simulink model "FeedBack_Linearization"  (R2021b)
settings: Solver=VariableStepAuto  StartTime=0.0  StopTime=10.0  RelTol=1e-3
undefined symbols (not defined in the file): Kd, Kp, q_dq_init
(part 4 of 9)

== matlab function FeedBack_Linearization/C ==
  data: q input; C output; dq input
function C = C_fun(q,dq)
%C_fun
%    C = C_fun(Q1,Q2,Q3,Q4,Q5,Q6,Q7,DQ1,DQ2,DQ3,DQ4,DQ5,DQ6,DQ7)

%    This function was generated by the Symbolic Math Toolbox version 9.0.
%    15-Apr-2022 03:00:29

q1 = q(1);
q2 = q(2);
q3 = q(3);
q4 = q(4);
q5 = q(5);
q6 = q(6);
q7 = q(7);

dq1 = dq(1);
dq2 = dq(2);
dq3 = dq(3);
dq4 = dq(4);
dq5 = dq(5);
dq6 = dq(6);
dq7 = dq(7);

t2 = cos(q1);
t3 = cos(q2);
t4 = cos(q3);
t5 = cos(q4);
t6 = cos(q5);
t7 = cos(q6);
t8 = cos(q7);
t9 = sin(q1);
t10 = sin(q2);
t11 = sin(q3);
t12 = sin(q4);
t13 = sin(q5);
t14 = sin(q6);
t15 = sin(q7);
t16 = dq1.^2;
t17 = dq2.^2;
t18 = dq3.^2;
t19 = dq4.^2;
t20 = dq5.^2;
t21 = dq6.^2;
t22 = dq7.^2;
t1002 = atan(4.601355810186573e-2);
t1005 = atan(4.558404558404559e-1);
t1006 = atan(2.19375);
t23 = t2.^2;
t24 = t3.^2;
t25 = t4.^2;
t26 = t9.^2;
t27 = t10.^2;
t28 = t11.^2;
t29 = t2.*t4;
t30 = t3.*t5;
t31 = t2.*t11;
t32 = t4.*t9;
t33 = t3.*t12;
t34 = t5.*t10;
t35 = t9.*t11;
t36 = t10.*t12;
t37 = dq1.*t2.*t3;
t39 = dq2.*t2.*t3;
t40 = dq2.*t3.*t4;
t43 = dq3.*t3.*t4;
t45 = dq1.*t2.*t10;
t46 = dq1.*t3.*t9;
t49 = dq2.*t2.*t10;
t50 = dq2.*t3.*t9;
t51 = dq2.*t3.*t11;
t52 = dq2.*t4.*t10;
t57 = dq3.*t3.*t11;
t58 = dq3.*t4.*t10;
t61 = dq1.*t9.*t10;
t63 = dq2.*t9.*t10;
t64 = dq2.*t10.*t11;
t67 = dq3.*t10.*t11;
t71 = t10.*t11.*t13;
t72 = dq2.*t3.*t10.*2.0;
t83 = t3.*t6.*t11;
t84 = t4.*t6.*t10;
t90 = t3.*t11.*t13;
t91 = t4.*t10.*t13;
t92 = t6.*t10.*t11;
t105 = t10.*(2.1e+1./5.0e+1);
t192 = t2.*t3.*t16;
t194 = t2.*t3.*t17;
t202 = t2.*t10.*t16;
t203 = t3.*t9.*t16;
t206 = t2.*t10.*t17;
t207 = t3.*t9.*t17;
t209 = t4.*t10.*t17;
t213 = t4.*t10.*t18;
t221 = t9.*t10.*t16;
t223 = t9.*t10.*t17;
t224 = t10.*t11.*t17;
t226 = t10.*t11.*t18;
t248 = t3.*t10.*t17.*2.0;
t267 = t2.*t3.*(2.1e+1./5.0e+1);
t272 = t3.*t9.*(2.1e+1./5.0e+1);
t358 = dq2.*t10.*(-2.1e+1./5.0e+1);
t496 = t3.*t17.*(2.1e+1./5.0e+1);
t1021 = q2+t1002;
t1026 = q1+t1006;
t1037 = -t1005;
t1107 = t2.*t16.*3.55e-3;
t1108 = t9.*t16.*3.55e-3;
t1403 = t3.*t17.*3.9348e-1;
t1717 = dq2.*t3.*t10.*2.32304589786736e-19;
t1723 = dq2.*t3.*t10.*1.781996172844913e-20;
t2010 = dq2.*t3.*t10.*8.400000000000278e-4;
t38 = dq1.*t29;
t41 = dq3.*t29;
t42 = dq2.*t30;
t44 = dq4.*t30;
t47 = dq1.*t31;
t48 = dq1.*t32;
t53 = dq3.*t31;
t54 = dq3.*t32;
t55 = dq2.*t33;
t56 = dq2.*t34;
t59 = dq4.*t33;
t60 = dq4.*t34;
t62 = dq1.*t35;
t65 = dq3.*t35;
t66 = dq2.*t36;
t68 = dq4.*t36;
t69 = dq2.*t24;
t70 = t9.*t36;
t73 = t3.*t29;
t74 = t2.*t30;
t75 = t4.*t30;
t76 = t3.*t31;
t77 = t3.*t32;
t78 = t2.*t33;
t79 = t2.*t34;
t80 = t9.*t30;
t81 = t4.*t33;
t82 = t4.*t34;
t85 = t3.*t35;
t86 = t2.*t36;
t87 = t9.*t33;
t88 = t9.*t34;
t89 = t4.*t36;
t93 = t33.*(2.0./5.0);
t94 = t34.*(2.0./5.0);
t102 = t6.*t40;
t103 = t6.*t43;
t113 = dq2.*t10.*t29;
t127 = t13.*t40;
t128 = t6.*t51;
t129 = dq3.*t11.*t30;
t131 = t13.*t43;
t132 = t6.*t58;
t135 = dq5.*t83;
t136 = dq5.*t84;
t143 = dq2.*t10.*t31;
t145 = dq2.*t10.*t32;
t157 = t13.*t51;
t158 = t6.*t64;
t159 = dq3.*t11.*t33;
t161 = dq3.*t11.*t34;
t162 = t13.*t58;
t163 = t6.*t67;
t166 = dq5.*t90;
t167 = dq5.*t91;
t168 = dq5.*t92;
t173 = dq2.*t10.*t35;
t177 = t13.*t64;
t178 = dq3.*t11.*t36;
t179 = t13.*t67;
t181 = dq5.*t71;
t182 = -t72;
t185 = -t61;
t186 = -t63;
t187 = -t64;
t189 = -t67;
t191 = dq1.*t3.*t23;
t193 = t16.*t29;
t195 = t18.*t29;
t196 = t17.*t30;
t197 = t19.*t30;
t198 = dq2.*t37.*2.0;
t200 = dq3.*t40.*2.0;
t201 = dq1.*t3.*t26;
t204 = t16.*t31;
t205 = t16.*t32;
t208 = dq2.*t4.*t27;
t210 = t18.*t31;
t211 = t18.*t32;
t212 = t17.*t33;
t214 = t19.*t33;
t215 = dq2.*t45.*2.0;
t216 = dq2.*t46.*2.0;
t219 = dq3.*t51.*2.0;
t222 = t16.*t35;
t225 = t18.*t35;
t227 = dq2.*t61.*2.0;
t231 = dq1.*dq2.*t10.*t23;
t232 = dq1.*dq2.*t10.*t26;
t233 = dq2.*dq3.*t11.*t27;
t234 = t10.*t40.*2.0;
t239 = dq2.*t105;
t240 = t29.*t34;
t241 = t29.*t36;
t242 = t32.*t34;
t243 = t6.*t10.*t31;
t244 = t6.*t11.*t34;
t250 = t32.*t36;
t251 = t10.*t13.*t31;
t252 = t6.*t10.*t35;
t253 = t11.*t13.*t34;
t254 = t7.*t11.*t36;
t258 = t10.*t13.*t35;
t259 = t11.*t14.*t36;
t265 = -t90;
t266 = -t92;
t269 = t11.*t36.*(2.0./5.0);
t271 = t2.*t105;
t281 = t9.*t105;
t395 = t17.*t92;
t397 = t18.*t92;
t399 = t20.*t92;
t418 = t17.*t71;
t419 = t18.*t71;
t420 = t20.*t71;
t459 = t37.*(2.1e+1./5.0e+1);
t460 = t39.*(2.1e+1./5.0e+1);
t464 = t45.*(2.1e+1./5.0e+1);
t465 = t46.*(2.1e+1./5.0e+1);
t466 = t49.*(2.1e+1./5.0e+1);
t467 = t50.*(2.1e+1./5.0e+1);
t468 = t61.*(2.1e+1./5.0e+1);
t469 = t63.*(2.1e+1./5.0e+1);
t475 = t3.*t209.*2.0;
t554 = dq2.*t37.*(2.1e+1./2.5e+1);
t557 = dq2.*t46.*(2.1e+1./2.5e+1);
t558 = -t496;
t567 = t45+t50;
t568 = t46+t49;
t569 = t51+t58;
t570 = t52+t57;
t1058 = q1+t1037;
t1171 = -t1108;
t1192 = dq2.*t37.*3.3338e-1;
t1196 = dq2.*t46.*3.3338e-1;
t1235 = dq3.*t51.*4.5e-3;
t1251 = t202.*1.6669e-1;
t1252 = t206.*1.6669e-1;
t1254 = t221.*1.6669e-1;
t1255 = t223.*1.6669e-1;
t1261 = dq3.*t40.*7.635999999999999e-2;
t1262 = dq3.*t40.*6.984e-2;
t1279 = t209.*2.25e-3;
t1281 = t213.*2.25e-3;
t1282 = dq2.*t45.*1.534e-2;
t1285 = dq2.*t61.*1.534e-2;
t1323 = t224.*3.492e-2;
t1324 = t226.*3.492e-2;
t1396 = t224.*3.818e-2;
t1397 = t226.*3.818e-2;
t1404 = t192.*7.669999999999999e-3;
t1405 = t194.*7.669999999999999e-3;
t1407 = t203.*7.669999999999999e-3;
t1408 = t207.*7.669999999999999e-3;
t1457 = dq2.*t37.*7.8696e-1;
t1461 = dq2.*t46.*7.8696e-1;
t1533 = t202.*3.9348e-1;
t1534 = t206.*3.9348e-1;
t1535 = t221.*3.9348e-1;
t1536 = t223.*3.9348e-1;
t1736 = -t1717;
t1751 = -t1723;
t1980 = t10.*t40.*1.400000000000004e-4;
t2007 = t3.*t209.*1.400000000000004e-4;
t2009 = t10.*t40.*9.999999999999995e-5;
t2018 = -t2010;
t2023 = t3.*t209.*9.999999999999995e-5;
t2048 = t10.*t40.*4.380000000000001e-3;
t2097 = t3.*t209.*4.380000000000001e-3;
t95 = t3.*t38;
t96 = dq1.*t74;
t97 = dq2.*t73;
t98 = t2.*t42;
t99 = t3.*t41;
t100 = t4.*t42;
t101 = t2.*t44;
t104 = t4.*t44;
t106 = t3.*t47;
t107 = t10.*t38;
t108 = t3.*t48;
t109 = dq1.*t78;
t110 = dq1.*t79;
t111 = dq1.*t80;
t112 = dq2.*t76;
t114 = dq2.*t77;
t115 = t2.*t55;
t116 = t2.*t56;
t117 = t9.*t42;
t118 = t3.*t53;
t119 = t10.*t41;
t120 = t3.*t54;
t121 = t4.*t55;
t122 = t11.*t42;
t123 = t4.*t56;
t124 = t2.*t59;
t125 = t2.*t60;
t126 = t9.*t44;
t130 = dq3.*t82;
t133 = t4.*t59;
t134 = t4.*t60;
t137 = t10.*t47;
t138 = t3.*t62;
t139 = t10.*t48;
t140 = dq1.*t86;
t141 = dq1.*t87;
t142 = dq1.*t88;
t144 = dq2.*t85;
t146 = t2.*t66;
t147 = t9.*t55;
t148 = t9.*t56;
t149 = t10.*t53;
t150 = t3.*t65;
t151 = t10.*t54;
t152 = t11.*t55;
t153 = t4.*t66;
t154 = t2.*t68;
t155 = t9.*t59;
t156 = t9.*t60;
t160 = dq3.*t89;
t164 = t4.*t68;
t165 = t11.*t60;
t169 = -t38;
t170 = -t41;
t171 = t10.*t62;
t172 = dq1.*t70;
t174 = t9.*t66;
t175 = t10.*t65;
t176 = t9.*t68;
t180 = t11.*t68;
t183 = -t55;
t184 = -t60;
t188 = -t66;
t190 = -t68;
t199 = dq3.*t38.*2.0;
t217 = dq3.*t47.*2.0;
t218 = dq3.*t48.*2.0;
t220 = dq4.*t56.*2.0;
t228 = dq3.*t62.*2.0;
t229 = dq4.*t66.*2.0;
t230 = -t93;
t235 = t44.*(2.0./5.0);
t236 = t56.*(2.0./5.0);
t237 = t59.*(2.0./5.0);
t238 = t66.*(2.0./5.0);
t245 = -t198;
t247 = -t200;
t249 = -t73;
t256 = -t81;
t257 = -t82;
t260 = -t227;
t262 = -t85;
t263 = -t86;
t264 = -t88;
t268 = t70.*(2.0./5.0);
t270 = t29.*t42;
t273 = t34.*t38;
t274 = t29.*t55;
t275 = t32.*t42;
t278 = t29.*t60;
t282 = t36.*t38;
t283 = t34.*t48;
t285 = t32.*t55;
t288 = t34.*t53;
t291 = t29.*t68;
t292 = t32.*t60;
t294 = dq5.*t243;
t299 = dq5.*t244;
t304 = -t102;
t305 = -t103;
t307 = t36.*t48;
t311 = t36.*t53;
t312 = t34.*t65;
t314 = t32.*t68;
t315 = dq5.*t251;
t316 = dq5.*t252;
t321 = dq5.*t253;
t322 = dq6.*t254;
t324 = -t128;
t325 = -t132;
t328 = t36.*t65;
t329 = dq5.*t258;
t331 = dq6.*t259;
t340 = -t173;
t344 = -t177;
t345 = -t179;
t350 = t16.*t73;
t351 = t17.*t73;
t352 = t18.*t73;
t356 = dq3.*t102.*2.0;
t359 = t16.*t76;
t360 = t16.*t77;
t361 = t16.*t79;
t362 = t17.*t76;
t363 = t17.*t77;
t364 = t17.*t79;
t365 = t18.*t76;
t366 = t18.*t77;
t367 = t17.*t82;
t368 = t19.*t79;
t369 = t18.*t82;
t370 = t19.*t82;
t381 = dq3.*t127.*2.0;
t383 = dq5.*t128.*2.0;
t384 = dq5.*t132.*2.0;
t385 = t16.*t85;
t386 = t16.*t86;
t387 = t16.*t88;
t388 = t17.*t85;
t389 = t17.*t86;
t390 = t17.*t88;
t391 = t18.*t85;
t392 = t17.*t89;
t393 = t19.*t86;
t394 = t19.*t88;
t396 = t18.*t89;
t398 = t19.*t89;
t411 = dq5.*t157.*2.0;
t412 = dq5.*t162.*2.0;
t413 = -t193;
t414 = -t195;
t415 = t16.*t70;
t416 = t17.*t70;
t417 = t19.*t70;
t425 = -t212;
t426 = -t214;
t427 = t74.*(2.0./5.0);
t428 = t79.*(2.0./5.0);
t429 = t80.*(2.0./5.0);
t430 = t81.*(2.0./5.0);
t431 = t82.*(2.0./5.0);
t432 = dq4.*t66.*(4.0./5.0);
t433 = t86.*(2.0./5.0);
t434 = t88.*(2.0./5.0);
t456 = dq3.*t11.*t94;
t463 = t178.*(2.0./5.0);
t482 = -t240;
t483 = t196.*(2.0./5.0);
t484 = t197.*(2.0./5.0);
t485 = -t242;
t486 = -t243;
t491 = -t252;
t492 = -t253;
t493 = -t254;
t530 = -t459;
t531 = -t460;
t535 = -t465;
t536 = -t466;
t537 = -t468;
t538 = -t469;
t544 = -t475;
t553 = t241.*(2.0./5.0);
t556 = t250.*(2.0./5.0);
t571 = t31+t77;
t572 = t32+t76;
t573 = t30+t89;
t574 = t36+t75;
t588 = -t554;
t590 = t16.*t271;
t591 = t17.*t271;
t592 = t16.*t281;
t593 = t17.*t281;
t600 = t37+t186;
t601 = t39+t185;
t602 = t40+t189;
t603 = t43+t187;
t610 = t2.*t567;
t611 = t3.*t569;
t622 = dq1.*t9.*t567;
t623 = dq2.*t10.*t569;
t624 = t191+t201;
t632 = t74+t241;
t633 = t80+t250;
t634 = t91+t244;
t645 = t2.*t10.*t568;
t688 = t39.*t568;
t701 = t61.*t568;
t702 = t231+t232;
t823 = t202+t206+t216;
t824 = t203+t207+t215;
t825 = t209+t213+t219;
t1086 = t56.*1.8866e-1;
t1087 = t59.*1.8866e-1;
t1095 = dq4.*t66.*3.7732e-1;
t1105 = t196.*1.8866e-1;
t1106 = t197.*1.8866e-1;
t1157 = t178.*1.8866e-1;
t1189 = t163.*2.37e-3;
t1190 = t167.*2.37e-3;
t1193 = t181.*2.37e-3;
t1233 = dq3.*t38.*4.5e-3;
t1234 = dq3.*t48.*4.5e-3;
t1236 = t102.*2.37e-3;
t1240 = t128.*2.37e-3;
t1241 = t132.*2.37e-3;
t1245 = t38.*3.818e-2;
t1247 = dq4.*t66.*1.0536e-1;
t1248 = -t1192;
t1249 = t48.*3.818e-2;
t1250 = t53.*3.818e-2;
t1253 = t65.*3.818e-2;
t1257 = dq3.*t102.*4.74e-3;
t1258 = t102.*2.75e-2;
t1259 = dq5.*t157.*4.74e-3;
t1260 = dq5.*t162.*4.74e-3;
t1263 = t128.*2.75e-2;
t1264 = t132.*2.75e-2;
t1265 = dq3.*t47.*7.635999999999999e-2;
t1266 = dq3.*t47.*6.984e-2;
t1267 = t163.*2.75e-2;
t1268 = t167.*2.75e-2;
t1270 = dq3.*t62.*7.635999999999999e-2;
t1271 = dq3.*t62.*6.984e-2;
C = ft_1({dq1,dq2,dq3,dq4,dq5,dq6,dq7,t10,t100,t101,t102,t1021,t1026,t104,t105,t1058,t106,t107,t108,t1086,t1087,t109,t1095,t11,t110,t1105,t1106,t1107,t111,t112,t113,t114,t115,t1157,t116,t117,t1171,t118,t1189,t119,t1190,t1193,t1196,t12,t120,t121,t122,t123,t1233,t1234,t1235,t1236,t124,t1240,t1241,t1245,t1247,t1248,t1249,t125,t1250,t1251,t1252,t1253,t1254,t1255,t1257,t1258,t1259,t126,t1260,t1261,t1262,t1263,t1264,t1265,t1266,t1267,t1268,t127,t1270,t1271,t1279,t128,t1281,t1282,t1285,t129,t13,t130,t131,t132,t1323,t1324,t133,t134,t135,t136,t137,t138,t139,t1396,t1397,t14,t140,t1403,t1404,t1405,t1407,t1408,t141,t142,t143,t144,t145,t1457,t146,t1461,t147,t148,t149,t15,t150,t151,t152,t153,t1533,t1534,t1535,t1536,t154,t155,t156,t157,t158,t159,t16,t160,t161,t162,t163,t164,t165,t166,t167,t168,t169,t17,t170,t171,t1717,t172,t1723,t173,t1736,t174,t175,t1751,t176,t178,t179,t18,t180,t181,t182,t183,t184,t185,t186,t187,t188,t189,t19,t190,t191,t192,t193,t194,t195,t196,t197,t1980,t199,t2,t20,t2007,t2009,t201,t2010,t2018,t2023,t204,t2048,t205,t208,t2097,t21,t210,t211,t212,t214,t217,t218,t22,t220,t221,t222,t223,t224,t225,t226,t228,t229,t23,t230,t231,t232,t233,t234,t235,t236,t237,t238,t239,t24,t240,t241,t242,t243,t244,t245,t247,t248,t249,t25,t250,t251,t252,t253,t254,t256,t257,t258,t259,t26,t260,t262,t263,t264,t265,t266,t267,t268,t269,t27,t270,t271,t272,t273,t274,t275,t278,t28,t281,t282,t283,t285,t288,t29,t291,t292,t294,t299,t3,t30,t304,t305,t307,t31,t311,t312,t314,t315,t316,t32,t321,t322,t324,t325,t328,t329,t33,t331,t34,t340,t344,t345,t35,t350,t351,t352,t356,t358,t359,t36,t360,t361,t362,t363,t364,t365,t366,t367,t368,t369,t37,t370,t381,t383,t384,t385,t386,t387,t388,t389,t39,t390,t391,t392,t393,t394,t395,t396,t397,t398,t399,t4,t40,t411,t412,t413,t414,t415,t416,t417,t418,t419,t42,t420,t425,t426,t427,t428,t429,t43,t430,t431,t432,t433,t434,t44,t45,t456,t459,t46,t460,t463,t464,t465,t466,t467,t468,t469,t47,t48,t482,t483,t484,t485,t486,t49,t491,t492,t493,t496,t5,t50,t51,t53,t530,t531,t535,t536,t537,t538,t54,t544,t55,t553,t554,t556,t557,t558,t56,t567,t568,t569,t57,t570,t571,t572,t573,t574,t58,t588,t59,t590,t591,t592,t593,t6,t600,t601,t602,t603,t61,t610,t611,t62,t622,t623,t624,t63,t632,t633,t634,t64,t645,t65,t67,t688,t69,t7,t70,t701,t702,t71,t72,t73,t74,t75,t76,t77,t78,t79,t8,t80,t81,t82,t823,t824,t825,t83,t84,t85,t86,t87,t88,t89,t9,t90,t91,t92,t94,t95,t96,t97,t98,t99});
end
function C = ft_1(ct)
dq1 = ct{1};
dq2 = ct{2};
dq3 = ct{3};
dq4 = ct{4};
dq5 = ct{5};
dq6 = ct{6};
dq7 = ct{7};
t10 = ct{8};
t100 = ct{9};
t101 = ct{10};
t102 = ct{11};
t1021 = ct{12};
t1026 = ct{13};
t104 = ct{14};
t105 = ct{15};
t1058 = ct{16};
t106 = ct{17};
t107 = ct{18};
t108 = ct{19};
t1086 = ct{20};
t1087 = ct{21};
t109 = ct{22};
t1095 = ct{23};
t11 = ct{24};
t110 = ct{25};
t1105 = ct{26};
t1106 = ct{27};
t1107 = ct{28};
t111 = ct{29};
t112 = ct{30};
t113 = ct{31};
t114 = ct{32};
t115 = ct{33};
t1157 = ct{34};
t116 = ct{35};
t117 = ct{36};
t1171 = ct{37};
t118 = ct{38};
t1189 = ct{39};
t119 = ct{40};
t1190 = ct{41};
t1193 = ct{42};
t1196 = ct{43};
t12 = ct{44};
t120 = ct{45};
t121 = ct{46};
t122 = ct{47};
t123 = ct{48};
t1233 = ct{49};
t1234 = ct{50};
t1235 = ct{51};
t1236 = ct{52};
t124 = ct{53};
t1240 = ct{54};
t1241 = ct{55};
t1245 = ct{56};
t1247 = ct{57};
t1248 = ct{58};
t1249 = ct{59};
t125 = ct{60};
t1250 = ct{61};
t1251 = ct{62};
t1252 = ct{63};
t1253 = ct{64};
t1254 = ct{65};
t1255 = ct{66};
t1257 = ct{67};
t1258 = ct{68};
t1259 = ct{69};
t126 = ct{70};
t1260 = ct{71};
t1261 = ct{72};
t1262 = ct{73};
t1263 = ct{74};
t1264 = ct{75};
t1265 = ct{76};
t1266 = ct{77};
t1267 = ct{78};
t1268 = ct{79};
t127 = ct{80};
t1270 = ct{81};
t1271 = ct{82};
t1279 = ct{83};
t128 = ct{84};
t1281 = ct{85};
t1282 = ct{86};
t1285 = ct{87};
t129 = ct{88};
t13 = ct{89};
t130 = ct{90};
t131 = ct{91};
t132 = ct{92};
t1323 = ct{93};
t1324 = ct{94};
t133 = ct{95};
t134 = ct{96};
t135 = ct{97};
t136 = ct{98};
t137 = ct{99};
t138 = ct{100};
t139 = ct{101};
t1396 = ct{102};
t1397 = ct{103};
t14 = ct{104};
t140 = ct{105};
t1403 = ct{106};
t1404 = ct{107};
t1405 = ct{108};
t1407 = ct{109};
t1408 = ct{110};
t141 = ct{111};
t142 = ct{112};
t143 = ct{113};
t144 = ct{114};
t145 = ct{115};
t1457 = ct{116};
t146 = ct{117};
t1461 = ct{118};
t147 = ct{119};
t148 = ct{120};
t149 = ct{121};
t15 = ct{122};
t150 = ct{123};
t151 = ct{124};
t152 = ct{125};
t153 = ct{126};
t1533 = ct{127};
t1534 = ct{128};
t1535 = ct{129};
t1536 = ct{130};
t154 = ct{131};
t155 = ct{132};
t156 = ct{133};
t157 = ct{134};
t158 = ct{135};
t159 = ct{136};
t16 = ct{137};
t160 = ct{138};
t161 = ct{139};
t162 = ct{140};
t163 = ct{141};
t164 = ct{142};
t165 = ct{143};
t166 = ct{144};
t167 = ct{145};
t168 = ct{146};
t169 = ct{147};
t17 = ct{148};
t170 = ct{149};
t171 = ct{150};
t1717 = ct{151};
t172 = ct{152};
t1723 = ct{153};
t173 = ct{154};
t1736 = ct{155};
t174 = ct{156};
t175 = ct{157};
t1751 = ct{158};
t176 = ct{159};
t178 = ct{160};
t179 = ct{161};
t18 = ct{162};
t180 = ct{163};
t181 = ct{164};
t182 = ct{165};
t183 = ct{166};
t184 = ct{167};
t185 = ct{168};
t186 = ct{169};
t187 = ct{170};
t188 = ct{171};
t189 = ct{172};
t19 = ct{173};
t190 = ct{174};
t191 = ct{175};
t192 = ct{176};
t193 = ct{177};
t194 = ct{178};
t195 = ct{179};
t196 = ct{180};
t197 = ct{181};
t1980 = ct{182};
t199 = ct{183};
t2 = ct{184};
t20 = ct{185};
t2007 = ct{186};
t2009 = ct{187};
t201 = ct{188};
t2010 = ct{189};
t2018 = ct{190};
t2023 = ct{191};
t204 = ct{192};
t2048 = ct{193};
t205 = ct{194};
t208 = ct{195};
t2097 = ct{196};
t21 = ct{197};
t210 = ct{198};
t211 = ct{199};
t212 = ct{200};
t214 = ct{201};
t217 = ct{202};
t218 = ct{203};
t22 = ct{204};
t220 = ct{205};
t221 = ct{206};
t222 = ct{207};
t223 = ct{208};
t224 = ct{209};
t225 = ct{210};
t226 = ct{211};
t228 = ct{212};
t229 = ct{213};
t23 = ct{214};
t230 = ct{215};
t231 = ct{216};
t232 = ct{217};
t233 = ct{218};
t234 = ct{219};
t235 = ct{220};
t236 = ct{221};
t237 = ct{222};
t238 = ct{223};
t239 = ct{224};
t24 = ct{225};
t240 = ct{226};
t241 = ct{227};
t242 = ct{228};
t243 = ct{229};
t244 = ct{230};
t245 = ct{231};
t247 = ct{232};
t248 = ct{233};
t249 = ct{234};
t25 = ct{235};
t250 = ct{236};
t251 = ct{237};
t252 = ct{238};
t253 = ct{239};
t254 = ct{240};
t256 = ct{241};
t257 = ct{242};
t258 = ct{243};
t259 = ct{244};
t26 = ct{245};
t260 = ct{246};
t262 = ct{247};
t263 = ct{248};
t264 = ct{249};
t265 = ct{250};
t266 = ct{251};
t267 = ct{252};
t268 = ct{253};
t269 = ct{254};
t27 = ct{255};
t270 = ct{256};
t271 = ct{257};
t272 = ct{258};
t273 = ct{259};
t274 = ct{260};
t275 = ct{261};
t278 = ct{262};
t28 = ct{263};
t281 = ct{264};
t282 = ct{265};
t283 = ct{266};
t285 = ct{267};
t288 = ct{268};
t29 = ct{269};
t291 = ct{270};
t292 = ct{271};
t294 = ct{272};
t299 = ct{273};
t3 = ct{274};
t30 = ct{275};
t304 = ct{276};
t305 = ct{277};
t307 = ct{278};
t31 = ct{279};
t311 = ct{280};
t312 = ct{281};
t314 = ct{282};
t315 = ct{283};
t316 = ct{284};
t32 = ct{285};
t321 = ct{286};
t322 = ct{287};
t324 = ct{288};
t325 = ct{289};
t328 = ct{290};
t329 = ct{291};
t33 = ct{292};
t331 = ct{293};
t34 = ct{294};
t340 = ct{295};
t344 = ct{296};
t345 = ct{297};
t35 = ct{298};
t350 = ct{299};
t351 = ct{300};
t352 = ct{301};
t356 = ct{302};
t358 = ct{303};
t359 = ct{304};
t36 = ct{305};
t360 = ct{306};
t361 = ct{307};
t362 = ct{308};
t363 = ct{309};
t364 = ct{310};
t365 = ct{311};
t366 = ct{312};
t367 = ct{313};
t368 = ct{314};
t369 = ct{315};
t37 = ct{316};
t370 = ct{317};
t381 = ct{318};
t383 = ct{319};
t384 = ct{320};
t385 = ct{321};
t386 = ct{322};
t387 = ct{323};
t388 = ct{324};
t389 = ct{325};
t39 = ct{326};
t390 = ct{327};
t391 = ct{328};
t392 = ct{329};
t393 = ct{330};
t394 = ct{331};
t395 = ct{332};
t396 = ct{333};
t397 = ct{334};
t398 = ct{335};
t399 = ct{336};
t4 = ct{337};
t40 = ct{338};
t411 = ct{339};
t412 = ct{340};
t413 = ct{341};
t414 = ct{342};
t415 = ct{343};
t416 = ct{344};
t417 = ct{345};
t418 = ct{346};
t419 = ct{347};
t42 = ct{348};
t420 = ct{349};
t425 = ct{350};
t426 = ct{351};
t427 = ct{352};
t428 = ct{353};
t429 = ct{354};
t43 = ct{355};
t430 = ct{356};
t431 = ct{357};
t432 = ct{358};
t433 = ct{359};
t434 = ct{360};
t44 = ct{361};
t45 = ct{362};
t456 = ct{363};
t459 = ct{364};
t46 = ct{365};
t460 = ct{366};
t463 = ct{367};
t464 = ct{368};
t465 = ct{369};
t466 = ct{370};
t467 = ct{371};
t468 = ct{372};
t469 = ct{373};
t47 = ct{374};
t48 = ct{375};
t482 = ct{376};
t483 = ct{377};
t484 = ct{378};
t485 = ct{379};
t486 = ct{380};
t49 = ct{381};
t491 = ct{382};
t492 = ct{383};
t493 = ct{384};
t496 = ct{385};
t5 = ct{386};
t50 = ct{387};
t51 = ct{388};
t53 = ct{389};
t530 = ct{390};
t531 = ct{391};
t535 = ct{392};
t536 = ct{393};
t537 = ct{394};
t538 = ct{395};
t54 = ct{396};
t544 = ct{397};
t55 = ct{398};
t553 = ct{399};
t554 = ct{400};
t556 = ct{401};
t557 = ct{402};
t558 = ct{403};
t56 = ct{404};
t567 = ct{405};
t568 = ct{406};
t569 = ct{407};
t57 = ct{408};
t570 = ct{409};
t571 = ct{410};
t572 = ct{411};
t573 = ct{412};
t574 = ct{413};
t58 = ct{414};
t588 = ct{415};
t59 = ct{416};
t590 = ct{417};
t591 = ct{418};
t592 = ct{419};
t593 = ct{420};
t6 = ct{421};
t600 = ct{422};
t601 = ct{423};
t602 = ct{424};
t603 = ct{425};
t61 = ct{426};
t610 = ct{427};
t611 = ct{428};
t62 = ct{429};
t622 = ct{430};
t623 = ct{431};
t624 = ct{432};
t63 = ct{433};
t632 = ct{434};
t633 = ct{435};
t634 = ct{436};
t64 = ct{437};
t645 = ct{438};
t65 = ct{439};
t67 = ct{440};
t688 = ct{441};
t69 = ct{442};
t7 = ct{443};
t70 = ct{444};
t701 = ct{445};
t702 = ct{446};
t71 = ct{447};
t72 = ct{448};
t73 = ct{449};
t74 = ct{450};
t75 = ct{451};
t76 = ct{452};
t77 = ct{453};
t78 = ct{454};
t79 = ct{455};
t8 = ct{456};
t80 = ct{457};
t81 = ct{458};
t82 = ct{459};
t823 = ct{460};
t824 = ct{461};
t825 = ct{462};
t83 = ct{463};
t84 = ct{464};
t85 = ct{465};
t86 = ct{466};
t87 = ct{467};
t88 = ct{468};
t89 = ct{469};
t9 = ct{470};
t90 = ct{471};
t91 = ct{472};
t92 = ct{473};
t94 = ct{474};
t95 = ct{475};
t96 = ct{476};
t97 = ct{477};
t98 = ct{478};
t99 = ct{479};
t1272 = t181.*2.75e-2;
t1278 = t204.*2.25e-3;
t1280 = t210.*2.25e-3;
t1283 = t222.*2.25e-3;
t1284 = t225.*2.25e-3;
t1301 = t395.*2.37e-3;
t1302 = t397.*2.37e-3;
t1303 = t399.*2.37e-3;
t1307 = t193.*3.492e-2;
t1308 = t195.*3.492e-2;
t1310 = -t1261;
t1316 = t205.*3.492e-2;
t1317 = t211.*3.492e-2;
t1337 = dq3.*t102.*5.5e-2;
t1338 = -t1285;
t1341 = dq5.*t157.*5.5e-2;
t1342 = dq5.*t162.*5.5e-2;
t1343 = t196.*5.267999999999999e-2;
t1344 = t197.*5.267999999999999e-2;
t1349 = t143.*3.818e-2;
t1353 = t173.*3.818e-2;
t1368 = t127.*5.000000000000001e-5;
t1369 = t136.*5.000000000000001e-5;
t1371 = t193.*3.818e-2;
t1372 = t195.*3.818e-2;
t1373 = dq4.*t56.*4.0e-4;
t1380 = t157.*5.000000000000001e-5;
t1381 = t162.*5.000000000000001e-5;
t1382 = t168.*5.000000000000001e-5;
t1384 = t205.*3.818e-2;
t1385 = t211.*3.818e-2;
t1392 = t179.*5.000000000000001e-5;
t1398 = -t1323;
t1399 = -t1324;
t1416 = t395.*2.75e-2;
t1417 = t397.*2.75e-2;
t1418 = t399.*2.75e-2;
t1447 = t212.*2.0e-4;
t1448 = t214.*2.0e-4;
t1464 = dq3.*t127.*1.0e-4;
t1465 = dq5.*t128.*1.0e-4;
t1466 = dq5.*t132.*1.0e-4;
t1550 = t418.*5.000000000000001e-5;
t1551 = t419.*5.000000000000001e-5;
t1552 = t420.*5.000000000000001e-5;
t1575 = -t1535;
t1576 = -t1536;
t1708 = t69.*1.16152294893368e-19;
t1739 = t69.*8.909980864224564e-21;
t1747 = t201.*1.16152294893368e-19;
t1768 = t191.*1.16152294893368e-19;
t1788 = t191.*5.582083966615414e-19;
t1789 = t201.*5.582083966615414e-19;
t1983 = t208.*7.000000000000022e-5;
t1990 = t233.*7.000000000000022e-5;
t2003 = t208.*4.999999999999997e-5;
t2004 = t69.*4.200000000000139e-4;
t2015 = -t2007;
t2017 = t233.*4.999999999999997e-5;
t2027 = t191.*1.0e-4;
t2031 = t201.*1.0e-4;
t2037 = t208.*2.19e-3;
t2059 = t233.*2.19e-3;
t2060 = -t2048;
t2121 = -t2097;
t246 = -t199;
t255 = -t220;
t261 = -t229;
t276 = t6.*t112;
t277 = t6.*t119;
t279 = t6.*t122;
t280 = t6.*t130;
t284 = t6.*t137;
t286 = t13.*t112;
t287 = t6.*t144;
t289 = t13.*t119;
t290 = t6.*t151;
t293 = t13.*t122;
t295 = t7.*t152;
t296 = t13.*t130;
t297 = t7.*t160;
t298 = t7.*t165;
t300 = -t95;
t301 = -t97;
t302 = -t99;
t303 = -t100;
t306 = -t104;
t308 = t13.*t137;
t309 = t6.*t171;
t310 = t13.*t144;
t313 = t13.*t151;
t317 = t14.*t152;
t318 = t14.*t160;
t319 = t6.*t180;
t320 = t14.*t165;
t323 = -t121;
t326 = -t134;
t327 = t13.*t171;
t330 = t13.*t180;
t332 = -t141;
t333 = -t142;
t334 = -t146;
t335 = -t148;
t336 = -t154;
t337 = -t155;
t338 = -t171;
t339 = -t172;
t341 = -t174;
t342 = -t175;
t343 = -t176;
t346 = -t180;
t347 = -t236;
t348 = -t237;
t349 = -t238;
t353 = dq1.*t98.*2.0;
t354 = dq3.*t95.*2.0;
t355 = dq4.*t98.*2.0;
t357 = dq4.*t100.*2.0;
t371 = dq2.*t107.*2.0;
t372 = dq1.*t115.*2.0;
t373 = dq1.*t117.*2.0;
t374 = dq3.*t106.*2.0;
t375 = dq3.*t108.*2.0;
t376 = dq2.*t119.*2.0;
t377 = dq1.*t125.*2.0;
t378 = dq4.*t115.*2.0;
t379 = dq4.*t117.*2.0;
t380 = dq3.*t122.*2.0;
t382 = dq4.*t121.*2.0;
t400 = dq2.*t137.*2.0;
t401 = dq2.*t139.*2.0;
t402 = dq1.*t147.*2.0;
t403 = dq3.*t138.*2.0;
t404 = dq2.*t149.*2.0;
t405 = dq2.*t151.*2.0;
t406 = dq1.*t154.*2.0;
t407 = dq1.*t156.*2.0;
t408 = dq4.*t147.*2.0;
t409 = dq3.*t152.*2.0;
t410 = dq3.*t165.*2.0;
t421 = dq2.*t171.*2.0;
t422 = dq2.*t175.*2.0;
t423 = dq1.*t176.*2.0;
t424 = dq3.*t180.*2.0;
t435 = t96.*(2.0./5.0);
t436 = t98.*(2.0./5.0);
t437 = t100.*(2.0./5.0);
t438 = t110.*(2.0./5.0);
t439 = t111.*(2.0./5.0);
t440 = t115.*(2.0./5.0);
t441 = t116.*(2.0./5.0);
t442 = t117.*(2.0./5.0);
t443 = t121.*(2.0./5.0);
t444 = t124.*(2.0./5.0);
t445 = t125.*(2.0./5.0);
t446 = t134.*(2.0./5.0);
t447 = t140.*(2.0./5.0);
t448 = t142.*(2.0./5.0);
t449 = t147.*(2.0./5.0);
t450 = t148.*(2.0./5.0);
t451 = t152.*(2.0./5.0);
t452 = t154.*(2.0./5.0);
t453 = t155.*(2.0./5.0);
t454 = t156.*(2.0./5.0);
t455 = t160.*(2.0./5.0);
t457 = t164.*(2.0./5.0);
t458 = t165.*(2.0./5.0);
t461 = t172.*(2.0./5.0);
t462 = t176.*(2.0./5.0);
t473 = -t356;
t479 = -t381;
t480 = -t383;
t481 = -t384;
t494 = -t430;
t495 = -t432;
t497 = -t270;
t498 = t34.*t169;
t499 = t29.*t183;
t500 = -t275;
t503 = t29.*t184;
t514 = -t321;
t520 = -t328;
t534 = -t463;
t539 = t16.*t249;
t540 = t17.*t249;
t541 = t18.*t249;
t542 = dq1.*t98.*(4.0./5.0);
t543 = dq4.*t100.*(4.0./5.0);
t545 = dq1.*t117.*(4.0./5.0);
t546 = dq4.*t115.*(4.0./5.0);
t547 = dq1.*t154.*(4.0./5.0);
t548 = dq4.*t147.*(4.0./5.0);
t549 = dq3.*t152.*(4.0./5.0);
t550 = dq3.*t165.*(4.0./5.0);
t551 = -t483;
t552 = -t484;
t555 = dq1.*t176.*(4.0./5.0);
t559 = t274.*(2.0./5.0);
t560 = t278.*(2.0./5.0);
t561 = t282.*(2.0./5.0);
t562 = t285.*(2.0./5.0);
t563 = t292.*(2.0./5.0);
t564 = t307.*(2.0./5.0);
t565 = t311.*(2.0./5.0);
t566 = t328.*(2.0./5.0);
t577 = t361.*(2.0./5.0);
t578 = t364.*(2.0./5.0);
t579 = t368.*(2.0./5.0);
t580 = t387.*(2.0./5.0);
t581 = t390.*(2.0./5.0);
t582 = t392.*(2.0./5.0);
t583 = t394.*(2.0./5.0);
t584 = t396.*(2.0./5.0);
t585 = t398.*(2.0./5.0);
t604 = t29+t262;
t605 = t35+t249;
t606 = t33+t257;
t607 = t34+t256;
t608 = t572.^2;
t609 = t573.^2;
t612 = t5.*t571;
t613 = t6.*t571;
t614 = t6.*t572;
t615 = t6.*t574;
t616 = t7.*t573;
t617 = t12.*t571;
t618 = t13.*t571;
t619 = t13.*t572;
t620 = t13.*t574;
t621 = t14.*t573;
t626 = dq4.*t12.*t572;
t629 = dq5.*t13.*t573;
t637 = dq4.*t5.*t572;
t640 = dq5.*t6.*t573;
t647 = t7.*t12.*t572;
t649 = t8.*t13.*t573;
t650 = t12.*t14.*t572;
t651 = t13.*t15.*t573;
t659 = t9.*t601;
t676 = t78+t482;
t677 = t87+t485;
t678 = t84+t492;
t687 = t12.*t572.*(2.0./5.0);
t707 = dq1.*t2.*t601;
t722 = t7.*t632;
t723 = t14.*t632;
t724 = t7.*t633;
t725 = t7.*t634;
t728 = t14.*t633;
t729 = t14.*t634;
t733 = t9.*t10.*t600;
t734 = t10.*t11.*t602;
t761 = -t688;
t769 = t45.*t600;
t770 = t50.*t600;
t771 = t51.*t602;
t772 = t58.*t602;
t818 = t137+t144+t151;
t819 = t152+t160+t165;
t828 = t221+t223+t245;
t829 = t224+t226+t247;
t830 = t192+t194+t260;
t833 = t567.*t571;
t845 = t9.*t823;
t873 = t9.*t10.*t824;
t874 = t10.*t11.*t825;
t1020 = t47+t54+t108+t113+t118;
t1040 = t48+t53+t106+t120+t340;
t1065 = t123+t129+t133+t183+t184;
t1101 = -t1086;
t1102 = -t1087;
t1109 = -t1095;
t1138 = t96.*1.8866e-1;
t1139 = t98.*1.8866e-1;
t1141 = t110.*1.8866e-1;
t1142 = t111.*1.8866e-1;
t1143 = t116.*1.8866e-1;
t1144 = t117.*1.8866e-1;
t1145 = t121.*1.8866e-1;
t1146 = t124.*1.8866e-1;
t1147 = t134.*1.8866e-1;
t1148 = t142.*1.8866e-1;
t1149 = t148.*1.8866e-1;
t1150 = t152.*1.8866e-1;
t1151 = t154.*1.8866e-1;
t1152 = t155.*1.8866e-1;
t1153 = t160.*1.8866e-1;
t1154 = t165.*1.8866e-1;
t1156 = t176.*1.8866e-1;
t1162 = dq1.*t98.*3.7732e-1;
t1163 = dq4.*t100.*3.7732e-1;
t1164 = dq1.*t117.*3.7732e-1;
t1165 = dq4.*t115.*3.7732e-1;
t1166 = dq1.*t154.*3.7732e-1;
t1167 = dq4.*t147.*3.7732e-1;
t1168 = dq3.*t152.*3.7732e-1;
t1169 = dq3.*t165.*3.7732e-1;
t1170 = dq1.*t176.*3.7732e-1;
t1184 = -t1157;
t1197 = t361.*1.8866e-1;
t1198 = t364.*1.8866e-1;
t1199 = t368.*1.8866e-1;
t1200 = t387.*1.8866e-1;
t1201 = t390.*1.8866e-1;
t1202 = t392.*1.8866e-1;
t1203 = t394.*1.8866e-1;
t1204 = t396.*1.8866e-1;
t1205 = t398.*1.8866e-1;
t1230 = t278.*1.8866e-1;
t1232 = t292.*1.8866e-1;
t1276 = -t1233;
t1286 = -t1236;
t1291 = -t1240;
t1292 = -t1241;
t1293 = -t1245;
t1294 = -t1247;
t1299 = t96.*5.267999999999999e-2;
t1300 = t98.*5.267999999999999e-2;
t1304 = -t1258;
t1305 = -t1259;
t1306 = -t1260;
t1311 = t110.*5.267999999999999e-2;
t1312 = t111.*5.267999999999999e-2;
t1313 = t116.*5.267999999999999e-2;
t1314 = t117.*5.267999999999999e-2;
t1315 = t124.*5.267999999999999e-2;
t1319 = t142.*5.267999999999999e-2;
t1320 = t148.*5.267999999999999e-2;
t1321 = t154.*5.267999999999999e-2;
t1322 = t155.*5.267999999999999e-2;
t1326 = -t1271;
t1327 = t176.*5.267999999999999e-2;
t1328 = -t1272;
t1331 = dq2.*t107.*4.5e-3;
t1332 = dq3.*t106.*4.5e-3;
t1333 = dq2.*t139.*4.5e-3;
t1334 = dq3.*t138.*4.5e-3;
t1335 = dq2.*t149.*4.5e-3;
t1336 = dq2.*t175.*4.5e-3;
t1339 = t299.*2.37e-3;
t1340 = t315.*2.37e-3;
t1346 = t329.*2.37e-3;
t1347 = t137.*3.818e-2;
t1348 = t138.*3.818e-2;
t1350 = t144.*3.818e-2;
t1351 = t151.*3.818e-2;
t1352 = t171.*3.818e-2;
t1354 = dq3.*t95.*7.635999999999999e-2;
t1355 = dq3.*t95.*6.984e-2;
t1356 = dq3.*t108.*7.635999999999999e-2;
t1357 = dq2.*t119.*7.635999999999999e-2;
t1358 = dq3.*t108.*6.984e-2;
t1359 = dq2.*t119.*6.984e-2;
t1360 = t299.*2.75e-2;
t1361 = -t1301;
t1362 = -t1302;
t1363 = -t1303;
t1364 = dq2.*t137.*7.635999999999999e-2;
t1365 = dq2.*t151.*7.635999999999999e-2;
t1366 = dq2.*t137.*6.984e-2;
t1367 = dq2.*t151.*6.984e-2;
t1370 = t315.*2.75e-2;
t1378 = dq2.*t171.*7.635999999999999e-2;
t1379 = dq2.*t171.*6.984e-2;
t1383 = t329.*2.75e-2;
t1393 = t350.*2.25e-3;
t1394 = t351.*2.25e-3;
t1395 = t352.*2.25e-3;
t1400 = t360.*2.25e-3;
t1401 = t363.*2.25e-3;
t1402 = t366.*2.25e-3;
t1410 = dq1.*t98.*1.0536e-1;
t1411 = dq4.*t100.*1.0536e-1;
t1412 = -t1337;
t1413 = dq1.*t117.*1.0536e-1;
t1414 = dq4.*t115.*1.0536e-1;
t1415 = t99.*3.818e-2;
t1419 = dq1.*t154.*1.0536e-1;
t1420 = dq4.*t147.*1.0536e-1;
t1421 = dq3.*t152.*1.0536e-1;
t1422 = dq3.*t165.*1.0536e-1;
t1425 = t106.*3.818e-2;
t1426 = t112.*3.818e-2;
t1427 = t119.*3.818e-2;
t1428 = t120.*3.818e-2;
t1429 = dq1.*t176.*1.0536e-1;
t1430 = t172.*2.0e-4;
t1431 = t174.*2.0e-4;
t1432 = -t1353;
t1435 = t322.*4.9e-4;
t1437 = t278.*5.267999999999999e-2;
t1438 = t359.*3.492e-2;
t1439 = t362.*3.492e-2;
t1440 = t365.*3.492e-2;
t1441 = t292.*5.267999999999999e-2;
t1442 = t385.*3.492e-2;
t1443 = t388.*3.492e-2;
t1444 = t391.*3.492e-2;
t1450 = -t1371;
t1451 = -t1372;
t1452 = -t1373;
t1456 = -t1392;
t1467 = t101.*2.0e-4;
t1468 = t361.*5.267999999999999e-2;
t1469 = t364.*5.267999999999999e-2;
t1470 = t368.*5.267999999999999e-2;
t1476 = t109.*2.0e-4;
t1477 = t115.*2.0e-4;
t1478 = t125.*2.0e-4;
t1479 = t126.*2.0e-4;
t1481 = t387.*5.267999999999999e-2;
t1482 = t390.*5.267999999999999e-2;
t1483 = t392.*5.267999999999999e-2;
t1484 = t394.*5.267999999999999e-2;
t1485 = t396.*5.267999999999999e-2;
t1486 = t398.*5.267999999999999e-2;
t1492 = t140.*2.0e-4;
t1493 = t141.*2.0e-4;
t1494 = t146.*2.0e-4;
t1495 = t147.*2.0e-4;
t1496 = t156.*2.0e-4;
t1500 = dq4.*t98.*4.0e-4;
t1501 = dq1.*t115.*4.0e-4;
t1502 = dq1.*t125.*4.0e-4;
t1503 = dq4.*t117.*4.0e-4;
t1504 = dq3.*t122.*4.0e-4;
t1505 = dq4.*t121.*4.0e-4;
t1507 = t294.*5.000000000000001e-5;
t1508 = t359.*3.818e-2;
t1509 = t362.*3.818e-2;
t1510 = t365.*3.818e-2;
t1511 = dq1.*t147.*4.0e-4;
t1512 = dq1.*t156.*4.0e-4;
t1513 = t316.*5.000000000000001e-5;
t1514 = t321.*5.000000000000001e-5;
t1517 = t385.*3.818e-2;
t1518 = t388.*3.818e-2;
t1519 = t391.*3.818e-2;
t1520 = dq3.*t180.*4.0e-4;
t1524 = -t1447;
t1525 = -t1448;
t1537 = -t1464;
t1538 = -t1465;
t1539 = -t1466;
t1555 = t331.*2.019e-2;
t1558 = t367.*2.0e-4;
t1559 = t369.*2.0e-4;
t1560 = t370.*2.0e-4;
t1566 = t386.*2.0e-4;
t1567 = t389.*2.0e-4;
t1568 = t393.*2.0e-4;
t1570 = t415.*2.0e-4;
t1571 = t416.*2.0e-4;
t1572 = t417.*2.0e-4;
t1577 = t291.*2.0e-4;
t1580 = t314.*2.0e-4;
t1648 = t331.*1.9738e-1;
t1895 = t610.*8.909980864224564e-21;
t1904 = t610.*5.582083966615414e-19;
t1916 = t645.*1.16152294893368e-19;
t1926 = t645.*8.909980864224564e-21;
t2030 = -t2017;
t2050 = -t2037;
t2099 = t611.*7.000000000000001e-5;
t2129 = t623.*7.000000000000001e-5;
t2135 = t610.*3.199999999999801e-4;
t2143 = t611.*4.999999999999997e-5;
t2144 = t623.*4.999999999999997e-5;
t2145 = t611.*2.23e-3;
t2162 = t623.*2.23e-3;
t2194 = t645.*4.200000000000139e-4;
t3248 = t1107+t1248+t1254+t1255+t1282+t1407+t1408;
t3249 = t1171+t1196+t1251+t1252+t1338+t1404+t1405;
t3252 = t1235+t1262+t1279+t1281+t1398+t1399+t1403;
t470 = -t353;
t471 = -t354;
t472 = -t355;
t474 = -t357;
t476 = -t372;
t477 = -t377;
t478 = -t379;
t487 = -t421;
t488 = -t422;
t489 = -t423;
t490 = -t424;
t501 = -t276;
t502 = -t277;
t504 = -t284;
t505 = -t287;
t506 = -t290;
t507 = -t295;
t508 = -t297;
t509 = -t298;
t510 = -t435;
t511 = -t436;
t512 = -t437;
t513 = -t319;
t515 = -t440;
t516 = -t443;
t517 = -t445;
C = ft_2({dq1,dq2,dq3,dq4,dq5,dq6,dq7,t10,t101,t1020,t1021,t1026,t1040,t105,t1058,t1065,t107,t109,t11,t110,t1101,t1102,t1105,t1106,t1109,t111,t112,t1138,t1139,t114,t1141,t1142,t1143,t1144,t1145,t1146,t1147,t1148,t1149,t115,t1150,t1151,t1152,t1153,t1154,t1156,t116,t1162,t1163,t1164,t1165,t1166,t1167,t1168,t1169,t117,t1170,t1184,t1189,t119,t1190,t1193,t1197,t1198,t1199,t12,t1200,t1201,t1202,t1203,t1204,t1205,t122,t1230,t1232,t1234,t124,t1249,t125,t1250,t1253,t1257,t126,t1263,t1264,t1265,t1266,t1267,t1268,t127,t1270,t1276,t1278,t1280,t1283,t1284,t1286,t1291,t1292,t1293,t1294,t1299,t13,t130,t1300,t1304,t1305,t1306,t1307,t1308,t131,t1310,t1311,t1312,t1313,t1314,t1315,t1316,t1317,t1319,t1320,t1321,t1322,t1326,t1327,t1328,t1331,t1332,t1333,t1334,t1335,t1336,t1339,t1340,t1341,t1342,t1343,t1344,t1346,t1347,t1348,t1349,t135,t1350,t1351,t1352,t1354,t1355,t1356,t1357,t1358,t1359,t136,t1360,t1361,t1362,t1363,t1364,t1365,t1366,t1367,t1368,t1369,t137,t1370,t1378,t1379,t138,t1380,t1381,t1382,t1383,t1384,t1385,t139,t1393,t1394,t1395,t1396,t1397,t14,t140,t1400,t1401,t1402,t1410,t1411,t1412,t1413,t1414,t1415,t1416,t1417,t1418,t1419,t1420,t1421,t1422,t1425,t1426,t1427,t1428,t1429,t143,t1430,t1431,t1432,t1435,t1437,t1438,t1439,t144,t1440,t1441,t1442,t1443,t1444,t145,t1450,t1451,t1452,t1456,t1457,t1461,t1467,t1468,t1469,t147,t1470,t1476,t1477,t1478,t1479,t1481,t1482,t1483,t1484,t1485,t1486,t149,t1492,t1493,t1494,t1495,t1496,t15,t150,t1500,t1501,t1502,t1503,t1504,t1505,t1507,t1508,t1509,t151,t1510,t1511,t1512,t1513,t1514,t1517,t1518,t1519,t152,t1520,t1524,t1525,t153,t1533,t1534,t1537,t1538,t1539,t1550,t1551,t1552,t1555,t1558,t1559,t156,t1560,t1566,t1567,t1568,t157,t1570,t1571,t1572,t1575,t1576,t1577,t158,t1580,t159,t16,t160,t161,t162,t163,t164,t1648,t165,t166,t167,t168,t169,t17,t170,t1708,t171,t1717,t1723,t1736,t1739,t1747,t175,t1751,t1768,t178,t1788,t1789,t180,t181,t182,t185,t186,t187,t188,t189,t1895,t19,t190,t1904,t1916,t1926,t196,t197,t1980,t1983,t1990,t2,t20,t2003,t2004,t2009,t2010,t2015,t2018,t2023,t2027,t2030,t2031,t204,t205,t2050,t2059,t2060,t208,t2099,t21,t210,t211,t2121,t2129,t2135,t2143,t2144,t2145,t2162,t217,t218,t2194,t22,t221,t222,t223,t225,t228,t23,t230,t231,t232,t233,t234,t235,t236,t237,t238,t239,t24,t240,t241,t242,t243,t244,t246,t248,t25,t250,t251,t252,t253,t254,t255,t258,t259,t26,t261,t263,t264,t265,t266,t267,t268,t269,t27,t270,t271,t272,t273,t274,t275,t276,t277,t279,t28,t280,t281,t282,t283,t284,t285,t286,t287,t288,t289,t29,t290,t291,t292,t293,t294,t295,t296,t297,t298,t299,t3,t30,t300,t301,t302,t303,t304,t305,t306,t307,t308,t309,t31,t310,t311,t312,t313,t314,t315,t316,t317,t318,t319,t32,t320,t322,t323,t324,t3248,t3249,t325,t3252,t326,t327,t328,t329,t33,t330,t331,t332,t333,t334,t335,t336,t337,t338,t339,t34,t341,t342,t343,t344,t345,t346,t347,t348,t349,t35,t358,t359,t36,t360,t361,t362,t363,t364,t365,t366,t367,t368,t369,t37,t370,t371,t373,t374,t375,t376,t378,t380,t382,t385,t386,t387,t388,t389,t39,t390,t391,t392,t393,t394,t395,t396,t397,t398,t399,t4,t40,t400,t401,t402,t403,t404,t405,t406,t407,t408,t409,t410,t411,t412,t413,t414,t415,t416,t417,t418,t419,t42,t420,t425,t426,t427,t428,t429,t43,t431,t432,t433,t434,t435,t436,t438,t439,t44,t441,t442,t443,t444,t446,t447,t448,t449,t45,t450,t451,t452,t453,t454,t455,t456,t457,t458,t459,t46,t460,t461,t462,t463,t464,t465,t466,t467,t468,t469,t470,t471,t472,t473,t474,t476,t477,t478,t479,t480,t481,t483,t484,t486,t487,t488,t489,t49,t490,t491,t493,t494,t495,t496,t497,t498,t499,t5,t50,t500,t501,t502,t503,t504,t505,t506,t507,t508,t509,t51,t510,t511,t512,t513,t514,t515,t516,t517,t520,t530,t531,t534,t535,t536,t537,t538,t539,t540,t541,t542,t543,t544,t545,t546,t547,t548,t549,t55,t550,t551,t552,t553,t554,t555,t556,t557,t558,t559,t56,t560,t561,t562,t563,t564,t565,t566,t567,t568,t569,t57,t570,t571,t572,t573,t574,t577,t578,t579,t58,t580,t581,t582,t583,t584,t585,t588,t59,t590,t591,t592,t593,t6,t600,t601,t602,t603,t604,t605,t606,t607,t608,t609,t61,t610,t611,t612,t613,t614,t615,t616,t617,t618,t619,t62,t620,t621,t622,t623,t624,t626,t629,t63,t632,t633,t634,t637,t64,t640,t645,t647,t649,t65,t650,t651,t659,t67,t676,t677,t678,t687,t688,t69,t7,t70,t701,t702,t707,t71,t72,t722,t723,t724,t725,t728,t729,t73,t733,t734,t74,t75,t76,t761,t769,t77,t770,t771,t772,t78,t79,t8,t80,t81,t818,t819,t82,t823,t828,t829,t83,t830,t833,t84,t845,t85,t86,t87,t873,t874,t88,t89,t9,t90,t91,t92,t94,t96,t97,t98});
end
function C = ft_2(ct)
dq1 = ct{1};
dq2 = ct{2};
dq3 = ct{3};
dq4 = ct{4};
dq5 = ct{5};
dq6 = ct{6};
dq7 = ct{7};
t10 = ct{8};
t101 = ct{9};
t1020 = ct{10};
t1021 = ct{11};
t1026 = ct{12};
t1040 = ct{13};
t105 = ct{14};
t1058 = ct{15};
t1065 = ct{16};
t107 = ct{17};
t109 = ct{18};
t11 = ct{19};
t110 = ct{20};
t1101 = ct{21};
t1102 = ct{22};
t1105 = ct{23};
t1106 = ct{24};
t1109 = ct{25};
t111 = ct{26};
t112 = ct{27};
t1138 = ct{28};
t1139 = ct{29};
t114 = ct{30};
t1141 = ct{31};
t1142 = ct{32};
t1143 = ct{33};
t1144 = ct{34};
t1145 = ct{35};
t1146 = ct{36};
t1147 = ct{37};
t1148 = ct{38};
t1149 = ct{39};
t115 = ct{40};
t1150 = ct{41};
t1151 = ct{42};
t1152 = ct{43};
t1153 = ct{44};
t1154 = ct{45};
t1156 = ct{46};
t116 = ct{47};
t1162 = ct{48};
t1163 = ct{49};
t1164 = ct{50};
t1165 = ct{51};
t1166 = ct{52};
t1167 = ct{53};
t1168 = ct{54};
t1169 = ct{55};
t117 = ct{56};
t1170 = ct{57};
t1184 = ct{58};
t1189 = ct{59};
t119 = ct{60};
t1190 = ct{61};
t1193 = ct{62};
t1197 = ct{63};
t1198 = ct{64};
t1199 = ct{65};
t12 = ct{66};
t1200 = ct{67};
t1201 = ct{68};
t1202 = ct{69};
t1203 = ct{70};
t1204 = ct{71};
t1205 = ct{72};
t122 = ct{73};
t1230 = ct{74};
t1232 = ct{75};
t1234 = ct{76};
t124 = ct{77};
t1249 = ct{78};
t125 = ct{79};
t1250 = ct{80};
t1253 = ct{81};
t1257 = ct{82};
t126 = ct{83};
t1263 = ct{84};
t1264 = ct{85};
t1265 = ct{86};
t1266 = ct{87};
t1267 = ct{88};
t1268 = ct{89};
t127 = ct{90};
t1270 = ct{91};
t1276 = ct{92};
t1278 = ct{93};
t1280 = ct{94};
t1283 = ct{95};
t1284 = ct{96};
t1286 = ct{97};
t1291 = ct{98};
t1292 = ct{99};
t1293 = ct{100};
t1294 = ct{101};
t1299 = ct{102};
t13 = ct{103};
t130 = ct{104};
t1300 = ct{105};
t1304 = ct{106};
t1305 = ct{107};
t1306 = ct{108};
t1307 = ct{109};
t1308 = ct{110};
t131 = ct{111};
t1310 = ct{112};
t1311 = ct{113};
t1312 = ct{114};
t1313 = ct{115};
t1314 = ct{116};
t1315 = ct{117};
t1316 = ct{118};
t1317 = ct{119};
t1319 = ct{120};
t1320 = ct{121};
t1321 = ct{122};
t1322 = ct{123};
t1326 = ct{124};
t1327 = ct{125};
t1328 = ct{126};
t1331 = ct{127};
t1332 = ct{128};
t1333 = ct{129};
t1334 = ct{130};
t1335 = ct{131};
t1336 = ct{132};
t1339 = ct{133};
t1340 = ct{134};
t1341 = ct{135};
t1342 = ct{136};
t1343 = ct{137};
t1344 = ct{138};
t1346 = ct{139};
t1347 = ct{140};
t1348 = ct{141};
t1349 = ct{142};
t135 = ct{143};
t1350 = ct{144};
t1351 = ct{145};
t1352 = ct{146};
t1354 = ct{147};
t1355 = ct{148};
t1356 = ct{149};
t1357 = ct{150};
t1358 = ct{151};
t1359 = ct{152};
t136 = ct{153};
t1360 = ct{154};
t1361 = ct{155};
t1362 = ct{156};
t1363 = ct{157};
t1364 = ct{158};
t1365 = ct{159};
t1366 = ct{160};
t1367 = ct{161};
t1368 = ct{162};
t1369 = ct{163};
t137 = ct{164};
t1370 = ct{165};
t1378 = ct{166};
t1379 = ct{167};
t138 = ct{168};
t1380 = ct{169};
t1381 = ct{170};
t1382 = ct{171};
t1383 = ct{172};
t1384 = ct{173};
t1385 = ct{174};
t139 = ct{175};
t1393 = ct{176};
t1394 = ct{177};
t1395 = ct{178};
t1396 = ct{179};
t1397 = ct{180};
t14 = ct{181};
t140 = ct{182};
t1400 = ct{183};
t1401 = ct{184};
t1402 = ct{185};
t1410 = ct{186};
t1411 = ct{187};
t1412 = ct{188};
t1413 = ct{189};
t1414 = ct{190};
t1415 = ct{191};
t1416 = ct{192};
t1417 = ct{193};
t1418 = ct{194};
t1419 = ct{195};
t1420 = ct{196};
t1421 = ct{197};
t1422 = ct{198};
t1425 = ct{199};
t1426 = ct{200};
t1427 = ct{201};
t1428 = ct{202};
t1429 = ct{203};
t143 = ct{204};
t1430 = ct{205};
t1431 = ct{206};
t1432 = ct{207};
t1435 = ct{208};
t1437 = ct{209};
t1438 = ct{210};
t1439 = ct{211};
t144 = ct{212};
t1440 = ct{213};
t1441 = ct{214};
t1442 = ct{215};
t1443 = ct{216};
t1444 = ct{217};
t145 = ct{218};
t1450 = ct{219};
t1451 = ct{220};
t1452 = ct{221};
t1456 = ct{222};
t1457 = ct{223};
t1461 = ct{224};
t1467 = ct{225};
t1468 = ct{226};
t1469 = ct{227};
t147 = ct{228};
t1470 = ct{229};
t1476 = ct{230};
t1477 = ct{231};
t1478 = ct{232};
t1479 = ct{233};
t1481 = ct{234};
t1482 = ct{235};
t1483 = ct{236};
t1484 = ct{237};
t1485 = ct{238};
t1486 = ct{239};
t149 = ct{240};
t1492 = ct{241};
t1493 = ct{242};
t1494 = ct{243};
t1495 = ct{244};
t1496 = ct{245};
t15 = ct{246};
t150 = ct{247};
t1500 = ct{248};
t1501 = ct{249};
t1502 = ct{250};
t1503 = ct{251};
t1504 = ct{252};
t1505 = ct{253};
t1507 = ct{254};
t1508 = ct{255};
t1509 = ct{256};
t151 = ct{257};
t1510 = ct{258};
t1511 = ct{259};
t1512 = ct{260};
t1513 = ct{261};
t1514 = ct{262};
t1517 = ct{263};
t1518 = ct{264};
t1519 = ct{265};
t152 = ct{266};
t1520 = ct{267};
t1524 = ct{268};
t1525 = ct{269};
t153 = ct{270};
t1533 = ct{271};
t1534 = ct{272};
t1537 = ct{273};
t1538 = ct{274};
t1539 = ct{275};
t1550 = ct{276};
t1551 = ct{277};
t1552 = ct{278};
t1555 = ct{279};
t1558 = ct{280};
t1559 = ct{281};
t156 = ct{282};
t1560 = ct{283};
t1566 = ct{284};
t1567 = ct{285};
t1568 = ct{286};
t157 = ct{287};
t1570 = ct{288};
t1571 = ct{289};
t1572 = ct{290};
t1575 = ct{291};
t1576 = ct{292};
t1577 = ct{293};
t158 = ct{294};
t1580 = ct{295};
t159 = ct{296};
t16 = ct{297};
t160 = ct{298};
t161 = ct{299};
t162 = ct{300};
t163 = ct{301};
t164 = ct{302};
t1648 = ct{303};
t165 = ct{304};
t166 = ct{305};
t167 = ct{306};
t168 = ct{307};
t169 = ct{308};
t17 = ct{309};
t170 = ct{310};
t1708 = ct{311};
t171 = ct{312};
t1717 = ct{313};
t1723 = ct{314};
t1736 = ct{315};
t1739 = ct{316};
t1747 = ct{317};
t175 = ct{318};
t1751 = ct{319};
t1768 = ct{320};
t178 = ct{321};
t1788 = ct{322};
t1789 = ct{323};
t180 = ct{324};
t181 = ct{325};
t182 = ct{326};
t185 = ct{327};
t186 = ct{328};
t187 = ct{329};
t188 = ct{330};
t189 = ct{331};
t1895 = ct{332};
t19 = ct{333};
t190 = ct{334};
t1904 = ct{335};
t1916 = ct{336};
t1926 = ct{337};
t196 = ct{338};
t197 = ct{339};
t1980 = ct{340};
t1983 = ct{341};
t1990 = ct{342};
t2 = ct{343};
t20 = ct{344};
t2003 = ct{345};
t2004 = ct{346};
t2009 = ct{347};
t2010 = ct{348};
t2015 = ct{349};
t2018 = ct{350};
t2023 = ct{351};
t2027 = ct{352};
t2030 = ct{353};
t2031 = ct{354};
t204 = ct{355};
t205 = ct{356};
t2050 = ct{357};
t2059 = ct{358};
t2060 = ct{359};
t208 = ct{360};
t2099 = ct{361};
t21 = ct{362};
t210 = ct{363};
t211 = ct{364};
t2121 = ct{365};
t2129 = ct{366};
t2135 = ct{367};
t2143 = ct{368};
t2144 = ct{369};
t2145 = ct{370};
t2162 = ct{371};
t217 = ct{372};
t218 = ct{373};
t2194 = ct{374};
t22 = ct{375};
t221 = ct{376};
t222 = ct{377};
t223 = ct{378};
t225 = ct{379};
t228 = ct{380};
t23 = ct{381};
t230 = ct{382};
t231 = ct{383};
t232 = ct{384};
t233 = ct{385};
t234 = ct{386};
t235 = ct{387};
t236 = ct{388};
t237 = ct{389};
t238 = ct{390};
t239 = ct{391};
t24 = ct{392};
t240 = ct{393};
t241 = ct{394};
t242 = ct{395};
t243 = ct{396};
t244 = ct{397};
t246 = ct{398};
t248 = ct{399};
t25 = ct{400};
t250 = ct{401};
t251 = ct{402};
t252 = ct{403};
t253 = ct{404};
t254 = ct{405};
t255 = ct{406};
t258 = ct{407};
t259 = ct{408};
t26 = ct{409};
t261 = ct{410};
t263 = ct{411};
t264 = ct{412};
t265 = ct{413};
t266 = ct{414};
t267 = ct{415};
t268 = ct{416};
t269 = ct{417};
t27 = ct{418};
t270 = ct{419};
t271 = ct{420};
t272 = ct{421};
t273 = ct{422};
t274 = ct{423};
t275 = ct{424};
t276 = ct{425};
t277 = ct{426};
t279 = ct{427};
t28 = ct{428};
t280 = ct{429};
t281 = ct{430};
t282 = ct{431};
t283 = ct{432};
t284 = ct{433};
t285 = ct{434};
t286 = ct{435};
t287 = ct{436};
t288 = ct{437};
t289 = ct{438};
t29 = ct{439};
t290 = ct{440};
t291 = ct{441};
t292 = ct{442};
t293 = ct{443};
t294 = ct{444};
t295 = ct{445};
t296 = ct{446};
t297 = ct{447};
t298 = ct{448};
t299 = ct{449};
t3 = ct{450};
t30 = ct{451};
t300 = ct{452};
t301 = ct{453};
t302 = ct{454};
t303 = ct{455};
t304 = ct{456};
t305 = ct{457};
t306 = ct{458};
t307 = ct{459};
t308 = ct{460};
t309 = ct{461};
t31 = ct{462};
t310 = ct{463};
t311 = ct{464};
t312 = ct{465};
t313 = ct{466};
t314 = ct{467};
t315 = ct{468};
t316 = ct{469};
t317 = ct{470};
t318 = ct{471};
t319 = ct{472};
t32 = ct{473};
t320 = ct{474};
t322 = ct{475};
t323 = ct{476};
t324 = ct{477};
t3248 = ct{478};
t3249 = ct{479};
t325 = ct{480};
t3252 = ct{481};
t326 = ct{482};
t327 = ct{483};
t328 = ct{484};
t329 = ct{485};
t33 = ct{486};
t330 = ct{487};
t331 = ct{488};
t332 = ct{489};
t333 = ct{490};
t334 = ct{491};
t335 = ct{492};
t336 = ct{493};
t337 = ct{494};
t338 = ct{495};
t339 = ct{496};
t34 = ct{497};
t341 = ct{498};
t342 = ct{499};
t343 = ct{500};
t344 = ct{501};
t345 = ct{502};
t346 = ct{503};
t347 = ct{504};
t348 = ct{505};
t349 = ct{506};
t35 = ct{507};
t358 = ct{508};
t359 = ct{509};
t36 = ct{510};
t360 = ct{511};
t361 = ct{512};
t362 = ct{513};
t363 = ct{514};
t364 = ct{515};
t365 = ct{516};
t366 = ct{517};
t367 = ct{518};
t368 = ct{519};
t369 = ct{520};
t37 = ct{521};
t370 = ct{522};
t371 = ct{523};
t373 = ct{524};
t374 = ct{525};
t375 = ct{526};
t376 = ct{527};
t378 = ct{528};
t380 = ct{529};
t382 = ct{530};
t385 = ct{531};
t386 = ct{532};
t387 = ct{533};
t388 = ct{534};
t389 = ct{535};
t39 = ct{536};
t390 = ct{537};
t391 = ct{538};
t392 = ct{539};
t393 = ct{540};
t394 = ct{541};
t395 = ct{542};
t396 = ct{543};
t397 = ct{544};
t398 = ct{545};
t399 = ct{546};
t4 = ct{547};
t40 = ct{548};
t400 = ct{549};
t401 = ct{550};
t402 = ct{551};
t403 = ct{552};
t404 = ct{553};
t405 = ct{554};
t406 = ct{555};
t407 = ct{556};
t408 = ct{557};
t409 = ct{558};
t410 = ct{559};
t411 = ct{560};
t412 = ct{561};
t413 = ct{562};
t414 = ct{563};
t415 = ct{564};
t416 = ct{565};
t417 = ct{566};
t418 = ct{567};
t419 = ct{568};
t42 = ct{569};
t420 = ct{570};
t425 = ct{571};
t426 = ct{572};
t427 = ct{573};
t428 = ct{574};
t429 = ct{575};
t43 = ct{576};
t431 = ct{577};
t432 = ct{578};
t433 = ct{579};
t434 = ct{580};
t435 = ct{581};
t436 = ct{582};
t438 = ct{583};
t439 = ct{584};
t44 = ct{585};
t441 = ct{586};
t442 = ct{587};
t443 = ct{588};
t444 = ct{589};
t446 = ct{590};
t447 = ct{591};
t448 = ct{592};
t449 = ct{593};
t45 = ct{594};
t450 = ct{595};
t451 = ct{596};
t452 = ct{597};
t453 = ct{598};
t454 = ct{599};
t455 = ct{600};
t456 = ct{601};
t457 = ct{602};
t458 = ct{603};
t459 = ct{604};
t46 = ct{605};
t460 = ct{606};
t461 = ct{607};
t462 = ct{608};
t463 = ct{609};
t464 = ct{610};
t465 = ct{611};
t466 = ct{612};
t467 = ct{613};
t468 = ct{614};
t469 = ct{615};
t470 = ct{616};
t471 = ct{617};
t472 = ct{618};
t473 = ct{619};
t474 = ct{620};
t476 = ct{621};
t477 = ct{622};
t478 = ct{623};
t479 = ct{624};
t480 = ct{625};
t481 = ct{626};
t483 = ct{627};
t484 = ct{628};
t486 = ct{629};
t487 = ct{630};
t488 = ct{631};
t489 = ct{632};
t49 = ct{633};
t490 = ct{634};
t491 = ct{635};
t493 = ct{636};
t494 = ct{637};
t495 = ct{638};
t496 = ct{639};
t497 = ct{640};
t498 = ct{641};
t499 = ct{642};
t5 = ct{643};
t50 = ct{644};
t500 = ct{645};
t501 = ct{646};
t502 = ct{647};
t503 = ct{648};
t504 = ct{649};
t505 = ct{650};
t506 = ct{651};
t507 = ct{652};
t508 = ct{653};
t509 = ct{654};
t51 = ct{655};
t510 = ct{656};
t511 = ct{657};
t512 = ct{658};
t513 = ct{659};
t514 = ct{660};
t515 = ct{661};
t516 = ct{662};
t517 = ct{663};
t520 = ct{664};
t530 = ct{665};
t531 = ct{666};
t534 = ct{667};
t535 = ct{668};
t536 = ct{669};
t537 = ct{670};
t538 = ct{671};
t539 = ct{672};
t540 = ct{673};
t541 = ct{674};
t542 = ct{675};
t543 = ct{676};
t544 = ct{677};
t545 = ct{678};
t546 = ct{679};
t547 = ct{680};
t548 = ct{681};
t549 = ct{682};
t55 = ct{683};
t550 = ct{684};
t551 = ct{685};
t552 = ct{686};
t553 = ct{687};
t554 = ct{688};
t555 = ct{689};
t556 = ct{690};
t557 = ct{691};
t558 = ct{692};
t559 = ct{693};
t56 = ct{694};
t560 = ct{695};
t561 = ct{696};
t562 = ct{697};
t563 = ct{698};
t564 = ct{699};
t565 = ct{700};
t566 = ct{701};
t567 = ct{702};
t568 = ct{703};
t569 = ct{704};
t57 = ct{705};
t570 = ct{706};
t571 = ct{707};
t572 = ct{708};
t573 = ct{709};
t574 = ct{710};
t577 = ct{711};
t578 = ct{712};
t579 = ct{713};
t58 = ct{714};
t580 = ct{715};
t581 = ct{716};
t582 = ct{717};
t583 = ct{718};
t584 = ct{719};
t585 = ct{720};
t588 = ct{721};
t59 = ct{722};
t590 = ct{723};
t591 = ct{724};
t592 = ct{725};
t593 = ct{726};
t6 = ct{727};
t600 = ct{728};
t601 = ct{729};
t602 = ct{730};
t603 = ct{731};
t604 = ct{732};
t605 = ct{733};
t606 = ct{734};
t607 = ct{735};
t608 = ct{736};
t609 = ct{737};
t61 = ct{738};
t610 = ct{739};
t611 = ct{740};
t612 = ct{741};
t613 = ct{742};
t614 = ct{743};
t615 = ct{744};
t616 = ct{745};
t617 = ct{746};
t618 = ct{747};
t619 = ct{748};
t62 = ct{749};
t620 = ct{750};
t621 = ct{751};
t622 = ct{752};
t623 = ct{753};
t624 = ct{754};
t626 = ct{755};
t629 = ct{756};
t63 = ct{757};
t632 = ct{758};
t633 = ct{759};
t634 = ct{760};
t637 = ct{761};
t64 = ct{762};
t640 = ct{763};
t645 = ct{764};
t647 = ct{765};
t649 = ct{766};
t65 = ct{767};
t650 = ct{768};
t651 = ct{769};
t659 = ct{770};
t67 = ct{771};
t676 = ct{772};
t677 = ct{773};
t678 = ct{774};
t687 = ct{775};
t688 = ct{776};
t69 = ct{777};
t7 = ct{778};
t70 = ct{779};
t701 = ct{780};
t702 = ct{781};
t707 = ct{782};
t71 = ct{783};
t72 = ct{784};
t722 = ct{785};
t723 = ct{786};
t724 = ct{787};
t725 = ct{788};
t728 = ct{789};
t729 = ct{790};
t73 = ct{791};
t733 = ct{792};
t734 = ct{793};
t74 = ct{794};
t75 = ct{795};
t76 = ct{796};
t761 = ct{797};
t769 = ct{798};
t77 = ct{799};
t770 = ct{800};
t771 = ct{801};
t772 = ct{802};
t78 = ct{803};
t79 = ct{804};
t8 = ct{805};
t80 = ct{806};
t81 = ct{807};
t818 = ct{808};
t819 = ct{809};
t82 = ct{810};
t823 = ct{811};
t828 = ct{812};
t829 = ct{813};
t83 = ct{814};
t830 = ct{815};
t833 = ct{816};
t84 = ct{817};
t845 = ct{818};
t85 = ct{819};
t86 = ct{820};
t87 = ct{821};
t873 = ct{822};
t874 = ct{823};
t88 = ct{824};
t89 = ct{825};
t9 = ct{826};
t90 = ct{827};
t91 = ct{828};
t92 = ct{829};
t94 = ct{830};
t96 = ct{831};
t97 = ct{832};
t98 = ct{833};
t518 = -t446;
t519 = -t327;
t521 = -t330;
t522 = -t447;
t523 = -t449;
t524 = -t450;
t525 = -t451;
t526 = -t453;
t527 = -t454;
t528 = -t455;
t529 = -t458;
t532 = -t461;
t533 = -t462;
t575 = -t542;
t576 = -t543;
t586 = -t549;
t587 = -t550;
t589 = -t555;
t594 = -t559;
t595 = -t560;
t596 = -t563;
t597 = -t582;
t598 = -t584;
t599 = -t585;
t625 = dq4.*t617;
t627 = dq5.*t618;
t628 = dq5.*t619;
t630 = dq5.*t620;
t631 = dq6.*t621;
t635 = t604.^2;
t636 = dq4.*t612;
t638 = dq5.*t613;
t639 = dq5.*t614;
t641 = dq5.*t615;
t642 = dq6.*t616;
t643 = t5.*t614;
t644 = t6.*t616;
t646 = t5.*t619;
t648 = t6.*t621;
t652 = t5.*t605;
t653 = t6.*t604;
t654 = t6.*t605;
t655 = -t614;
t656 = t6.*t606;
t657 = t7.*t606;
t658 = t7.*t607;
t660 = t12.*t605;
t661 = t13.*t604;
t662 = t13.*t605;
t663 = t13.*t606;
t664 = t14.*t606;
t665 = t14.*t607;
t666 = -t621;
t667 = dq4.*t12.*t604;
t679 = t19.*t612;
t680 = t20.*t614;
t681 = t21.*t616;
t682 = t19.*t617;
t683 = t20.*t619;
t684 = t21.*t621;
t685 = t612.*(2.0./5.0);
t686 = t617.*(2.0./5.0);
t689 = t7.*t637;
t691 = t8.*t640;
t693 = dq4.*t12.*t614;
t694 = t14.*t637;
t696 = dq6.*t647;
t697 = dq5.*t13.*t616;
t698 = t15.*t640;
t700 = dq7.*t649;
t703 = dq4.*t12.*t619;
t704 = dq6.*t650;
t705 = dq5.*t13.*t621;
t706 = dq7.*t651;
t708 = dq4.*t5.*t604;
t711 = -t637;
t716 = -t640;
t731 = t7.*t12.*t604;
t735 = t12.*t14.*t604;
t736 = -t650;
t737 = -t651;
t739 = -t659;
t743 = t637.*(2.0./5.0);
t755 = dq6.*t722;
t756 = t12.*t604.*(2.0./5.0);
t758 = dq6.*t723;
t759 = dq6.*t724;
t760 = dq6.*t725;
t767 = dq6.*t728;
t768 = dq6.*t729;
t785 = t6.*t676;
t786 = t13.*t676;
t787 = t6.*t677;
t788 = t8.*t678;
t791 = t13.*t677;
t792 = t15.*t678;
t793 = -t733;
t815 = t70+t612;
t817 = t83+t620;
t826 = t264+t617;
t832 = t265+t615;
t840 = t139+t149+t301;
t841 = t107+t114+t342;
t842 = t112+t119+t338;
t843 = t122+t130+t346;
t847 = (t88-t617).^2;
t854 = t6.*t818;
t855 = t7.*t819;
t856 = t13.*t818;
t857 = t14.*t819;
t859 = t569.*t606;
t861 = -t7.*(t90-t615);
t862 = -t7.*(t88-t617);
t865 = -t14.*(t90-t615);
t867 = t2.*t828;
t868 = t3.*t829;
t869 = -t14.*(t88-t617);
t875 = -t845;
t881 = -dq5.*t6.*(t88-t617);
t892 = -dq5.*t13.*(t88-t617);
t898 = t259+t725;
t905 = t2.*t10.*t830;
t910 = -t8.*t13.*(t88-t617);
t912 = t601.*t605;
t916 = -t13.*t15.*(t88-t617);
t924 = -t873;
t925 = -t874;
t944 = dq6.*t7.*(t90-t615);
t948 = dq5.*t6.*(t88-t617);
t960 = t493+t729;
t966 = t6.*t7.*(t88-t617);
t969 = t8.*t13.*(t88-t617);
t999 = t7.*t21.*(t88-t617);
t1047 = t5.*t1020;
t1048 = t6.*t1020;
t1049 = t12.*t1020;
t1050 = t13.*t1020;
t1057 = t571.*t828;
t1066 = t65+t138+t143+t169+t302;
t1067 = t62+t145+t150+t170+t300;
t1068 = t42+t153+t159+t190+t306;
t1069 = t44+t161+t164+t188+t303;
t1070 = t56+t59+t178+t323+t326;
t1071 = t605.*t823;
t1072 = t2.*t10.*t1020;
t1075 = t5.*t1040;
t1076 = t6.*t1040;
t1079 = t12.*t1040;
t1080 = t13.*t1040;
t1083 = t606.*t829;
t1112 = t6.*t1065;
t1121 = t13.*t1065;
t1124 = t9.*t10.*t1040;
t1173 = -t1148;
t1174 = -t1149;
t1175 = -t1150;
t1176 = -t1151;
t1177 = -t1152;
t1178 = -t1153;
t1179 = -t1154;
t1181 = t45.*t1040;
t1182 = t50.*t1040;
t1183 = -t1156;
t1194 = -t1162;
t1195 = -t1163;
t1208 = -t1170;
t1275 = -t1230;
t1376 = -t1311;
t1377 = -t1314;
t1388 = -t1319;
t1389 = -t1320;
t1390 = -t1321;
t1391 = -t1322;
t1406 = -t1336;
t1423 = -t1340;
t1436 = -t1354;
t1445 = -t1366;
t1446 = -t1367;
t1449 = -t1370;
t1453 = -t1378;
t1454 = -t1379;
t1455 = -t1383;
t1458 = -t1393;
t1459 = -t1394;
t1460 = -t1395;
t1463 = -t1411;
t1474 = -t1413;
t1475 = -t1414;
t1480 = -t1415;
t1490 = -t1419;
t1491 = -t1420;
t1497 = -t1426;
t1498 = -t1427;
t1499 = t572.*t1020;
t1506 = -t1437;
t1521 = -t1442;
t1522 = -t1443;
t1523 = -t1444;
t1540 = -t1468;
t1541 = -t1469;
t1542 = -t1470;
t1543 = -t1476;
t1544 = -t1477;
t1545 = -t1478;
t1546 = -t1479;
t1547 = -t1481;
t1548 = -t1482;
t1549 = -t1484;
t1553 = -t1493;
t1554 = -t1494;
t1556 = -t1500;
t1561 = -t1501;
t1562 = -t1502;
t1563 = -t1503;
t1565 = -t1507;
t1569 = -t1514;
t1573 = -t1520;
t1591 = -t1555;
t1592 = t601.*t1020;
t1603 = t637.*1.8866e-1;
t1605 = -t1580;
t1627 = t573.*t1065;
t1641 = t640.*2.75e-2;
t1852 = t111+t116+t124+t307+t311+t499+t503;
t1877 = dq6.*t7.*(t88-t617).*(-4.9e-4);
t1885 = t101+t283+t288+t291+t332+t334+t497;
t1892 = t109+t126+t312+t314+t341+t498+t500;
t1894 = dq6.*t14.*(t88-t617).*(-2.019e-2);
t1896 = t96+t282+t285+t292+t335+t337+t520;
t1898 = t14.*t21.*(t88-t617).*(-4.9e-4);
t1900 = dq6.*t14.*(t88-t617).*2.019e-2;
t1908 = dq6.*t6.*t14.*(t88-t617).*(-4.9e-4);
t1930 = t659.*8.909980864224564e-21;
t1948 = t659.*5.582083966615414e-19;
t1956 = t733.*1.16152294893368e-19;
t1960 = dq7.*t13.*t15.*(t88-t617).*(-2.324e-2);
t1964 = t733.*8.909980864224564e-21;
t1977 = dq6.*t14.*(t88-t617).*(-1.9738e-1);
t2150 = t734.*7.000000000000001e-5;
t2153 = t734.*7.000000000000022e-5;
t2154 = t659.*3.199999999999801e-4;
t2155 = -t2144;
t2158 = -t2145;
t2166 = t771.*7.000000000000001e-5;
t2167 = t772.*7.000000000000001e-5;
t2174 = t771.*7.000000000000022e-5;
t2175 = t772.*7.000000000000022e-5;
t2199 = t222+t225+t246+t401+t403+t404+t539+t540+t541;
t2238 = t733.*4.200000000000139e-4;
t2243 = t734.*7.299999999999999e-4;
t2284 = t771.*7.299999999999999e-4;
t2285 = t772.*7.299999999999999e-4;
t2298 = t833.*7.000000000000022e-5;
t2317 = t833.*4.999999999999997e-5;
t2324 = t874.*7.000000000000001e-5;
t2328 = t874.*7.000000000000022e-5;
t2340 = t833.*2.19e-3;
t2354 = t874.*7.299999999999999e-4;
t668 = dq4.*t660;
t669 = -t625;
t670 = dq5.*t661;
t671 = dq5.*t662;
t672 = dq5.*t663;
t673 = dq6.*t664;
t674 = dq6.*t665;
t675 = -t631;
t690 = t5.*t639;
t692 = t6.*t642;
t695 = t5.*t628;
t699 = t6.*t631;
t709 = dq4.*t652;
t710 = -t636;
t712 = dq5.*t653;
t713 = dq5.*t654;
t714 = -t639;
t715 = dq5.*t656;
t717 = -t641;
t718 = dq6.*t657;
t719 = dq6.*t658;
t720 = -t642;
t721 = t625.*(2.0./5.0);
t726 = t5.*t653;
t727 = -t643;
t730 = t5.*t661;
t732 = -t648;
t738 = -t653;
t740 = -t686;
t741 = -t665;
t742 = t636.*(2.0./5.0);
t746 = t19.*t652;
t747 = t20.*t653;
t748 = t20.*t656;
t749 = t19.*t660;
t750 = -t682;
t751 = t20.*t661;
t752 = t20.*t663;
t753 = t21.*t666;
t754 = t652.*(2.0./5.0);
t757 = t660.*(2.0./5.0);
t762 = t7.*t708;
t765 = -t691;
t773 = dq4.*t12.*t653;
t774 = t14.*t708;
t776 = dq6.*t731;
t777 = -t696;
t778 = dq4.*t12.*t661;
t779 = dq6.*t735;
t780 = -t704;
t781 = -t708;
t789 = t682.*(2.0./5.0);
t794 = -t735;
t795 = t708.*(2.0./5.0);
t802 = dq5.*t785;
t803 = -t755;
t804 = dq5.*t786;
t805 = dq5.*t787;
t806 = dq7.*t788;
t808 = dq5.*t791;
t809 = -t767;
t810 = -t768;
t811 = dq7.*t792;
t827 = t71+t656;
t831 = t79+t660;
t834 = t8.*t817;
t835 = t6.*t815;
t836 = t7.*t815;
t837 = t15.*t817;
t838 = t13.*t815;
t839 = t14.*t815;
t844 = t266+t663;
t858 = t263+t652;
t876 = (t92-t663).^2;
t879 = dq6.*t861;
t880 = t5.*t840;
t883 = dq6.*t862;
t886 = dq6.*t865;
t888 = t5.*t841;
t889 = t12.*t840;
t890 = t6.*t842;
t891 = t6.*t843;
t894 = dq6.*t869;
t899 = t12.*t841;
t900 = t13.*t842;
t901 = -t854;
t902 = t13.*t843;
t903 = -t855;
t906 = t6.*t862;
t909 = t6.*t869;
t913 = -t859;
t914 = -t6.*(t86-t652);
t915 = -t7.*(t86-t652);
t917 = -t13.*(t86-t652);
t918 = -t14.*(t86-t652);
t919 = -t8.*(t92-t663);
t920 = -t15.*(t92-t663);
t922 = t21.*t869;
t929 = t8.*t881;
t934 = dq5.*t13.*t862;
t936 = t15.*t881;
t938 = dq7.*t910;
t940 = t251+t785;
t945 = dq5.*t13.*t869;
t946 = dq7.*t916;
t952 = -dq6.*t7.*(t92-t663);
t956 = -dq6.*t14.*(t92-t663);
t959 = t258+t787;
t962 = t21.*t862;
t965 = -t905;
t971 = -t912;
t974 = t8.*t898;
t975 = t15.*t898;
t982 = t8.*t948;
t983 = dq6.*t966;
t987 = dq7.*t969;
t991 = t486+t786;
t992 = dq6.*t7.*(t86-t652);
t994 = dq6.*t14.*(t92-t663);
t995 = dq7.*t15.*(t92-t663);
t996 = t491+t791;
t1001 = t7.*t15.*(t92-t663);
t1010 = t15.*t22.*(t92-t663);
t1019 = t13.*t20.*(t86-t652);
t1023 = t646+t654;
t1024 = t644+t664;
t1025 = t610+t739;
t1028 = -t8.*(t243-t786);
t1029 = -t15.*(t243-t786);
t1031 = -t8.*(t252-t791);
t1032 = -t15.*(t252-t791);
t1044 = t8.*(t243-t786);
t1046 = dq7.*t15.*(t243-t786);
t1073 = -t1047;
t1074 = -t1048;
t1078 = -t7.*(t643-t662);
t1082 = -t14.*(t643-t662);
t1084 = dq4.*t1047.*2.0;
t1085 = dq4.*t1049.*2.0;
t1096 = t1047.*(2.0./5.0);
t1097 = t1049.*(2.0./5.0);
t1098 = -t1071;
t1103 = dq5.*t1076.*2.0;
t1104 = dq5.*t1080.*2.0;
t1110 = t6.*t1075;
t1113 = t13.*t1075;
t1114 = t7.*t1079;
t1115 = t5.*t1066;
t1116 = t5.*t1067;
t1117 = t6.*t1066;
t1118 = t6.*t1067;
t1120 = t6.*t1069;
t1122 = t7.*t1068;
t1123 = t7.*t1069;
t1125 = t14.*t1079;
t1126 = t12.*t1066;
t1127 = t12.*t1067;
t1128 = t13.*t1066;
t1129 = t13.*t1067;
t1130 = t6.*t1070;
t1131 = t13.*t1069;
t1132 = t7.*t1070;
t1133 = t14.*t1068;
t1134 = t14.*t1069;
t1135 = -t1080;
t1136 = t13.*t1070;
t1137 = t14.*t1070;
t1140 = -t1083;
t1155 = dq4.*t1047.*(4.0./5.0);
t1159 = dq6.*t7.*(t643-t662);
t1161 = dq6.*t14.*(t643-t662);
t1172 = t1079.*(2.0./5.0);
t1210 = t2.*t10.*t1066;
t1214 = t9.*t10.*t1067;
t1217 = t10.*t11.*t1068;
t1218 = t10.*t11.*t1069;
t1223 = -t1124;
t1225 = t10.*t11.*t1070;
t1256 = t69+t645+t793;
t1277 = t39.*t1066;
t1287 = t61.*t1066;
t1288 = t51.*t1070;
t1289 = t58.*t1070;
t1296 = t658+t865;
t1574 = (t614+t13.*(t86-t652)).^2;
t1593 = -t1499;
t1596 = -t8.*(t614+t13.*(t86-t652));
t1597 = -t8.*(t665+t7.*(t90-t615));
t1599 = -t15.*(t614+t13.*(t86-t652));
t1600 = -t15.*(t665+t7.*(t90-t615));
t1602 = t636.*1.8866e-1;
t1616 = -dq6.*t7.*(t614+t13.*(t86-t652));
t1622 = -dq6.*t14.*(t614+t13.*(t86-t652));
t1628 = t567.*t1067;
t1629 = t569.*t1069;
t1630 = t573.*t1069;
t1634 = t8.*(t665+t7.*(t90-t615));
t1635 = t15.*(t614+t13.*(t86-t652));
t1636 = t708.*1.8866e-1;
t1638 = t627.*2.37e-3;
t1639 = t628.*2.37e-3;
t1640 = t682.*1.8866e-1;
t1643 = t627.*2.75e-2;
t1644 = t628.*2.75e-2;
t1661 = dq6.*t14.*(t614+t13.*(t86-t652));
t1664 = t680.*2.37e-3;
t1665 = t604.*t1067;
t1666 = t636.*5.267999999999999e-2;
t1667 = -t1641;
t1674 = t642.*4.9e-4;
t1675 = t638.*5.000000000000001e-5;
t1676 = t639.*5.000000000000001e-5;
t1683 = t680.*2.75e-2;
t1684 = t631.*2.019e-2;
t1694 = t684.*4.9e-4;
t1696 = t682.*5.267999999999999e-2;
t1698 = t625.*2.0e-4;
t1701 = t696.*4.9e-4;
t1704 = t681.*2.019e-2;
t1713 = t683.*5.000000000000001e-5;
t1715 = t704.*2.019e-2;
t1734 = t700.*3.466000000000001e-2;
t1735 = t755.*4.9e-4;
t1740 = t759.*4.9e-4;
t1741 = t768.*4.9e-4;
t1744 = t679.*2.0e-4;
t1748 = t667+t1075;
t1754 = t758.*2.019e-2;
t1756 = t760.*2.019e-2;
t1758 = t767.*2.019e-2;
t1760 = t706.*2.324e-2;
t1772 = t631.*1.9738e-1;
t1791 = t815.*t1040;
t1807 = t681.*1.9738e-1;
t1814 = t704.*1.9738e-1;
t1818 = -t1020.*(t86-t652);
t1819 = t815.*t1067;
t1820 = -t8.*(t650+t7.*(t643-t662));
t1821 = -t15.*(t650+t7.*(t643-t662));
t1827 = -t7.*(t708-t1079);
t1831 = -t14.*(t708-t1079);
t1834 = t758.*1.9738e-1;
C = ft_3({dq1,dq2,dq3,dq4,dq5,dq6,dq7,t10,t1001,t101,t1010,t1019,t1020,t1021,t1023,t1024,t1025,t1026,t1028,t1029,t1031,t1032,t1040,t1044,t1046,t1047,t1048,t1049,t105,t1050,t1057,t1058,t1066,t1067,t1068,t1069,t107,t1070,t1071,t1072,t1073,t1074,t1075,t1076,t1078,t1079,t1080,t1082,t1083,t1084,t1085,t109,t1096,t1097,t1098,t11,t110,t1101,t1102,t1103,t1104,t1105,t1106,t1109,t111,t1110,t1112,t1113,t1114,t1115,t1116,t1117,t1118,t112,t1120,t1121,t1122,t1123,t1124,t1125,t1126,t1127,t1128,t1129,t1130,t1131,t1132,t1133,t1134,t1135,t1136,t1137,t1138,t1139,t114,t1140,t1141,t1142,t1143,t1144,t1145,t1146,t1147,t115,t1155,t1159,t116,t1161,t1164,t1165,t1166,t1167,t1168,t1169,t117,t1172,t1173,t1174,t1175,t1176,t1177,t1178,t1179,t1181,t1182,t1183,t1184,t1189,t119,t1190,t1193,t1194,t1195,t1197,t1198,t1199,t12,t1200,t1201,t1202,t1203,t1204,t1205,t1208,t1210,t1214,t1217,t1218,t122,t1223,t1225,t1232,t1234,t124,t1249,t125,t1250,t1253,t1256,t1257,t126,t1263,t1264,t1265,t1266,t1267,t1268,t127,t1270,t1275,t1276,t1277,t1278,t1280,t1283,t1284,t1286,t1287,t1288,t1289,t1291,t1292,t1293,t1294,t1296,t1299,t13,t130,t1300,t1304,t1305,t1306,t1307,t1308,t131,t1310,t1312,t1313,t1315,t1316,t1317,t1326,t1327,t1328,t1331,t1332,t1333,t1334,t1335,t1339,t1341,t1342,t1343,t1344,t1346,t1347,t1348,t1349,t135,t1350,t1351,t1352,t1355,t1356,t1357,t1358,t1359,t136,t1360,t1361,t1362,t1363,t1364,t1365,t1368,t1369,t137,t1376,t1377,t1380,t1381,t1382,t1384,t1385,t1388,t1389,t139,t1390,t1391,t1396,t1397,t14,t140,t1400,t1401,t1402,t1406,t1410,t1412,t1416,t1417,t1418,t1421,t1422,t1423,t1425,t1428,t1429,t1430,t1431,t1432,t1435,t1436,t1438,t1439,t144,t1440,t1441,t1445,t1446,t1449,t1450,t1451,t1452,t1453,t1454,t1455,t1456,t1457,t1458,t1459,t1460,t1461,t1463,t1467,t147,t1474,t1475,t1480,t1483,t1485,t1486,t149,t1490,t1491,t1492,t1495,t1496,t1497,t1498,t1499,t15,t1504,t1505,t1506,t1508,t1509,t151,t1510,t1511,t1512,t1513,t1517,t1518,t1519,t152,t1521,t1522,t1523,t1524,t1525,t1533,t1534,t1537,t1538,t1539,t1540,t1541,t1542,t1543,t1544,t1545,t1546,t1547,t1548,t1549,t1550,t1551,t1552,t1553,t1554,t1556,t1558,t1559,t156,t1560,t1561,t1562,t1563,t1565,t1566,t1567,t1568,t1569,t157,t1570,t1571,t1572,t1573,t1574,t1575,t1576,t1577,t158,t1591,t1592,t1593,t1596,t1597,t1599,t16,t160,t1600,t1602,t1603,t1605,t1616,t162,t1622,t1627,t1628,t1629,t163,t1630,t1634,t1635,t1636,t1638,t1639,t1640,t1643,t1644,t1648,t165,t166,t1661,t1664,t1665,t1666,t1667,t167,t1674,t1675,t1676,t168,t1683,t1684,t1694,t1696,t1698,t17,t1701,t1704,t1708,t171,t1713,t1715,t1717,t1723,t1734,t1735,t1736,t1739,t1740,t1741,t1744,t1747,t1748,t175,t1751,t1754,t1756,t1758,t1760,t1768,t1772,t1788,t1789,t1791,t180,t1807,t181,t1814,t1819,t182,t1820,t1821,t1827,t1831,t1834,t185,t1852,t186,t187,t1877,t1885,t189,t1892,t1895,t1896,t1898,t1900,t1904,t1908,t1916,t1926,t1930,t1948,t1956,t196,t1960,t1964,t197,t1977,t1980,t1983,t1990,t2,t20,t2003,t2004,t2009,t2010,t2015,t2018,t2023,t2027,t2030,t2031,t204,t205,t2050,t2059,t2060,t208,t2099,t21,t210,t211,t2121,t2129,t2135,t2143,t2150,t2153,t2154,t2155,t2158,t2162,t2166,t2167,t217,t2174,t2175,t218,t2194,t2199,t22,t221,t223,t2238,t2243,t228,t2284,t2285,t2298,t23,t230,t231,t2317,t232,t2324,t2328,t233,t234,t2340,t235,t2354,t236,t237,t238,t239,t24,t240,t241,t242,t243,t244,t248,t25,t250,t251,t252,t253,t254,t255,t258,t259,t26,t261,t267,t268,t269,t27,t270,t271,t272,t273,t274,t275,t276,t277,t279,t28,t280,t281,t282,t283,t284,t285,t286,t287,t288,t289,t29,t290,t291,t292,t293,t294,t295,t296,t297,t298,t299,t3,t30,t301,t304,t305,t307,t308,t309,t31,t310,t311,t312,t313,t314,t315,t316,t317,t318,t319,t32,t320,t322,t324,t3248,t3249,t325,t3252,t327,t328,t329,t33,t330,t331,t332,t333,t334,t335,t336,t337,t338,t339,t34,t341,t342,t343,t344,t345,t346,t347,t348,t349,t35,t358,t359,t36,t360,t361,t362,t363,t364,t365,t366,t367,t368,t369,t37,t370,t371,t373,t374,t375,t376,t378,t380,t382,t385,t386,t387,t388,t389,t39,t390,t391,t392,t393,t394,t395,t396,t397,t398,t399,t4,t40,t400,t402,t405,t406,t407,t408,t409,t410,t411,t412,t413,t414,t415,t416,t417,t418,t419,t420,t425,t426,t427,t428,t429,t43,t431,t432,t433,t434,t435,t436,t438,t439,t441,t442,t443,t444,t446,t448,t45,t450,t451,t452,t453,t455,t456,t457,t458,t459,t46,t460,t461,t463,t464,t465,t466,t467,t468,t469,t470,t471,t472,t473,t474,t476,t477,t478,t479,t480,t481,t483,t484,t487,t488,t489,t49,t490,t494,t495,t496,t5,t50,t501,t502,t503,t504,t505,t506,t507,t508,t509,t51,t510,t511,t512,t513,t514,t515,t516,t517,t518,t519,t521,t522,t523,t524,t525,t526,t527,t528,t529,t530,t531,t533,t534,t535,t536,t537,t538,t542,t543,t544,t545,t546,t547,t548,t549,t55,t550,t551,t552,t553,t554,t556,t557,t558,t561,t562,t563,t564,t565,t566,t567,t568,t569,t57,t570,t571,t572,t573,t574,t575,t576,t577,t578,t579,t58,t580,t581,t582,t583,t584,t585,t586,t587,t588,t589,t590,t591,t592,t593,t594,t595,t596,t597,t598,t599,t6,t600,t601,t602,t603,t604,t605,t606,t607,t608,t609,t61,t611,t612,t613,t614,t615,t616,t617,t618,t619,t620,t621,t622,t623,t624,t626,t627,t628,t629,t63,t630,t631,t632,t633,t634,t635,t637,t638,t639,t64,t640,t642,t643,t644,t646,t647,t648,t649,t650,t651,t652,t653,t654,t655,t656,t657,t658,t660,t661,t662,t663,t664,t665,t666,t667,t668,t669,t67,t670,t671,t672,t673,t674,t675,t676,t677,t678,t679,t680,t681,t683,t684,t685,t686,t687,t688,t689,t69,t690,t691,t692,t693,t694,t695,t696,t697,t698,t699,t7,t70,t700,t701,t702,t703,t704,t705,t706,t707,t708,t709,t71,t710,t711,t712,t713,t714,t715,t716,t717,t718,t719,t72,t720,t721,t722,t723,t724,t725,t726,t727,t728,t729,t73,t730,t731,t732,t734,t735,t736,t737,t738,t74,t740,t741,t742,t743,t746,t747,t748,t749,t75,t750,t751,t752,t753,t754,t755,t756,t757,t758,t759,t76,t760,t761,t762,t765,t767,t769,t77,t770,t771,t772,t773,t774,t776,t777,t778,t779,t78,t780,t781,t785,t786,t787,t788,t789,t79,t791,t792,t794,t795,t8,t80,t802,t803,t804,t805,t806,t808,t809,t81,t810,t811,t815,t817,t818,t819,t82,t827,t83,t831,t833,t834,t835,t836,t837,t838,t839,t84,t840,t841,t842,t843,t845,t847,t85,t854,t855,t856,t857,t859,t86,t861,t862,t867,t868,t869,t87,t873,t875,t876,t88,t880,t881,t883,t886,t888,t889,t89,t890,t891,t892,t894,t898,t899,t9,t90,t900,t901,t902,t903,t905,t909,t91,t912,t913,t914,t915,t916,t917,t918,t919,t92,t920,t922,t924,t925,t934,t936,t938,t94,t940,t944,t945,t946,t948,t952,t959,t96,t965,t966,t969,t97,t971,t974,t975,t98,t982,t983,t987,t992,t994,t995,t999});
end
function C = ft_3(ct)
dq1 = ct{1};
dq2 = ct{2};
dq3 = ct{3};
dq4 = ct{4};
dq5 = ct{5};
dq6 = ct{6};
dq7 = ct{7};
t10 = ct{8};
t1001 = ct{9};
t101 = ct{10};
t1010 = ct{11};
t1019 = ct{12};
t1020 = ct{13};
t1021 = ct{14};
t1023 = ct{15};
t1024 = ct{16};
t1025 = ct{17};
t1026 = ct{18};
t1028 = ct{19};
t1029 = ct{20};
t1031 = ct{21};
t1032 = ct{22};
t1040 = ct{23};
t1044 = ct{24};
t1046 = ct{25};
t1047 = ct{26};
t1048 = ct{27};
t1049 = ct{28};
t105 = ct{29};
t1050 = ct{30};
t1057 = ct{31};
t1058 = ct{32};
t1066 = ct{33};
t1067 = ct{34};
t1068 = ct{35};
t1069 = ct{36};
t107 = ct{37};
t1070 = ct{38};
t1071 = ct{39};
t1072 = ct{40};
t1073 = ct{41};
t1074 = ct{42};
t1075 = ct{43};
t1076 = ct{44};
t1078 = ct{45};
t1079 = ct{46};
t1080 = ct{47};
t1082 = ct{48};
t1083 = ct{49};
t1084 = ct{50};
t1085 = ct{51};
t109 = ct{52};
t1096 = ct{53};
t1097 = ct{54};
t1098 = ct{55};
t11 = ct{56};
t110 = ct{57};
t1101 = ct{58};
t1102 = ct{59};
t1103 = ct{60};
t1104 = ct{61};
t1105 = ct{62};
t1106 = ct{63};
t1109 = ct{64};
t111 = ct{65};
t1110 = ct{66};
t1112 = ct{67};
t1113 = ct{68};
t1114 = ct{69};
t1115 = ct{70};
t1116 = ct{71};
t1117 = ct{72};
t1118 = ct{73};
t112 = ct{74};
t1120 = ct{75};
t1121 = ct{76};
t1122 = ct{77};
t1123 = ct{78};
t1124 = ct{79};
t1125 = ct{80};
t1126 = ct{81};
t1127 = ct{82};
t1128 = ct{83};
t1129 = ct{84};
t1130 = ct{85};
t1131 = ct{86};
t1132 = ct{87};
t1133 = ct{88};
t1134 = ct{89};
t1135 = ct{90};
t1136 = ct{91};
t1137 = ct{92};
t1138 = ct{93};
t1139 = ct{94};
t114 = ct{95};
t1140 = ct{96};
t1141 = ct{97};
t1142 = ct{98};
t1143 = ct{99};
t1144 = ct{100};
t1145 = ct{101};
t1146 = ct{102};
t1147 = ct{103};
t115 = ct{104};
t1155 = ct{105};
t1159 = ct{106};
t116 = ct{107};
t1161 = ct{108};
t1164 = ct{109};
t1165 = ct{110};
t1166 = ct{111};
t1167 = ct{112};
t1168 = ct{113};
t1169 = ct{114};
t117 = ct{115};
t1172 = ct{116};
t1173 = ct{117};
t1174 = ct{118};
t1175 = ct{119};
t1176 = ct{120};
t1177 = ct{121};
t1178 = ct{122};
t1179 = ct{123};
t1181 = ct{124};
t1182 = ct{125};
t1183 = ct{126};
t1184 = ct{127};
t1189 = ct{128};
t119 = ct{129};
t1190 = ct{130};
t1193 = ct{131};
t1194 = ct{132};
t1195 = ct{133};
t1197 = ct{134};
t1198 = ct{135};
t1199 = ct{136};
t12 = ct{137};
t1200 = ct{138};
t1201 = ct{139};
t1202 = ct{140};
t1203 = ct{141};
t1204 = ct{142};
t1205 = ct{143};
t1208 = ct{144};
t1210 = ct{145};
t1214 = ct{146};
t1217 = ct{147};
t1218 = ct{148};
t122 = ct{149};
t1223 = ct{150};
t1225 = ct{151};
t1232 = ct{152};
t1234 = ct{153};
t124 = ct{154};
t1249 = ct{155};
t125 = ct{156};
t1250 = ct{157};
t1253 = ct{158};
t1256 = ct{159};
t1257 = ct{160};
t126 = ct{161};
t1263 = ct{162};
t1264 = ct{163};
t1265 = ct{164};
t1266 = ct{165};
t1267 = ct{166};
t1268 = ct{167};
t127 = ct{168};
t1270 = ct{169};
t1275 = ct{170};
t1276 = ct{171};
t1277 = ct{172};
t1278 = ct{173};
t1280 = ct{174};
t1283 = ct{175};
t1284 = ct{176};
t1286 = ct{177};
t1287 = ct{178};
t1288 = ct{179};
t1289 = ct{180};
t1291 = ct{181};
t1292 = ct{182};
t1293 = ct{183};
t1294 = ct{184};
t1296 = ct{185};
t1299 = ct{186};
t13 = ct{187};
t130 = ct{188};
t1300 = ct{189};
t1304 = ct{190};
t1305 = ct{191};
t1306 = ct{192};
t1307 = ct{193};
t1308 = ct{194};
t131 = ct{195};
t1310 = ct{196};
t1312 = ct{197};
t1313 = ct{198};
t1315 = ct{199};
t1316 = ct{200};
t1317 = ct{201};
t1326 = ct{202};
t1327 = ct{203};
t1328 = ct{204};
t1331 = ct{205};
t1332 = ct{206};
t1333 = ct{207};
t1334 = ct{208};
t1335 = ct{209};
t1339 = ct{210};
t1341 = ct{211};
t1342 = ct{212};
t1343 = ct{213};
t1344 = ct{214};
t1346 = ct{215};
t1347 = ct{216};
t1348 = ct{217};
t1349 = ct{218};
t135 = ct{219};
t1350 = ct{220};
t1351 = ct{221};
t1352 = ct{222};
t1355 = ct{223};
t1356 = ct{224};
t1357 = ct{225};
t1358 = ct{226};
t1359 = ct{227};
t136 = ct{228};
t1360 = ct{229};
t1361 = ct{230};
t1362 = ct{231};
t1363 = ct{232};
t1364 = ct{233};
t1365 = ct{234};
t1368 = ct{235};
t1369 = ct{236};
t137 = ct{237};
t1376 = ct{238};
t1377 = ct{239};
t1380 = ct{240};
t1381 = ct{241};
t1382 = ct{242};
t1384 = ct{243};
t1385 = ct{244};
t1388 = ct{245};
t1389 = ct{246};
t139 = ct{247};
t1390 = ct{248};
t1391 = ct{249};
t1396 = ct{250};
t1397 = ct{251};
t14 = ct{252};
t140 = ct{253};
t1400 = ct{254};
t1401 = ct{255};
t1402 = ct{256};
t1406 = ct{257};
t1410 = ct{258};
t1412 = ct{259};
t1416 = ct{260};
t1417 = ct{261};
t1418 = ct{262};
t1421 = ct{263};
t1422 = ct{264};
t1423 = ct{265};
t1425 = ct{266};
t1428 = ct{267};
t1429 = ct{268};
t1430 = ct{269};
t1431 = ct{270};
t1432 = ct{271};
t1435 = ct{272};
t1436 = ct{273};
t1438 = ct{274};
t1439 = ct{275};
t144 = ct{276};
t1440 = ct{277};
t1441 = ct{278};
t1445 = ct{279};
t1446 = ct{280};
t1449 = ct{281};
t1450 = ct{282};
t1451 = ct{283};
t1452 = ct{284};
t1453 = ct{285};
t1454 = ct{286};
t1455 = ct{287};
t1456 = ct{288};
t1457 = ct{289};
t1458 = ct{290};
t1459 = ct{291};
t1460 = ct{292};
t1461 = ct{293};
t1463 = ct{294};
t1467 = ct{295};
t147 = ct{296};
t1474 = ct{297};
t1475 = ct{298};
t1480 = ct{299};
t1483 = ct{300};
t1485 = ct{301};
t1486 = ct{302};
t149 = ct{303};
t1490 = ct{304};
t1491 = ct{305};
t1492 = ct{306};
t1495 = ct{307};
t1496 = ct{308};
t1497 = ct{309};
t1498 = ct{310};
t1499 = ct{311};
t15 = ct{312};
t1504 = ct{313};
t1505 = ct{314};
t1506 = ct{315};
t1508 = ct{316};
t1509 = ct{317};
t151 = ct{318};
t1510 = ct{319};
t1511 = ct{320};
t1512 = ct{321};
t1513 = ct{322};
t1517 = ct{323};
t1518 = ct{324};
t1519 = ct{325};
t152 = ct{326};
t1521 = ct{327};
t1522 = ct{328};
t1523 = ct{329};
t1524 = ct{330};
t1525 = ct{331};
t1533 = ct{332};
t1534 = ct{333};
t1537 = ct{334};
t1538 = ct{335};
t1539 = ct{336};
t1540 = ct{337};
t1541 = ct{338};
t1542 = ct{339};
t1543 = ct{340};
t1544 = ct{341};
t1545 = ct{342};
t1546 = ct{343};
t1547 = ct{344};
t1548 = ct{345};
t1549 = ct{346};
t1550 = ct{347};
t1551 = ct{348};
t1552 = ct{349};
t1553 = ct{350};
t1554 = ct{351};
t1556 = ct{352};
t1558 = ct{353};
t1559 = ct{354};
t156 = ct{355};
t1560 = ct{356};
t1561 = ct{357};
t1562 = ct{358};
t1563 = ct{359};
t1565 = ct{360};
t1566 = ct{361};
t1567 = ct{362};
t1568 = ct{363};
t1569 = ct{364};
t157 = ct{365};
t1570 = ct{366};
t1571 = ct{367};
t1572 = ct{368};
t1573 = ct{369};
t1574 = ct{370};
t1575 = ct{371};
t1576 = ct{372};
t1577 = ct{373};
t158 = ct{374};
t1591 = ct{375};
t1592 = ct{376};
t1593 = ct{377};
t1596 = ct{378};
t1597 = ct{379};
t1599 = ct{380};
t16 = ct{381};
t160 = ct{382};
t1600 = ct{383};
t1602 = ct{384};
t1603 = ct{385};
t1605 = ct{386};
t1616 = ct{387};
t162 = ct{388};
t1622 = ct{389};
t1627 = ct{390};
t1628 = ct{391};
t1629 = ct{392};
t163 = ct{393};
t1630 = ct{394};
t1634 = ct{395};
t1635 = ct{396};
t1636 = ct{397};
t1638 = ct{398};
t1639 = ct{399};
t1640 = ct{400};
t1643 = ct{401};
t1644 = ct{402};
t1648 = ct{403};
t165 = ct{404};
t166 = ct{405};
t1661 = ct{406};
t1664 = ct{407};
t1665 = ct{408};
t1666 = ct{409};
t1667 = ct{410};
t167 = ct{411};
t1674 = ct{412};
t1675 = ct{413};
t1676 = ct{414};
t168 = ct{415};
t1683 = ct{416};
t1684 = ct{417};
t1694 = ct{418};
t1696 = ct{419};
t1698 = ct{420};
t17 = ct{421};
t1701 = ct{422};
t1704 = ct{423};
t1708 = ct{424};
t171 = ct{425};
t1713 = ct{426};
t1715 = ct{427};
t1717 = ct{428};
t1723 = ct{429};
t1734 = ct{430};
t1735 = ct{431};
t1736 = ct{432};
t1739 = ct{433};
t1740 = ct{434};
t1741 = ct{435};
t1744 = ct{436};
t1747 = ct{437};
t1748 = ct{438};
t175 = ct{439};
t1751 = ct{440};
t1754 = ct{441};
t1756 = ct{442};
t1758 = ct{443};
t1760 = ct{444};
t1768 = ct{445};
t1772 = ct{446};
t1788 = ct{447};
t1789 = ct{448};
t1791 = ct{449};
t180 = ct{450};
t1807 = ct{451};
t181 = ct{452};
t1814 = ct{453};
t1819 = ct{454};
t182 = ct{455};
t1820 = ct{456};
t1821 = ct{457};
t1827 = ct{458};
t1831 = ct{459};
t1834 = ct{460};
t185 = ct{461};
t1852 = ct{462};
t186 = ct{463};
t187 = ct{464};
t1877 = ct{465};
t1885 = ct{466};
t189 = ct{467};
t1892 = ct{468};
t1895 = ct{469};
t1896 = ct{470};
t1898 = ct{471};
t1900 = ct{472};
t1904 = ct{473};
t1908 = ct{474};
t1916 = ct{475};
t1926 = ct{476};
t1930 = ct{477};
t1948 = ct{478};
t1956 = ct{479};
t196 = ct{480};
t1960 = ct{481};
t1964 = ct{482};
t197 = ct{483};
t1977 = ct{484};
t1980 = ct{485};
t1983 = ct{486};
t1990 = ct{487};
t2 = ct{488};
t20 = ct{489};
t2003 = ct{490};
t2004 = ct{491};
t2009 = ct{492};
t2010 = ct{493};
t2015 = ct{494};
t2018 = ct{495};
t2023 = ct{496};
t2027 = ct{497};
t2030 = ct{498};
t2031 = ct{499};
t204 = ct{500};
t205 = ct{501};
t2050 = ct{502};
t2059 = ct{503};
t2060 = ct{504};
t208 = ct{505};
t2099 = ct{506};
t21 = ct{507};
t210 = ct{508};
t211 = ct{509};
t2121 = ct{510};
t2129 = ct{511};
t2135 = ct{512};
t2143 = ct{513};
t2150 = ct{514};
t2153 = ct{515};
t2154 = ct{516};
t2155 = ct{517};
t2158 = ct{518};
t2162 = ct{519};
t2166 = ct{520};
t2167 = ct{521};
t217 = ct{522};
t2174 = ct{523};
t2175 = ct{524};
t218 = ct{525};
t2194 = ct{526};
t2199 = ct{527};
t22 = ct{528};
t221 = ct{529};
t223 = ct{530};
t2238 = ct{531};
t2243 = ct{532};
t228 = ct{533};
t2284 = ct{534};
t2285 = ct{535};
t2298 = ct{536};
t23 = ct{537};
t230 = ct{538};
t231 = ct{539};
t2317 = ct{540};
t232 = ct{541};
t2324 = ct{542};
t2328 = ct{543};
t233 = ct{544};
t234 = ct{545};
t2340 = ct{546};
t235 = ct{547};
t2354 = ct{548};
t236 = ct{549};
t237 = ct{550};
t238 = ct{551};
t239 = ct{552};
t24 = ct{553};
t240 = ct{554};
t241 = ct{555};
t242 = ct{556};
t243 = ct{557};
t244 = ct{558};
t248 = ct{559};
t25 = ct{560};
t250 = ct{561};
t251 = ct{562};
t252 = ct{563};
t253 = ct{564};
t254 = ct{565};
t255 = ct{566};
t258 = ct{567};
t259 = ct{568};
t26 = ct{569};
t261 = ct{570};
t267 = ct{571};
t268 = ct{572};
t269 = ct{573};
t27 = ct{574};
t270 = ct{575};
t271 = ct{576};
t272 = ct{577};
t273 = ct{578};
t274 = ct{579};
t275 = ct{580};
t276 = ct{581};
t277 = ct{582};
t279 = ct{583};
t28 = ct{584};
t280 = ct{585};
t281 = ct{586};
t282 = ct{587};
t283 = ct{588};
t284 = ct{589};
t285 = ct{590};
t286 = ct{591};
t287 = ct{592};
t288 = ct{593};
t289 = ct{594};
t29 = ct{595};
t290 = ct{596};
t291 = ct{597};
t292 = ct{598};
t293 = ct{599};
t294 = ct{600};
t295 = ct{601};
t296 = ct{602};
t297 = ct{603};
t298 = ct{604};
t299 = ct{605};
t3 = ct{606};
t30 = ct{607};
t301 = ct{608};
t304 = ct{609};
t305 = ct{610};
t307 = ct{611};
t308 = ct{612};
t309 = ct{613};
t31 = ct{614};
t310 = ct{615};
t311 = ct{616};
t312 = ct{617};
t313 = ct{618};
t314 = ct{619};
t315 = ct{620};
t316 = ct{621};
t317 = ct{622};
t318 = ct{623};
t319 = ct{624};
t32 = ct{625};
t320 = ct{626};
t322 = ct{627};
t324 = ct{628};
t3248 = ct{629};
t3249 = ct{630};
t325 = ct{631};
t3252 = ct{632};
t327 = ct{633};
t328 = ct{634};
t329 = ct{635};
t33 = ct{636};
t330 = ct{637};
t331 = ct{638};
t332 = ct{639};
t333 = ct{640};
t334 = ct{641};
t335 = ct{642};
t336 = ct{643};
t337 = ct{644};
t338 = ct{645};
t339 = ct{646};
t34 = ct{647};
t341 = ct{648};
t342 = ct{649};
t343 = ct{650};
t344 = ct{651};
t345 = ct{652};
t346 = ct{653};
t347 = ct{654};
t348 = ct{655};
t349 = ct{656};
t35 = ct{657};
t358 = ct{658};
t359 = ct{659};
t36 = ct{660};
t360 = ct{661};
t361 = ct{662};
t362 = ct{663};
t363 = ct{664};
t364 = ct{665};
t365 = ct{666};
t366 = ct{667};
t367 = ct{668};
t368 = ct{669};
t369 = ct{670};
t37 = ct{671};
t370 = ct{672};
t371 = ct{673};
t373 = ct{674};
t374 = ct{675};
t375 = ct{676};
t376 = ct{677};
t378 = ct{678};
t380 = ct{679};
t382 = ct{680};
t385 = ct{681};
t386 = ct{682};
t387 = ct{683};
t388 = ct{684};
t389 = ct{685};
t39 = ct{686};
t390 = ct{687};
t391 = ct{688};
t392 = ct{689};
t393 = ct{690};
t394 = ct{691};
t395 = ct{692};
t396 = ct{693};
t397 = ct{694};
t398 = ct{695};
t399 = ct{696};
t4 = ct{697};
t40 = ct{698};
t400 = ct{699};
t402 = ct{700};
t405 = ct{701};
t406 = ct{702};
t407 = ct{703};
t408 = ct{704};
t409 = ct{705};
t410 = ct{706};
t411 = ct{707};
t412 = ct{708};
t413 = ct{709};
t414 = ct{710};
t415 = ct{711};
t416 = ct{712};
t417 = ct{713};
t418 = ct{714};
t419 = ct{715};
t420 = ct{716};
t425 = ct{717};
t426 = ct{718};
t427 = ct{719};
t428 = ct{720};
t429 = ct{721};
t43 = ct{722};
t431 = ct{723};
t432 = ct{724};
t433 = ct{725};
t434 = ct{726};
t435 = ct{727};
t436 = ct{728};
t438 = ct{729};
t439 = ct{730};
t441 = ct{731};
t442 = ct{732};
t443 = ct{733};
t444 = ct{734};
t446 = ct{735};
t448 = ct{736};
t45 = ct{737};
t450 = ct{738};
t451 = ct{739};
t452 = ct{740};
t453 = ct{741};
t455 = ct{742};
t456 = ct{743};
t457 = ct{744};
t458 = ct{745};
t459 = ct{746};
t46 = ct{747};
t460 = ct{748};
t461 = ct{749};
t463 = ct{750};
t464 = ct{751};
t465 = ct{752};
t466 = ct{753};
t467 = ct{754};
t468 = ct{755};
t469 = ct{756};
t470 = ct{757};
t471 = ct{758};
t472 = ct{759};
t473 = ct{760};
t474 = ct{761};
t476 = ct{762};
t477 = ct{763};
t478 = ct{764};
t479 = ct{765};
t480 = ct{766};
t481 = ct{767};
t483 = ct{768};
t484 = ct{769};
t487 = ct{770};
t488 = ct{771};
t489 = ct{772};
t49 = ct{773};
t490 = ct{774};
t494 = ct{775};
t495 = ct{776};
t496 = ct{777};
t5 = ct{778};
t50 = ct{779};
t501 = ct{780};
t502 = ct{781};
t503 = ct{782};
t504 = ct{783};
t505 = ct{784};
t506 = ct{785};
t507 = ct{786};
t508 = ct{787};
t509 = ct{788};
t51 = ct{789};
t510 = ct{790};
t511 = ct{791};
t512 = ct{792};
t513 = ct{793};
t514 = ct{794};
t515 = ct{795};
t516 = ct{796};
t517 = ct{797};
t518 = ct{798};
t519 = ct{799};
t521 = ct{800};
t522 = ct{801};
t523 = ct{802};
t524 = ct{803};
t525 = ct{804};
t526 = ct{805};
t527 = ct{806};
t528 = ct{807};
t529 = ct{808};
t530 = ct{809};
t531 = ct{810};
t533 = ct{811};
t534 = ct{812};
t535 = ct{813};
t536 = ct{814};
t537 = ct{815};
t538 = ct{816};
t542 = ct{817};
t543 = ct{818};
t544 = ct{819};
t545 = ct{820};
t546 = ct{821};
t547 = ct{822};
t548 = ct{823};
t549 = ct{824};
t55 = ct{825};
t550 = ct{826};
t551 = ct{827};
t552 = ct{828};
t553 = ct{829};
t554 = ct{830};
t556 = ct{831};
t557 = ct{832};
t558 = ct{833};
t561 = ct{834};
t562 = ct{835};
t563 = ct{836};
t564 = ct{837};
t565 = ct{838};
t566 = ct{839};
t567 = ct{840};
t568 = ct{841};
t569 = ct{842};
t57 = ct{843};
t570 = ct{844};
t571 = ct{845};
t572 = ct{846};
t573 = ct{847};
t574 = ct{848};
t575 = ct{849};
t576 = ct{850};
t577 = ct{851};
t578 = ct{852};
t579 = ct{853};
t58 = ct{854};
t580 = ct{855};
t581 = ct{856};
t582 = ct{857};
t583 = ct{858};
t584 = ct{859};
t585 = ct{860};
t586 = ct{861};
t587 = ct{862};
t588 = ct{863};
t589 = ct{864};
t590 = ct{865};
t591 = ct{866};
t592 = ct{867};
t593 = ct{868};
t594 = ct{869};
t595 = ct{870};
t596 = ct{871};
t597 = ct{872};
t598 = ct{873};
t599 = ct{874};
t6 = ct{875};
t600 = ct{876};
t601 = ct{877};
t602 = ct{878};
t603 = ct{879};
t604 = ct{880};
t605 = ct{881};
t606 = ct{882};
t607 = ct{883};
t608 = ct{884};
t609 = ct{885};
t61 = ct{886};
t611 = ct{887};
t612 = ct{888};
t613 = ct{889};
t614 = ct{890};
t615 = ct{891};
t616 = ct{892};
t617 = ct{893};
t618 = ct{894};
t619 = ct{895};
t620 = ct{896};
t621 = ct{897};
t622 = ct{898};
t623 = ct{899};
t624 = ct{900};
t626 = ct{901};
t627 = ct{902};
t628 = ct{903};
t629 = ct{904};
t63 = ct{905};
t630 = ct{906};
t631 = ct{907};
t632 = ct{908};
t633 = ct{909};
t634 = ct{910};
t635 = ct{911};
t637 = ct{912};
t638 = ct{913};
t639 = ct{914};
t64 = ct{915};
t640 = ct{916};
t642 = ct{917};
t643 = ct{918};
t644 = ct{919};
t646 = ct{920};
t647 = ct{921};
t648 = ct{922};
t649 = ct{923};
t650 = ct{924};
t651 = ct{925};
t652 = ct{926};
t653 = ct{927};
t654 = ct{928};
t655 = ct{929};
t656 = ct{930};
t657 = ct{931};
t658 = ct{932};
t660 = ct{933};
t661 = ct{934};
t662 = ct{935};
t663 = ct{936};
t664 = ct{937};
t665 = ct{938};
t666 = ct{939};
t667 = ct{940};
t668 = ct{941};
t669 = ct{942};
t67 = ct{943};
t670 = ct{944};
t671 = ct{945};
t672 = ct{946};
t673 = ct{947};
t674 = ct{948};
t675 = ct{949};
t676 = ct{950};
t677 = ct{951};
t678 = ct{952};
t679 = ct{953};
t680 = ct{954};
t681 = ct{955};
t683 = ct{956};
t684 = ct{957};
t685 = ct{958};
t686 = ct{959};
t687 = ct{960};
t688 = ct{961};
t689 = ct{962};
t69 = ct{963};
t690 = ct{964};
t691 = ct{965};
t692 = ct{966};
t693 = ct{967};
t694 = ct{968};
t695 = ct{969};
t696 = ct{970};
t697 = ct{971};
t698 = ct{972};
t699 = ct{973};
t7 = ct{974};
t70 = ct{975};
t700 = ct{976};
t701 = ct{977};
t702 = ct{978};
t703 = ct{979};
t704 = ct{980};
t705 = ct{981};
t706 = ct{982};
t707 = ct{983};
t708 = ct{984};
t709 = ct{985};
t71 = ct{986};
t710 = ct{987};
t711 = ct{988};
t712 = ct{989};
t713 = ct{990};
t714 = ct{991};
t715 = ct{992};
t716 = ct{993};
t717 = ct{994};
t718 = ct{995};
t719 = ct{996};
t72 = ct{997};
t720 = ct{998};
t721 = ct{999};
t722 = ct{1000};
t723 = ct{1001};
t724 = ct{1002};
t725 = ct{1003};
t726 = ct{1004};
t727 = ct{1005};
t728 = ct{1006};
t729 = ct{1007};
t73 = ct{1008};
t730 = ct{1009};
t731 = ct{1010};
t732 = ct{1011};
t734 = ct{1012};
t735 = ct{1013};
t736 = ct{1014};
t737 = ct{1015};
t738 = ct{1016};
t74 = ct{1017};
t740 = ct{1018};
t741 = ct{1019};
t742 = ct{1020};
t743 = ct{1021};
t746 = ct{1022};
t747 = ct{1023};
t748 = ct{1024};
t749 = ct{1025};
t75 = ct{1026};
t750 = ct{1027};
t751 = ct{1028};
t752 = ct{1029};
t753 = ct{1030};
t754 = ct{1031};
t755 = ct{1032};
t756 = ct{1033};
t757 = ct{1034};
t758 = ct{1035};
t759 = ct{1036};
t76 = ct{1037};
t760 = ct{1038};
t761 = ct{1039};
t762 = ct{1040};
t765 = ct{1041};
t767 = ct{1042};
t769 = ct{1043};
t77 = ct{1044};
t770 = ct{1045};
t771 = ct{1046};
t772 = ct{1047};
t773 = ct{1048};
t774 = ct{1049};
t776 = ct{1050};
t777 = ct{1051};
t778 = ct{1052};
t779 = ct{1053};
t78 = ct{1054};
t780 = ct{1055};
t781 = ct{1056};
t785 = ct{1057};
t786 = ct{1058};
t787 = ct{1059};
t788 = ct{1060};
t789 = ct{1061};
t79 = ct{1062};
t791 = ct{1063};
t792 = ct{1064};
t794 = ct{1065};
t795 = ct{1066};
t8 = ct{1067};
t80 = ct{1068};
t802 = ct{1069};
t803 = ct{1070};
t804 = ct{1071};
t805 = ct{1072};
t806 = ct{1073};
t808 = ct{1074};
t809 = ct{1075};
t81 = ct{1076};
t810 = ct{1077};
t811 = ct{1078};
t815 = ct{1079};
t817 = ct{1080};
t818 = ct{1081};
t819 = ct{1082};
t82 = ct{1083};
t827 = ct{1084};
t83 = ct{1085};
t831 = ct{1086};
t833 = ct{1087};
t834 = ct{1088};
t835 = ct{1089};
t836 = ct{1090};
t837 = ct{1091};
t838 = ct{1092};
t839 = ct{1093};
t84 = ct{1094};
t840 = ct{1095};
t841 = ct{1096};
t842 = ct{1097};
t843 = ct{1098};
t845 = ct{1099};
t847 = ct{1100};
t85 = ct{1101};
t854 = ct{1102};
t855 = ct{1103};
t856 = ct{1104};
t857 = ct{1105};
t859 = ct{1106};
t86 = ct{1107};
t861 = ct{1108};
t862 = ct{1109};
t867 = ct{1110};
t868 = ct{1111};
t869 = ct{1112};
t87 = ct{1113};
t873 = ct{1114};
t875 = ct{1115};
t876 = ct{1116};
t88 = ct{1117};
t880 = ct{1118};
t881 = ct{1119};
t883 = ct{1120};
t886 = ct{1121};
t888 = ct{1122};
t889 = ct{1123};
t89 = ct{1124};
t890 = ct{1125};
t891 = ct{1126};
t892 = ct{1127};
t894 = ct{1128};
t898 = ct{1129};
t899 = ct{1130};
t9 = ct{1131};
t90 = ct{1132};
t900 = ct{1133};
t901 = ct{1134};
t902 = ct{1135};
t903 = ct{1136};
t905 = ct{1137};
t909 = ct{1138};
t91 = ct{1139};
t912 = ct{1140};
t913 = ct{1141};
t914 = ct{1142};
t915 = ct{1143};
t916 = ct{1144};
t917 = ct{1145};
t918 = ct{1146};
t919 = ct{1147};
t92 = ct{1148};
t920 = ct{1149};
t922 = ct{1150};
t924 = ct{1151};
t925 = ct{1152};
t934 = ct{1153};
t936 = ct{1154};
t938 = ct{1155};
t94 = ct{1156};
t940 = ct{1157};
t944 = ct{1158};
t945 = ct{1159};
t946 = ct{1160};
t948 = ct{1161};
t952 = ct{1162};
t959 = ct{1163};
t96 = ct{1164};
t965 = ct{1165};
t966 = ct{1166};
t969 = ct{1167};
t97 = ct{1168};
t971 = ct{1169};
t974 = ct{1170};
t975 = ct{1171};
t98 = ct{1172};
t982 = ct{1173};
t983 = ct{1174};
t987 = ct{1175};
t992 = ct{1176};
t994 = ct{1177};
t995 = ct{1178};
t999 = ct{1179};
t1836 = t760.*1.9738e-1;
t1837 = t767.*1.9738e-1;
t1840 = t1020.*(t86-t652);
t1849 = t15.*(t650+t7.*(t643-t662));
t1863 = t163+t167+t293+t296+t299+t304+t521;
t1868 = t948.*(-2.75e-2);
t1870 = dq5.*t6.*(t86-t652).*(-2.37e-3);
t1879 = -t1066.*(t86-t652);
t1881 = t948.*2.75e-2;
t1887 = dq5.*t6.*(t86-t652).*2.37e-3;
t1893 = t127+t136+t279+t280+t345+t513+t514;
t1897 = dq5.*t6.*(t86-t652).*(-2.75e-2);
t1901 = t7.*t1852;
t1905 = t14.*t1852;
t1928 = dq6.*t14.*(t86-t652).*(-2.019e-2);
t1934 = t999.*(-2.019e-2);
t1937 = dq5.*t13.*(t86-t652).*(-5.000000000000001e-5);
t1944 = t6.*t1885;
t1945 = t13.*t1885;
t1946 = dq7.*t8.*(t92-t663).*(-3.466000000000001e-2);
t1947 = -t1930;
t1949 = t6.*t1892;
t1951 = t13.*t1892;
t1952 = t7.*t1896;
t1955 = t14.*t1896;
t1958 = t6.*t20.*(t86-t652).*(-5.000000000000001e-5);
t1965 = -t1948;
t1966 = -t1956;
t1967 = t6.*t20.*(t86-t652).*5.000000000000001e-5;
t1968 = t1049.*1.8866e-1;
t1973 = -t1964;
t1979 = dq7.*t7.*t8.*(t92-t663).*(-2.324e-2);
t1981 = dq4.*t1047.*3.7732e-1;
t1982 = t8.*t22.*(t92-t663).*(-2.324e-2);
t1987 = t999.*(-1.9738e-1);
t1989 = t1048.*2.37e-3;
t1991 = t1079.*1.8866e-1;
t1995 = dq6.*t14.*(t86-t652).*(-1.9738e-1);
t1996 = dq6.*t7.*(t92-t663).*(-1.9738e-1);
t1998 = t999.*1.9738e-1;
t1999 = t1020.*t1066;
t2008 = t1048.*2.75e-2;
t2011 = dq7.*t8.*(t252-t791).*(-3.466000000000001e-2);
t2014 = t1076.*2.37e-3;
t2016 = t1049.*5.267999999999999e-2;
t2020 = dq4.*t1047.*1.0536e-1;
t2024 = t1040.*t1067;
t2026 = t1050.*5.000000000000001e-5;
t2028 = dq5.*t1080.*4.74e-3;
t2032 = t1076.*2.75e-2;
t2034 = dq7.*t15.*(t252-t791).*(-2.324e-2);
t2038 = t1047.*2.0e-4;
t2042 = dq5.*t1080.*5.5e-2;
t2049 = dq7.*t15.*(t252-t791).*2.324e-2;
t2056 = t1069.*t1070;
t2061 = dq4.*t1049.*4.0e-4;
t2069 = t1080.*5.000000000000001e-5;
t2078 = dq5.*t1076.*1.0e-4;
t2127 = t204+t210+t218+t360+t363+t366+t371+t374+t488;
t2128 = t205+t211+t217+t359+t362+t365+t375+t376+t487;
t2136 = t196+t197+t261+t392+t396+t398+t409+t410+t474;
t2149 = t131+t135+t344+t630+t1112;
t2168 = t228+t385+t388+t391+t400+t405+t413+t414+t471;
t2169 = -t2154;
t2189 = t255+t367+t369+t370+t380+t382+t425+t426+t490;
t2252 = -t2238;
t2271 = t5.*t2199;
t2272 = -t2243;
t2274 = t12.*t2199;
t2293 = dq7.*t8.*(t614+t13.*(t86-t652)).*(-3.466000000000001e-2);
t2296 = t622+t707+t867+t875;
t2318 = t868.*7.000000000000001e-5;
t2322 = dq7.*t7.*t8.*(t614+t13.*(t86-t652)).*(-2.324e-2);
t2325 = t8.*t22.*(t614+t13.*(t86-t652)).*(-2.324e-2);
t2331 = -t2324;
t2332 = t868.*4.999999999999997e-5;
t2333 = t8.*t22.*(t614+t13.*(t86-t652)).*2.324e-2;
t2334 = dq6.*t7.*(t614+t13.*(t86-t652)).*(-1.9738e-1);
t2335 = t912.*7.000000000000022e-5;
t2336 = -t2328;
t2337 = t868.*2.23e-3;
t2341 = t859.*1.11e-3;
t2347 = -t2340;
t2349 = t912.*4.999999999999997e-5;
t2361 = -t2354;
t2364 = t912.*2.19e-3;
t2365 = t859.*8.8e-4;
t2373 = t572.*t2199;
t2381 = t1057.*7.000000000000022e-5;
t2386 = t1071.*7.000000000000022e-5;
t2387 = dq7.*t8.*(t650+t7.*(t643-t662)).*(-2.324e-2);
t2388 = t859.*1.144e-2;
t2389 = t1057.*4.999999999999997e-5;
t2393 = t1072.*7.000000000000001e-5;
t2396 = t1071.*4.999999999999997e-5;
t2401 = t1124.*7.000000000000001e-5;
t2402 = t1072.*4.999999999999997e-5;
t2404 = t1072.*2.23e-3;
t2405 = t1181.*7.000000000000001e-5;
t2406 = t1182.*7.000000000000001e-5;
t2408 = t1057.*2.19e-3;
t2409 = t1083.*1.11e-3;
t2410 = t1124.*4.999999999999997e-5;
t2415 = t1071.*2.19e-3;
t2420 = t1181.*4.999999999999997e-5;
t2421 = t1182.*4.999999999999997e-5;
t2423 = t1124.*2.23e-3;
t2432 = t1181.*2.23e-3;
t2433 = t1182.*2.23e-3;
t2440 = t1083.*8.8e-4;
t2450 = t1499.*7.000000000000001e-5;
t2452 = t1499.*7.000000000000022e-5;
t2468 = t1592.*7.000000000000022e-5;
t2472 = t1083.*1.144e-2;
t2478 = t1592.*4.999999999999997e-5;
t2480 = t1499.*7.299999999999999e-4;
t2493 = t1592.*2.19e-3;
t2494 = t1627.*1.11e-3;
t2534 = t1627.*1.12e-3;
t2622 = t1627.*4.988e-2;
t2678 = t1066.*(t86-t652).*(-1.11e-3);
t2696 = t1066.*(t86-t652).*(-8.8e-4);
t2730 = t1066.*(t86-t652).*(-1.144e-2);
t3672 = t1266+t1276+t1283+t1284+t1316+t1317+t1333+t1334+t1335+t1358+t1359+t1438+t1439+t1440+t1454+t1458+t1459+t1460+t1461+t1533+t1534;
t3673 = t1234+t1278+t1280+t1307+t1308+t1326+t1331+t1332+t1355+t1400+t1401+t1402+t1406+t1445+t1446+t1457+t1521+t1522+t1523+t1575+t1576;
t3679 = t558+t1294+t1310+t1343+t1344+t1396+t1397+t1421+t1422+t1452+t1463+t1483+t1485+t1486+t1504+t1505+t1524+t1525+t1558+t1559+t1560+t1573;
t744 = -t672;
t745 = -t673;
t763 = t5.*t712;
t764 = -t690;
t766 = -t692;
t775 = t5.*t670;
t782 = -t742;
t783 = -t718;
t784 = t668.*(2.0./5.0);
t790 = -t726;
t796 = t709.*(2.0./5.0);
t798 = -t746;
t799 = t20.*t738;
t800 = -t789;
t801 = -t752;
t812 = -t776;
t813 = -t779;
t816 = t749.*(2.0./5.0);
t820 = -t804;
t821 = -t806;
t822 = -t808;
t846 = t831.^2;
t848 = dq7.*t834;
t849 = dq5.*t835;
t850 = dq6.*t836;
t851 = dq7.*t837;
t852 = dq5.*t838;
t853 = dq6.*t839;
t860 = t7.*t831;
t863 = t14.*t831;
t864 = t7.*t827;
t866 = t8.*t827;
t870 = t14.*t827;
t871 = t15.*t827;
t872 = t20.*t838;
t877 = dq5.*t6.*t831;
t882 = dq5.*t13.*t831;
t904 = t20.*t835;
t908 = t8.*t13.*t831;
t911 = t13.*t15.*t831;
t931 = t6.*t883;
t937 = t6.*t894;
t941 = dq5.*t914;
t942 = dq6.*t915;
t947 = dq5.*t917;
t950 = dq6.*t918;
t953 = dq7.*t919;
t954 = -t888;
t955 = -t890;
t958 = dq7.*t920;
t968 = t7.*t919;
t970 = t7.*t920;
t972 = t889.*(2.0./5.0);
t973 = t899.*(2.0./5.0);
t977 = t22.*t920;
t978 = dq7.*t974;
t979 = dq7.*t975;
t989 = dq6.*t14.*t919;
t993 = dq6.*t14.*t920;
t997 = t20.*t914;
t998 = t20.*t917;
t1000 = t22.*t919;
t1003 = t7.*t940;
t1004 = t14.*t940;
t1007 = t7.*t959;
t1008 = t14.*t959;
t1009 = -t975;
t1016 = t8.*t994;
t1017 = t7.*t995;
t1018 = t15.*t994;
t1022 = t613+t730;
t1034 = dq7.*t1028;
t1036 = dq7.*t1029;
t1038 = dq7.*t1031;
t1039 = dq7.*t1032;
t1042 = t662+t727;
t1043 = t657+t732;
t1045 = dq7.*t1044;
t1052 = t8.*t1023;
t1053 = t8.*t1024;
t1055 = t15.*t1023;
t1056 = t15.*t1024;
t1089 = dq6.*t1078;
t1094 = dq6.*t1082;
t1099 = -t1084;
t1100 = -t1085;
t1111 = -t1096;
t1119 = -t1097;
t1180 = -t1155;
t1185 = dq4.*t1127.*2.0;
t1186 = dq5.*t1128.*2.0;
t1187 = dq5.*t1131.*2.0;
t1188 = dq6.*t1132.*2.0;
t1191 = dq6.*t1137.*2.0;
t1206 = t661+t835;
t1209 = t6.*t1115;
t1211 = t13.*t1115;
t1212 = t7.*t1126;
t1213 = t7.*t1130;
t1215 = t14.*t1126;
t1216 = -t1114;
t1219 = t14.*t1130;
t1220 = t8.*t1136;
t1221 = -t1116;
t1222 = -t1122;
t1224 = -t1125;
t1226 = t15.*t1136;
t1227 = -t1129;
t1228 = -t1132;
t1229 = -t1134;
t1231 = -t1172;
t1237 = dq4.*t1116.*2.0;
t1238 = dq5.*t1117.*2.0;
t1239 = dq5.*t1120.*2.0;
t1269 = t1116.*(2.0./5.0);
t1273 = t1126.*(2.0./5.0);
t1274 = t1127.*(2.0./5.0);
t1295 = t619+t914;
t1297 = t738+t838;
t1345 = dq4.*t1116.*(4.0./5.0);
t1409 = -t1277;
t1433 = t655+t917;
t1434 = t741+t861;
t1462 = (t653-t838).^2;
t1527 = -t8.*(t653-t838);
t1531 = -t15.*(t653-t838);
t1581 = -dq6.*t7.*(t653-t838);
t1586 = -dq6.*t14.*(t653-t838);
t1604 = t15.*(t653-t838);
t1612 = -t1602;
t1618 = dq7.*t1596;
t1620 = dq7.*t1597;
t1623 = dq7.*t1599;
t1624 = dq7.*t1600;
t1625 = dq6.*t14.*(t653-t838);
t1631 = t7.*t1596;
t1632 = t7.*t1599;
t1637 = t709.*1.8866e-1;
t1642 = t22.*t1596;
t1646 = t22.*t1599;
t1651 = dq6.*t14.*t1596;
t1653 = -t1639;
t1655 = t792+t974;
t1656 = dq6.*t14.*t1599;
t1659 = dq7.*t1634;
t1662 = dq7.*t1635;
t1663 = -t1640;
t1668 = t7.*t1635;
t1669 = t690.*2.37e-3;
t1670 = t715.*2.37e-3;
t1671 = t670.*2.37e-3;
t1672 = t671.*2.37e-3;
t1673 = t749.*1.8866e-1;
t1677 = t715.*2.75e-2;
t1678 = t670.*2.75e-2;
t1679 = t671.*2.75e-2;
t1680 = t22.*t1635;
t1687 = dq6.*t14.*t1635;
t1688 = t690.*2.75e-2;
t1689 = t747.*2.37e-3;
t1690 = t752.*2.37e-3;
t1691 = -t1676;
t1692 = t709.*5.267999999999999e-2;
t1699 = -t1684;
t1700 = t836+t909;
t1702 = t699.*4.9e-4;
t1703 = t718.*4.9e-4;
t1706 = t712.*5.000000000000001e-5;
t1707 = t713.*5.000000000000001e-5;
t1709 = t672.*5.000000000000001e-5;
t1710 = t692.*2.019e-2;
t1712 = t747.*2.75e-2;
t1714 = t752.*2.75e-2;
t1716 = -t1698;
t1718 = t673.*2.019e-2;
t1721 = t695.*5.000000000000001e-5;
t1724 = t802.*2.37e-3;
t1725 = t805.*2.37e-3;
t1727 = -t1713;
t1728 = t749.*5.267999999999999e-2;
t1729 = t647+t1082;
t1733 = t668.*2.0e-4;
t1738 = t839+t966;
t1742 = t776.*4.9e-4;
t1749 = t629+t1130;
t1757 = t748.*5.000000000000001e-5;
t1759 = t751.*5.000000000000001e-5;
t1762 = t779.*2.019e-2;
t1764 = t802.*2.75e-2;
t1765 = -t1741;
t1767 = t805.*2.75e-2;
t1770 = t626+t1115;
t1773 = -t1754;
t1774 = -t1756;
t1775 = -t1758;
t1777 = t736+t1078;
t1781 = t746.*2.0e-4;
t1784 = t781+t1079;
t1785 = t716+t1136;
t1786 = -t1772;
t1790 = t804.*5.000000000000001e-5;
t1794 = t808.*5.000000000000001e-5;
t1796 = t711+t1126;
t1798 = t673.*1.9738e-1;
t1800 = t6.*t1748;
t1804 = t13.*t1748;
t1808 = t806.*3.466000000000001e-2;
t1812 = t692.*1.9738e-1;
t1816 = t811.*2.324e-2;
t1822 = -t1814;
t1823 = t111+t116+t124+t503+t889;
t1824 = dq7.*t1820;
t1825 = -t7.*(t637-t1126);
t1826 = dq7.*t1821;
t1828 = -t14.*(t637-t1126);
t1829 = -t8.*(t640-t1136);
t1830 = t163+t167+t299+t304+t902;
t1832 = -t15.*(t640-t1136);
t1838 = t779.*1.9738e-1;
t1842 = t827.*t1068;
t1843 = t827.*t1069;
t1846 = t827.*t1070;
t1850 = -t1837;
t1855 = t101+t291+t332+t334+t880;
t1859 = dq7.*t1849;
t1860 = t96+t292+t335+t337+t899;
t1861 = t15.*(t640-t1136);
t1865 = t127+t136+t345+t514+t891;
t1866 = t208+t833+t971;
t1910 = t992.*(-4.9e-4);
t1911 = t8.*t1863;
t1917 = t15.*t1863;
t1920 = t1019.*(-2.37e-3);
t1924 = t983.*(-2.019e-2);
t1925 = t1019.*(-2.75e-2);
t1932 = t992.*4.9e-4;
t1935 = t1019.*2.37e-3;
t1941 = t1019.*2.75e-2;
t1943 = t987.*(-3.466000000000001e-2);
t1950 = t7.*t1893;
t1953 = t14.*t1893;
t1962 = t995.*(-2.324e-2);
t1963 = t987.*3.466000000000001e-2;
t1971 = t995.*2.324e-2;
t1978 = t1010.*(-3.466000000000001e-2);
t1992 = -t1981;
t1994 = t983.*(-1.9738e-1);
t2001 = -t1989;
t2002 = -t1991;
t2006 = t983.*1.9738e-1;
t2012 = t1126.*1.8866e-1;
t2013 = t1127.*1.8866e-1;
t2025 = dq4.*t1116.*3.7732e-1;
t2029 = t1046.*(-2.324e-2);
t2036 = t834+t1600;
t2040 = t1117.*2.37e-3;
t2041 = t1118.*2.37e-3;
t2043 = t1131.*2.37e-3;
t2052 = t1161.*(-4.9e-4);
t2055 = -t2024;
t2062 = dq5.*t1120.*4.74e-3;
t2063 = dq5.*t1128.*4.74e-3;
t2065 = t1117.*2.75e-2;
t2066 = t1118.*2.75e-2;
t2068 = t1131.*2.75e-2;
t2072 = t1136.*2.75e-2;
t2075 = t837+t1634;
t2077 = dq5.*t1120.*5.5e-2;
t2079 = dq5.*t1128.*5.5e-2;
t2082 = -t2061;
t2084 = t1134.*4.9e-4;
t2087 = t1137.*4.9e-4;
t2091 = t1159.*(-2.019e-2);
t2092 = t1127.*5.267999999999999e-2;
t2094 = -t2069;
t2098 = dq6.*t1132.*9.8e-4;
t2101 = dq4.*t1116.*1.0536e-1;
t2104 = -t2056;
t2106 = t1123.*2.019e-2;
t2107 = t1132.*2.019e-2;
t2113 = t1120.*5.000000000000001e-5;
t2117 = t1128.*5.000000000000001e-5;
t2118 = t1129.*5.000000000000001e-5;
t2122 = dq5.*t1117.*1.0e-4;
t2123 = dq5.*t1131.*1.0e-4;
t2124 = t1116.*2.0e-4;
t2131 = dq6.*t1137.*4.038e-2;
t2137 = dq4.*t1127.*4.0e-4;
t2147 = t98+t333+t336+t709+t1049;
t2148 = t115+t125+t339+t668+t1073;
t2152 = t1159.*(-1.9738e-1);
t2156 = t5.*t2127;
t2157 = t6.*t2128;
t2159 = t12.*t2127;
t2160 = t13.*t2128;
t2163 = t110+t117+t343+t710+t1127;
t2170 = t7.*t2136;
t2171 = t1123.*1.9738e-1;
t2172 = t14.*t2136;
t2173 = t1132.*1.9738e-1;
t2177 = t158+t166+t305+t717+t1121;
t2178 = dq6.*t1137.*3.9476e-1;
t2185 = t7.*t2149;
t2188 = t14.*t2149;
t2190 = t2.*t10.*t2128;
t2196 = t181+t324+t325+t715+t1131;
t2201 = t10.*t11.*t2136;
t2230 = t6.*t2168;
t2235 = t13.*t2168;
t2244 = t6.*t2189;
t2247 = t13.*t2189;
t2249 = dq7.*t8.*(t653-t838).*(-3.466000000000001e-2);
t2275 = t9.*t10.*t2168;
t2303 = dq7.*t7.*t8.*(t653-t838).*(-2.324e-2);
t2305 = -t2271;
t2309 = t8.*t22.*(t653-t838).*(-2.324e-2);
t2316 = t2274.*(2.0./5.0);
t2320 = dq6.*t7.*(t653-t838).*(-1.9738e-1);
t2342 = -t2332;
t2344 = -t2335;
t2345 = t604.*t2127;
t2348 = -t2341;
t2353 = -t2349;
t2360 = t573.*t2189;
t2368 = -t2365;
t2384 = t611+t1210+t1223;
t2390 = -t2386;
t2391 = -t2388;
t2397 = -t2389;
t2400 = -t2393;
t2403 = -t2401;
t2407 = t827.*t2136;
t2411 = t1214.*7.000000000000001e-5;
t2413 = -t2128.*(t86-t652);
t2414 = t815.*t2168;
t2416 = t1210.*7.000000000000001e-5;
t2417 = -t2410;
t2419 = t1277.*7.000000000000001e-5;
t2422 = t1287.*7.000000000000001e-5;
t2425 = -t2415;
t2427 = -t2420;
t2428 = -t2421;
t2429 = -t2149.*(t92-t663);
t2431 = t2128.*(t86-t652);
t2434 = t1210.*4.999999999999997e-5;
t2435 = t1214.*4.999999999999997e-5;
t2436 = t1277.*4.999999999999997e-5;
t2437 = t1287.*4.999999999999997e-5;
t2438 = t1210.*2.23e-3;
t2439 = t1214.*2.23e-3;
t2448 = t1277.*2.23e-3;
t2449 = t1287.*2.23e-3;
t2453 = -t2450;
t2454 = t1217.*3.844e-2;
t2455 = t1218.*3.844e-2;
t2456 = t1225.*3.844e-2;
t2457 = -t2452;
t2458 = t1288.*3.844e-2;
t2459 = t1289.*3.844e-2;
t2461 = t1217.*1.12e-3;
t2462 = t1218.*1.12e-3;
t2463 = t1225.*1.12e-3;
t2465 = t1217.*8.8e-4;
t2466 = t1218.*8.8e-4;
t2467 = t1225.*8.8e-4;
t2469 = t1288.*8.8e-4;
t2470 = t1289.*8.8e-4;
t2474 = t1288.*1.12e-3;
t2475 = t1289.*1.12e-3;
t2479 = t1628.*7.000000000000022e-5;
t2484 = -t2478;
t2489 = t1628.*4.999999999999997e-5;
t2490 = t1665.*7.000000000000001e-5;
t2491 = t1665.*7.000000000000022e-5;
C = ft_4({dq1,dq2,dq3,dq4,dq5,dq6,dq7,t10,t1000,t1001,t1003,t1004,t1007,t1008,t1009,t1010,t1016,t1017,t1018,t1019,t1020,t1021,t1022,t1023,t1024,t1025,t1026,t1029,t1031,t1032,t1034,t1036,t1038,t1039,t1040,t1044,t1045,t1046,t105,t1050,t1052,t1053,t1055,t1056,t1057,t1058,t1066,t1067,t1069,t107,t1070,t1072,t1074,t1075,t1076,t1079,t1089,t109,t1094,t1096,t1097,t1098,t1099,t11,t1100,t1101,t1102,t1103,t1104,t1105,t1106,t1109,t1110,t1113,t1114,t1115,t1117,t1118,t1119,t112,t1120,t1123,t1125,t1126,t1128,t1130,t1132,t1133,t1135,t1136,t1137,t1138,t1139,t114,t1140,t1141,t1142,t1143,t1144,t1145,t1146,t1147,t1159,t1161,t1164,t1165,t1166,t1167,t1168,t1169,t1172,t1173,t1174,t1175,t1176,t1177,t1178,t1179,t1180,t1181,t1182,t1183,t1184,t1185,t1186,t1187,t1188,t1189,t119,t1190,t1191,t1193,t1194,t1195,t1197,t1198,t1199,t12,t1200,t1201,t1202,t1203,t1204,t1205,t1206,t1208,t1209,t1211,t1212,t1213,t1214,t1215,t1216,t1217,t1218,t1219,t122,t1220,t1221,t1222,t1224,t1225,t1226,t1227,t1228,t1229,t1231,t1232,t1237,t1238,t1239,t1249,t1250,t1253,t1256,t1257,t126,t1263,t1264,t1265,t1267,t1268,t1269,t1270,t1273,t1274,t1275,t1286,t1287,t1288,t1289,t1291,t1292,t1293,t1295,t1296,t1299,t13,t130,t1300,t1304,t1305,t1306,t1312,t1313,t1315,t1327,t1328,t1339,t1341,t1342,t1345,t1346,t1347,t1348,t1349,t1350,t1351,t1352,t1356,t1357,t1360,t1361,t1362,t1363,t1364,t1365,t1368,t1369,t137,t1376,t1377,t1380,t1381,t1382,t1384,t1385,t1388,t1389,t139,t1390,t1391,t14,t140,t1409,t1410,t1412,t1416,t1417,t1418,t1423,t1425,t1428,t1429,t1430,t1431,t1432,t1435,t1436,t144,t1441,t1449,t1450,t1451,t1453,t1455,t1456,t1462,t1467,t147,t1474,t1475,t1480,t149,t1490,t1491,t1492,t1495,t1496,t1497,t1498,t15,t1506,t1508,t1509,t151,t1510,t1511,t1512,t1513,t1517,t1518,t1519,t152,t1527,t1531,t1537,t1538,t1539,t1540,t1541,t1542,t1543,t1544,t1545,t1546,t1547,t1548,t1549,t1550,t1551,t1552,t1553,t1554,t1556,t156,t1561,t1562,t1563,t1565,t1566,t1567,t1568,t1569,t157,t1570,t1571,t1572,t1574,t1577,t1581,t1591,t1592,t1593,t1596,t16,t160,t1603,t1604,t1605,t1612,t1616,t1618,t162,t1622,t1623,t1624,t1625,t1627,t1628,t1629,t1630,t1631,t1634,t1635,t1636,t1637,t1638,t1642,t1643,t1644,t1648,t165,t1651,t1653,t1655,t1659,t1661,t1662,t1663,t1664,t1665,t1666,t1667,t1668,t1669,t1670,t1671,t1672,t1673,t1674,t1675,t1677,t1678,t1679,t168,t1680,t1683,t1687,t1688,t1689,t1690,t1691,t1692,t1694,t1696,t1699,t17,t1700,t1701,t1702,t1703,t1704,t1706,t1707,t1708,t1709,t171,t1710,t1712,t1714,t1715,t1716,t1717,t1718,t1721,t1723,t1724,t1725,t1727,t1728,t1729,t1733,t1734,t1735,t1736,t1738,t1739,t1740,t1742,t1744,t1747,t1748,t1749,t175,t1751,t1757,t1759,t1760,t1762,t1764,t1765,t1767,t1768,t1770,t1772,t1773,t1774,t1775,t1781,t1786,t1788,t1789,t1790,t1791,t1794,t1798,t180,t1800,t1804,t1807,t1808,t1812,t1814,t1816,t1819,t182,t1820,t1822,t1823,t1824,t1825,t1826,t1827,t1828,t1829,t1830,t1831,t1834,t1836,t1837,t1838,t1840,t1842,t1843,t1846,t1849,t185,t1850,t1852,t1855,t1859,t186,t1860,t1861,t1863,t1865,t1866,t187,t1877,t1879,t1881,t1885,t1887,t189,t1892,t1893,t1895,t1896,t1897,t1898,t1900,t1901,t1904,t1905,t1908,t1911,t1916,t1917,t1924,t1926,t1928,t1932,t1934,t1935,t1937,t1941,t1944,t1945,t1946,t1947,t1949,t1950,t1951,t1952,t1953,t1955,t1960,t1962,t1963,t1965,t1966,t1967,t1968,t1971,t1973,t1977,t1978,t1980,t1982,t1983,t1990,t1992,t1998,t1999,t2,t2001,t2002,t2003,t2004,t2006,t2008,t2009,t2010,t2011,t2012,t2013,t2014,t2015,t2016,t2018,t2020,t2023,t2024,t2025,t2026,t2027,t2028,t2029,t2030,t2031,t2032,t2034,t2036,t2038,t2040,t2041,t2042,t2043,t2049,t2050,t2055,t2056,t2059,t2060,t2062,t2063,t2065,t2066,t2068,t2072,t2075,t2077,t2078,t2079,t208,t2082,t2084,t2087,t2092,t2094,t2098,t2099,t21,t2101,t2104,t2106,t2107,t2113,t2117,t2118,t2121,t2122,t2123,t2124,t2129,t2131,t2135,t2137,t2143,t2147,t2148,t2149,t2150,t2152,t2153,t2155,t2156,t2157,t2158,t2159,t2160,t2162,t2163,t2166,t2167,t2169,t2170,t2171,t2172,t2173,t2174,t2175,t2177,t2178,t2185,t2188,t2190,t2194,t2196,t22,t2201,t221,t223,t2230,t2235,t2244,t2247,t2249,t2252,t2271,t2272,t2274,t2275,t2284,t2285,t2293,t2296,t2298,t23,t230,t2305,t2309,t231,t2316,t2317,t2318,t232,t233,t2331,t2333,t2336,t2337,t234,t2341,t2342,t2344,t2345,t2347,t2348,t235,t2353,t236,t2360,t2361,t2364,t2365,t2368,t237,t2373,t238,t2381,t2384,t2387,t2388,t239,t2390,t2391,t2393,t2396,t2397,t24,t240,t2400,t2402,t2403,t2404,t2405,t2406,t2407,t2408,t2409,t241,t2411,t2414,t2416,t2417,t2419,t242,t2422,t2423,t2425,t2427,t2428,t2429,t243,t2431,t2432,t2433,t2434,t2435,t2436,t2437,t2438,t2439,t244,t2440,t2448,t2449,t2453,t2454,t2455,t2456,t2457,t2458,t2459,t2461,t2462,t2463,t2465,t2466,t2467,t2468,t2469,t2470,t2472,t2474,t2475,t2479,t248,t2480,t2484,t2489,t2490,t2491,t2493,t2494,t25,t250,t251,t252,t253,t2534,t254,t258,t259,t26,t2622,t267,t2678,t268,t269,t2696,t27,t270,t271,t272,t273,t2730,t274,t275,t276,t277,t279,t28,t280,t281,t282,t283,t284,t285,t286,t287,t288,t289,t29,t290,t293,t294,t295,t296,t297,t298,t3,t30,t301,t307,t308,t309,t31,t310,t311,t312,t313,t314,t315,t316,t317,t318,t319,t32,t320,t322,t3248,t3249,t3252,t327,t328,t329,t33,t330,t331,t338,t34,t341,t342,t346,t347,t348,t349,t35,t358,t36,t361,t364,t3672,t3673,t3679,t368,t37,t373,t378,t386,t387,t389,t39,t390,t393,t394,t395,t397,t399,t4,t40,t402,t406,t407,t408,t411,t412,t415,t416,t417,t418,t419,t420,t427,t428,t429,t43,t431,t432,t433,t434,t435,t436,t438,t439,t441,t442,t443,t444,t446,t448,t45,t450,t451,t452,t453,t455,t456,t457,t458,t459,t46,t460,t461,t463,t464,t465,t466,t467,t468,t469,t470,t472,t473,t476,t477,t478,t479,t480,t481,t483,t484,t489,t49,t494,t495,t496,t5,t50,t501,t502,t504,t505,t506,t507,t508,t509,t51,t510,t511,t512,t515,t516,t517,t518,t519,t522,t523,t524,t525,t526,t527,t528,t529,t530,t531,t533,t534,t535,t536,t537,t538,t542,t543,t544,t545,t546,t547,t548,t549,t55,t550,t551,t552,t553,t554,t556,t557,t558,t561,t562,t563,t564,t565,t566,t567,t568,t569,t57,t570,t571,t572,t573,t574,t575,t576,t577,t578,t579,t58,t580,t581,t582,t583,t584,t585,t586,t587,t588,t589,t590,t591,t592,t593,t594,t595,t596,t597,t598,t599,t6,t600,t601,t602,t603,t604,t605,t606,t607,t608,t609,t61,t612,t613,t614,t615,t616,t617,t618,t619,t620,t621,t622,t623,t624,t626,t627,t628,t629,t63,t631,t632,t633,t634,t635,t637,t638,t639,t64,t640,t642,t643,t644,t646,t647,t648,t649,t650,t651,t652,t653,t654,t656,t657,t658,t660,t661,t662,t663,t664,t665,t666,t667,t669,t67,t670,t671,t673,t674,t675,t676,t677,t678,t679,t680,t681,t683,t684,t685,t686,t687,t688,t689,t69,t691,t692,t693,t694,t695,t696,t697,t698,t699,t7,t70,t700,t701,t702,t703,t704,t705,t706,t707,t708,t71,t712,t713,t714,t719,t72,t720,t721,t722,t723,t724,t725,t726,t728,t729,t73,t730,t731,t734,t735,t737,t74,t740,t743,t744,t745,t748,t749,t75,t750,t751,t753,t754,t755,t756,t757,t758,t759,t76,t760,t761,t762,t763,t764,t765,t766,t769,t77,t770,t771,t772,t773,t774,t775,t776,t777,t778,t779,t78,t780,t782,t783,t784,t785,t786,t787,t788,t79,t790,t791,t792,t794,t795,t796,t798,t799,t8,t80,t800,t801,t802,t803,t805,t806,t809,t81,t810,t811,t812,t813,t815,t816,t817,t818,t819,t82,t820,t821,t822,t827,t83,t831,t834,t835,t836,t837,t838,t839,t84,t840,t841,t842,t843,t845,t846,t847,t848,t849,t85,t850,t851,t852,t853,t854,t855,t856,t857,t859,t86,t860,t862,t863,t864,t866,t867,t868,t869,t87,t870,t871,t872,t873,t876,t877,t88,t880,t881,t882,t883,t886,t888,t889,t89,t890,t891,t892,t894,t898,t899,t9,t90,t900,t901,t902,t903,t904,t905,t908,t91,t911,t913,t915,t916,t918,t919,t92,t920,t922,t924,t925,t931,t934,t936,t937,t938,t94,t940,t941,t942,t944,t945,t946,t947,t948,t950,t952,t953,t954,t955,t958,t959,t965,t966,t968,t969,t97,t972,t973,t974,t975,t977,t978,t979,t982,t983,t987,t992,t994,t995,t997,t999});
end
function C = ft_4(ct)
dq1 = ct{1};
dq2 = ct{2};
dq3 = ct{3};
dq4 = ct{4};
dq5 = ct{5};
dq6 = ct{6};
dq7 = ct{7};
t10 = ct{8};
t1000 = ct{9};
t1001 = ct{10};
t1003 = ct{11};
t1004 = ct{12};
t1007 = ct{13};
t1008 = ct{14};
t1009 = ct{15};
t1010 = ct{16};
t1016 = ct{17};
t1017 = ct{18};
t1018 = ct{19};
t1019 = ct{20};
t1020 = ct{21};
t1021 = ct{22};
t1022 = ct{23};
t1023 = ct{24};
t1024 = ct{25};
t1025 = ct{26};
t1026 = ct{27};
t1029 = ct{28};
t1031 = ct{29};
t1032 = ct{30};
t1034 = ct{31};
t1036 = ct{32};
t1038 = ct{33};
t1039 = ct{34};
t1040 = ct{35};
t1044 = ct{36};
t1045 = ct{37};
t1046 = ct{38};
t105 = ct{39};
t1050 = ct{40};
t1052 = ct{41};
t1053 = ct{42};
t1055 = ct{43};
t1056 = ct{44};
t1057 = ct{45};
t1058 = ct{46};
t1066 = ct{47};
t1067 = ct{48};
t1069 = ct{49};
t107 = ct{50};
t1070 = ct{51};
t1072 = ct{52};
t1074 = ct{53};
t1075 = ct{54};
t1076 = ct{55};
t1079 = ct{56};
t1089 = ct{57};
t109 = ct{58};
t1094 = ct{59};
t1096 = ct{60};
t1097 = ct{61};
t1098 = ct{62};
t1099 = ct{63};
t11 = ct{64};
t1100 = ct{65};
t1101 = ct{66};
t1102 = ct{67};
t1103 = ct{68};
t1104 = ct{69};
t1105 = ct{70};
t1106 = ct{71};
t1109 = ct{72};
t1110 = ct{73};
t1113 = ct{74};
t1114 = ct{75};
t1115 = ct{76};
t1117 = ct{77};
t1118 = ct{78};
t1119 = ct{79};
t112 = ct{80};
t1120 = ct{81};
t1123 = ct{82};
t1125 = ct{83};
t1126 = ct{84};
t1128 = ct{85};
t1130 = ct{86};
t1132 = ct{87};
t1133 = ct{88};
t1135 = ct{89};
t1136 = ct{90};
t1137 = ct{91};
t1138 = ct{92};
t1139 = ct{93};
t114 = ct{94};
t1140 = ct{95};
t1141 = ct{96};
t1142 = ct{97};
t1143 = ct{98};
t1144 = ct{99};
t1145 = ct{100};
t1146 = ct{101};
t1147 = ct{102};
t1159 = ct{103};
t1161 = ct{104};
t1164 = ct{105};
t1165 = ct{106};
t1166 = ct{107};
t1167 = ct{108};
t1168 = ct{109};
t1169 = ct{110};
t1172 = ct{111};
t1173 = ct{112};
t1174 = ct{113};
t1175 = ct{114};
t1176 = ct{115};
t1177 = ct{116};
t1178 = ct{117};
t1179 = ct{118};
t1180 = ct{119};
t1181 = ct{120};
t1182 = ct{121};
t1183 = ct{122};
t1184 = ct{123};
t1185 = ct{124};
t1186 = ct{125};
t1187 = ct{126};
t1188 = ct{127};
t1189 = ct{128};
t119 = ct{129};
t1190 = ct{130};
t1191 = ct{131};
t1193 = ct{132};
t1194 = ct{133};
t1195 = ct{134};
t1197 = ct{135};
t1198 = ct{136};
t1199 = ct{137};
t12 = ct{138};
t1200 = ct{139};
t1201 = ct{140};
t1202 = ct{141};
t1203 = ct{142};
t1204 = ct{143};
t1205 = ct{144};
t1206 = ct{145};
t1208 = ct{146};
t1209 = ct{147};
t1211 = ct{148};
t1212 = ct{149};
t1213 = ct{150};
t1214 = ct{151};
t1215 = ct{152};
t1216 = ct{153};
t1217 = ct{154};
t1218 = ct{155};
t1219 = ct{156};
t122 = ct{157};
t1220 = ct{158};
t1221 = ct{159};
t1222 = ct{160};
t1224 = ct{161};
t1225 = ct{162};
t1226 = ct{163};
t1227 = ct{164};
t1228 = ct{165};
t1229 = ct{166};
t1231 = ct{167};
t1232 = ct{168};
t1237 = ct{169};
t1238 = ct{170};
t1239 = ct{171};
t1249 = ct{172};
t1250 = ct{173};
t1253 = ct{174};
t1256 = ct{175};
t1257 = ct{176};
t126 = ct{177};
t1263 = ct{178};
t1264 = ct{179};
t1265 = ct{180};
t1267 = ct{181};
t1268 = ct{182};
t1269 = ct{183};
t1270 = ct{184};
t1273 = ct{185};
t1274 = ct{186};
t1275 = ct{187};
t1286 = ct{188};
t1287 = ct{189};
t1288 = ct{190};
t1289 = ct{191};
t1291 = ct{192};
t1292 = ct{193};
t1293 = ct{194};
t1295 = ct{195};
t1296 = ct{196};
t1299 = ct{197};
t13 = ct{198};
t130 = ct{199};
t1300 = ct{200};
t1304 = ct{201};
t1305 = ct{202};
t1306 = ct{203};
t1312 = ct{204};
t1313 = ct{205};
t1315 = ct{206};
t1327 = ct{207};
t1328 = ct{208};
t1339 = ct{209};
t1341 = ct{210};
t1342 = ct{211};
t1345 = ct{212};
t1346 = ct{213};
t1347 = ct{214};
t1348 = ct{215};
t1349 = ct{216};
t1350 = ct{217};
t1351 = ct{218};
t1352 = ct{219};
t1356 = ct{220};
t1357 = ct{221};
t1360 = ct{222};
t1361 = ct{223};
t1362 = ct{224};
t1363 = ct{225};
t1364 = ct{226};
t1365 = ct{227};
t1368 = ct{228};
t1369 = ct{229};
t137 = ct{230};
t1376 = ct{231};
t1377 = ct{232};
t1380 = ct{233};
t1381 = ct{234};
t1382 = ct{235};
t1384 = ct{236};
t1385 = ct{237};
t1388 = ct{238};
t1389 = ct{239};
t139 = ct{240};
t1390 = ct{241};
t1391 = ct{242};
t14 = ct{243};
t140 = ct{244};
t1409 = ct{245};
t1410 = ct{246};
t1412 = ct{247};
t1416 = ct{248};
t1417 = ct{249};
t1418 = ct{250};
t1423 = ct{251};
t1425 = ct{252};
t1428 = ct{253};
t1429 = ct{254};
t1430 = ct{255};
t1431 = ct{256};
t1432 = ct{257};
t1435 = ct{258};
t1436 = ct{259};
t144 = ct{260};
t1441 = ct{261};
t1449 = ct{262};
t1450 = ct{263};
t1451 = ct{264};
t1453 = ct{265};
t1455 = ct{266};
t1456 = ct{267};
t1462 = ct{268};
t1467 = ct{269};
t147 = ct{270};
t1474 = ct{271};
t1475 = ct{272};
t1480 = ct{273};
t149 = ct{274};
t1490 = ct{275};
t1491 = ct{276};
t1492 = ct{277};
t1495 = ct{278};
t1496 = ct{279};
t1497 = ct{280};
t1498 = ct{281};
t15 = ct{282};
t1506 = ct{283};
t1508 = ct{284};
t1509 = ct{285};
t151 = ct{286};
t1510 = ct{287};
t1511 = ct{288};
t1512 = ct{289};
t1513 = ct{290};
t1517 = ct{291};
t1518 = ct{292};
t1519 = ct{293};
t152 = ct{294};
t1527 = ct{295};
t1531 = ct{296};
t1537 = ct{297};
t1538 = ct{298};
t1539 = ct{299};
t1540 = ct{300};
t1541 = ct{301};
t1542 = ct{302};
t1543 = ct{303};
t1544 = ct{304};
t1545 = ct{305};
t1546 = ct{306};
t1547 = ct{307};
t1548 = ct{308};
t1549 = ct{309};
t1550 = ct{310};
t1551 = ct{311};
t1552 = ct{312};
t1553 = ct{313};
t1554 = ct{314};
t1556 = ct{315};
t156 = ct{316};
t1561 = ct{317};
t1562 = ct{318};
t1563 = ct{319};
t1565 = ct{320};
t1566 = ct{321};
t1567 = ct{322};
t1568 = ct{323};
t1569 = ct{324};
t157 = ct{325};
t1570 = ct{326};
t1571 = ct{327};
t1572 = ct{328};
t1574 = ct{329};
t1577 = ct{330};
t1581 = ct{331};
t1591 = ct{332};
t1592 = ct{333};
t1593 = ct{334};
t1596 = ct{335};
t16 = ct{336};
t160 = ct{337};
t1603 = ct{338};
t1604 = ct{339};
t1605 = ct{340};
t1612 = ct{341};
t1616 = ct{342};
t1618 = ct{343};
t162 = ct{344};
t1622 = ct{345};
t1623 = ct{346};
t1624 = ct{347};
t1625 = ct{348};
t1627 = ct{349};
t1628 = ct{350};
t1629 = ct{351};
t1630 = ct{352};
t1631 = ct{353};
t1634 = ct{354};
t1635 = ct{355};
t1636 = ct{356};
t1637 = ct{357};
t1638 = ct{358};
t1642 = ct{359};
t1643 = ct{360};
t1644 = ct{361};
t1648 = ct{362};
t165 = ct{363};
t1651 = ct{364};
t1653 = ct{365};
t1655 = ct{366};
t1659 = ct{367};
t1661 = ct{368};
t1662 = ct{369};
t1663 = ct{370};
t1664 = ct{371};
t1665 = ct{372};
t1666 = ct{373};
t1667 = ct{374};
t1668 = ct{375};
t1669 = ct{376};
t1670 = ct{377};
t1671 = ct{378};
t1672 = ct{379};
t1673 = ct{380};
t1674 = ct{381};
t1675 = ct{382};
t1677 = ct{383};
t1678 = ct{384};
t1679 = ct{385};
t168 = ct{386};
t1680 = ct{387};
t1683 = ct{388};
t1687 = ct{389};
t1688 = ct{390};
t1689 = ct{391};
t1690 = ct{392};
t1691 = ct{393};
t1692 = ct{394};
t1694 = ct{395};
t1696 = ct{396};
t1699 = ct{397};
t17 = ct{398};
t1700 = ct{399};
t1701 = ct{400};
t1702 = ct{401};
t1703 = ct{402};
t1704 = ct{403};
t1706 = ct{404};
t1707 = ct{405};
t1708 = ct{406};
t1709 = ct{407};
t171 = ct{408};
t1710 = ct{409};
t1712 = ct{410};
t1714 = ct{411};
t1715 = ct{412};
t1716 = ct{413};
t1717 = ct{414};
t1718 = ct{415};
t1721 = ct{416};
t1723 = ct{417};
t1724 = ct{418};
t1725 = ct{419};
t1727 = ct{420};
t1728 = ct{421};
t1729 = ct{422};
t1733 = ct{423};
t1734 = ct{424};
t1735 = ct{425};
t1736 = ct{426};
t1738 = ct{427};
t1739 = ct{428};
t1740 = ct{429};
t1742 = ct{430};
t1744 = ct{431};
t1747 = ct{432};
t1748 = ct{433};
t1749 = ct{434};
t175 = ct{435};
t1751 = ct{436};
t1757 = ct{437};
t1759 = ct{438};
t1760 = ct{439};
t1762 = ct{440};
t1764 = ct{441};
t1765 = ct{442};
t1767 = ct{443};
t1768 = ct{444};
t1770 = ct{445};
t1772 = ct{446};
t1773 = ct{447};
t1774 = ct{448};
t1775 = ct{449};
t1781 = ct{450};
t1786 = ct{451};
t1788 = ct{452};
t1789 = ct{453};
t1790 = ct{454};
t1791 = ct{455};
t1794 = ct{456};
t1798 = ct{457};
t180 = ct{458};
t1800 = ct{459};
t1804 = ct{460};
t1807 = ct{461};
t1808 = ct{462};
t1812 = ct{463};
t1814 = ct{464};
t1816 = ct{465};
t1819 = ct{466};
t182 = ct{467};
t1820 = ct{468};
t1822 = ct{469};
t1823 = ct{470};
t1824 = ct{471};
t1825 = ct{472};
t1826 = ct{473};
t1827 = ct{474};
t1828 = ct{475};
t1829 = ct{476};
t1830 = ct{477};
t1831 = ct{478};
t1834 = ct{479};
t1836 = ct{480};
t1837 = ct{481};
t1838 = ct{482};
t1840 = ct{483};
t1842 = ct{484};
t1843 = ct{485};
t1846 = ct{486};
t1849 = ct{487};
t185 = ct{488};
t1850 = ct{489};
t1852 = ct{490};
t1855 = ct{491};
t1859 = ct{492};
t186 = ct{493};
t1860 = ct{494};
t1861 = ct{495};
t1863 = ct{496};
t1865 = ct{497};
t1866 = ct{498};
t187 = ct{499};
t1877 = ct{500};
t1879 = ct{501};
t1881 = ct{502};
t1885 = ct{503};
t1887 = ct{504};
t189 = ct{505};
t1892 = ct{506};
t1893 = ct{507};
t1895 = ct{508};
t1896 = ct{509};
t1897 = ct{510};
t1898 = ct{511};
t1900 = ct{512};
t1901 = ct{513};
t1904 = ct{514};
t1905 = ct{515};
t1908 = ct{516};
t1911 = ct{517};
t1916 = ct{518};
t1917 = ct{519};
t1924 = ct{520};
t1926 = ct{521};
t1928 = ct{522};
t1932 = ct{523};
t1934 = ct{524};
t1935 = ct{525};
t1937 = ct{526};
t1941 = ct{527};
t1944 = ct{528};
t1945 = ct{529};
t1946 = ct{530};
t1947 = ct{531};
t1949 = ct{532};
t1950 = ct{533};
t1951 = ct{534};
t1952 = ct{535};
t1953 = ct{536};
t1955 = ct{537};
t1960 = ct{538};
t1962 = ct{539};
t1963 = ct{540};
t1965 = ct{541};
t1966 = ct{542};
t1967 = ct{543};
t1968 = ct{544};
t1971 = ct{545};
t1973 = ct{546};
t1977 = ct{547};
t1978 = ct{548};
t1980 = ct{549};
t1982 = ct{550};
t1983 = ct{551};
t1990 = ct{552};
t1992 = ct{553};
t1998 = ct{554};
t1999 = ct{555};
t2 = ct{556};
t2001 = ct{557};
t2002 = ct{558};
t2003 = ct{559};
t2004 = ct{560};
t2006 = ct{561};
t2008 = ct{562};
t2009 = ct{563};
t2010 = ct{564};
t2011 = ct{565};
t2012 = ct{566};
t2013 = ct{567};
t2014 = ct{568};
t2015 = ct{569};
t2016 = ct{570};
t2018 = ct{571};
t2020 = ct{572};
t2023 = ct{573};
t2024 = ct{574};
t2025 = ct{575};
t2026 = ct{576};
t2027 = ct{577};
t2028 = ct{578};
t2029 = ct{579};
t2030 = ct{580};
t2031 = ct{581};
t2032 = ct{582};
t2034 = ct{583};
t2036 = ct{584};
t2038 = ct{585};
t2040 = ct{586};
t2041 = ct{587};
t2042 = ct{588};
t2043 = ct{589};
t2049 = ct{590};
t2050 = ct{591};
t2055 = ct{592};
t2056 = ct{593};
t2059 = ct{594};
t2060 = ct{595};
t2062 = ct{596};
t2063 = ct{597};
t2065 = ct{598};
t2066 = ct{599};
t2068 = ct{600};
t2072 = ct{601};
t2075 = ct{602};
t2077 = ct{603};
t2078 = ct{604};
t2079 = ct{605};
t208 = ct{606};
t2082 = ct{607};
t2084 = ct{608};
t2087 = ct{609};
t2092 = ct{610};
t2094 = ct{611};
t2098 = ct{612};
t2099 = ct{613};
t21 = ct{614};
t2101 = ct{615};
t2104 = ct{616};
t2106 = ct{617};
t2107 = ct{618};
t2113 = ct{619};
t2117 = ct{620};
t2118 = ct{621};
t2121 = ct{622};
t2122 = ct{623};
t2123 = ct{624};
t2124 = ct{625};
t2129 = ct{626};
t2131 = ct{627};
t2135 = ct{628};
t2137 = ct{629};
t2143 = ct{630};
t2147 = ct{631};
t2148 = ct{632};
t2149 = ct{633};
t2150 = ct{634};
t2152 = ct{635};
t2153 = ct{636};
t2155 = ct{637};
t2156 = ct{638};
t2157 = ct{639};
t2158 = ct{640};
t2159 = ct{641};
t2160 = ct{642};
t2162 = ct{643};
t2163 = ct{644};
t2166 = ct{645};
t2167 = ct{646};
t2169 = ct{647};
t2170 = ct{648};
t2171 = ct{649};
t2172 = ct{650};
t2173 = ct{651};
t2174 = ct{652};
t2175 = ct{653};
t2177 = ct{654};
t2178 = ct{655};
t2185 = ct{656};
t2188 = ct{657};
t2190 = ct{658};
t2194 = ct{659};
t2196 = ct{660};
t22 = ct{661};
t2201 = ct{662};
t221 = ct{663};
t223 = ct{664};
t2230 = ct{665};
t2235 = ct{666};
t2244 = ct{667};
t2247 = ct{668};
t2249 = ct{669};
t2252 = ct{670};
t2271 = ct{671};
t2272 = ct{672};
t2274 = ct{673};
t2275 = ct{674};
t2284 = ct{675};
t2285 = ct{676};
t2293 = ct{677};
t2296 = ct{678};
t2298 = ct{679};
t23 = ct{680};
t230 = ct{681};
t2305 = ct{682};
t2309 = ct{683};
t231 = ct{684};
t2316 = ct{685};
t2317 = ct{686};
t2318 = ct{687};
t232 = ct{688};
t233 = ct{689};
t2331 = ct{690};
t2333 = ct{691};
t2336 = ct{692};
t2337 = ct{693};
t234 = ct{694};
t2341 = ct{695};
t2342 = ct{696};
t2344 = ct{697};
t2345 = ct{698};
t2347 = ct{699};
t2348 = ct{700};
t235 = ct{701};
t2353 = ct{702};
t236 = ct{703};
t2360 = ct{704};
t2361 = ct{705};
t2364 = ct{706};
t2365 = ct{707};
t2368 = ct{708};
t237 = ct{709};
t2373 = ct{710};
t238 = ct{711};
t2381 = ct{712};
t2384 = ct{713};
t2387 = ct{714};
t2388 = ct{715};
t239 = ct{716};
t2390 = ct{717};
t2391 = ct{718};
t2393 = ct{719};
t2396 = ct{720};
t2397 = ct{721};
t24 = ct{722};
t240 = ct{723};
t2400 = ct{724};
t2402 = ct{725};
t2403 = ct{726};
t2404 = ct{727};
t2405 = ct{728};
t2406 = ct{729};
t2407 = ct{730};
t2408 = ct{731};
t2409 = ct{732};
t241 = ct{733};
t2411 = ct{734};
t2414 = ct{735};
t2416 = ct{736};
t2417 = ct{737};
t2419 = ct{738};
t242 = ct{739};
t2422 = ct{740};
t2423 = ct{741};
t2425 = ct{742};
t2427 = ct{743};
t2428 = ct{744};
t2429 = ct{745};
t243 = ct{746};
t2431 = ct{747};
t2432 = ct{748};
t2433 = ct{749};
t2434 = ct{750};
t2435 = ct{751};
t2436 = ct{752};
t2437 = ct{753};
t2438 = ct{754};
t2439 = ct{755};
t244 = ct{756};
t2440 = ct{757};
t2448 = ct{758};
t2449 = ct{759};
t2453 = ct{760};
t2454 = ct{761};
t2455 = ct{762};
t2456 = ct{763};
t2457 = ct{764};
t2458 = ct{765};
t2459 = ct{766};
t2461 = ct{767};
t2462 = ct{768};
t2463 = ct{769};
t2465 = ct{770};
t2466 = ct{771};
t2467 = ct{772};
t2468 = ct{773};
t2469 = ct{774};
t2470 = ct{775};
t2472 = ct{776};
t2474 = ct{777};
t2475 = ct{778};
t2479 = ct{779};
t248 = ct{780};
t2480 = ct{781};
t2484 = ct{782};
t2489 = ct{783};
t2490 = ct{784};
t2491 = ct{785};
t2493 = ct{786};
t2494 = ct{787};
t25 = ct{788};
t250 = ct{789};
t251 = ct{790};
t252 = ct{791};
t253 = ct{792};
t2534 = ct{793};
t254 = ct{794};
t258 = ct{795};
t259 = ct{796};
t26 = ct{797};
t2622 = ct{798};
t267 = ct{799};
t2678 = ct{800};
t268 = ct{801};
t269 = ct{802};
t2696 = ct{803};
t27 = ct{804};
t270 = ct{805};
t271 = ct{806};
t272 = ct{807};
t273 = ct{808};
t2730 = ct{809};
t274 = ct{810};
t275 = ct{811};
t276 = ct{812};
t277 = ct{813};
t279 = ct{814};
t28 = ct{815};
t280 = ct{816};
t281 = ct{817};
t282 = ct{818};
t283 = ct{819};
t284 = ct{820};
t285 = ct{821};
t286 = ct{822};
t287 = ct{823};
t288 = ct{824};
t289 = ct{825};
t29 = ct{826};
t290 = ct{827};
t293 = ct{828};
t294 = ct{829};
t295 = ct{830};
t296 = ct{831};
t297 = ct{832};
t298 = ct{833};
t3 = ct{834};
t30 = ct{835};
t301 = ct{836};
t307 = ct{837};
t308 = ct{838};
t309 = ct{839};
t31 = ct{840};
t310 = ct{841};
t311 = ct{842};
t312 = ct{843};
t313 = ct{844};
t314 = ct{845};
t315 = ct{846};
t316 = ct{847};
t317 = ct{848};
t318 = ct{849};
t319 = ct{850};
t32 = ct{851};
t320 = ct{852};
t322 = ct{853};
t3248 = ct{854};
t3249 = ct{855};
t3252 = ct{856};
t327 = ct{857};
t328 = ct{858};
t329 = ct{859};
t33 = ct{860};
t330 = ct{861};
t331 = ct{862};
t338 = ct{863};
t34 = ct{864};
t341 = ct{865};
t342 = ct{866};
t346 = ct{867};
t347 = ct{868};
t348 = ct{869};
t349 = ct{870};
t35 = ct{871};
t358 = ct{872};
t36 = ct{873};
t361 = ct{874};
t364 = ct{875};
t3672 = ct{876};
t3673 = ct{877};
t3679 = ct{878};
t368 = ct{879};
t37 = ct{880};
t373 = ct{881};
t378 = ct{882};
t386 = ct{883};
t387 = ct{884};
t389 = ct{885};
t39 = ct{886};
t390 = ct{887};
t393 = ct{888};
t394 = ct{889};
t395 = ct{890};
t397 = ct{891};
t399 = ct{892};
t4 = ct{893};
t40 = ct{894};
t402 = ct{895};
t406 = ct{896};
t407 = ct{897};
t408 = ct{898};
t411 = ct{899};
t412 = ct{900};
t415 = ct{901};
t416 = ct{902};
t417 = ct{903};
t418 = ct{904};
t419 = ct{905};
t420 = ct{906};
t427 = ct{907};
t428 = ct{908};
t429 = ct{909};
t43 = ct{910};
t431 = ct{911};
t432 = ct{912};
t433 = ct{913};
t434 = ct{914};
t435 = ct{915};
t436 = ct{916};
t438 = ct{917};
t439 = ct{918};
t441 = ct{919};
t442 = ct{920};
t443 = ct{921};
t444 = ct{922};
t446 = ct{923};
t448 = ct{924};
t45 = ct{925};
t450 = ct{926};
t451 = ct{927};
t452 = ct{928};
t453 = ct{929};
t455 = ct{930};
t456 = ct{931};
t457 = ct{932};
t458 = ct{933};
t459 = ct{934};
t46 = ct{935};
t460 = ct{936};
t461 = ct{937};
t463 = ct{938};
t464 = ct{939};
t465 = ct{940};
t466 = ct{941};
t467 = ct{942};
t468 = ct{943};
t469 = ct{944};
t470 = ct{945};
t472 = ct{946};
t473 = ct{947};
t476 = ct{948};
t477 = ct{949};
t478 = ct{950};
t479 = ct{951};
t480 = ct{952};
t481 = ct{953};
t483 = ct{954};
t484 = ct{955};
t489 = ct{956};
t49 = ct{957};
t494 = ct{958};
t495 = ct{959};
t496 = ct{960};
t5 = ct{961};
t50 = ct{962};
t501 = ct{963};
t502 = ct{964};
t504 = ct{965};
t505 = ct{966};
t506 = ct{967};
t507 = ct{968};
t508 = ct{969};
t509 = ct{970};
t51 = ct{971};
t510 = ct{972};
t511 = ct{973};
t512 = ct{974};
t515 = ct{975};
t516 = ct{976};
t517 = ct{977};
t518 = ct{978};
t519 = ct{979};
t522 = ct{980};
t523 = ct{981};
t524 = ct{982};
t525 = ct{983};
t526 = ct{984};
t527 = ct{985};
t528 = ct{986};
t529 = ct{987};
t530 = ct{988};
t531 = ct{989};
t533 = ct{990};
t534 = ct{991};
t535 = ct{992};
t536 = ct{993};
t537 = ct{994};
t538 = ct{995};
t542 = ct{996};
t543 = ct{997};
t544 = ct{998};
t545 = ct{999};
t546 = ct{1000};
t547 = ct{1001};
t548 = ct{1002};
t549 = ct{1003};
t55 = ct{1004};
t550 = ct{1005};
t551 = ct{1006};
t552 = ct{1007};
t553 = ct{1008};
t554 = ct{1009};
t556 = ct{1010};
t557 = ct{1011};
t558 = ct{1012};
t561 = ct{1013};
t562 = ct{1014};
t563 = ct{1015};
t564 = ct{1016};
t565 = ct{1017};
t566 = ct{1018};
t567 = ct{1019};
t568 = ct{1020};
t569 = ct{1021};
t57 = ct{1022};
t570 = ct{1023};
t571 = ct{1024};
t572 = ct{1025};
t573 = ct{1026};
t574 = ct{1027};
t575 = ct{1028};
t576 = ct{1029};
t577 = ct{1030};
t578 = ct{1031};
t579 = ct{1032};
t58 = ct{1033};
t580 = ct{1034};
t581 = ct{1035};
t582 = ct{1036};
t583 = ct{1037};
t584 = ct{1038};
t585 = ct{1039};
t586 = ct{1040};
t587 = ct{1041};
t588 = ct{1042};
t589 = ct{1043};
t590 = ct{1044};
t591 = ct{1045};
t592 = ct{1046};
t593 = ct{1047};
t594 = ct{1048};
t595 = ct{1049};
t596 = ct{1050};
t597 = ct{1051};
t598 = ct{1052};
t599 = ct{1053};
t6 = ct{1054};
t600 = ct{1055};
t601 = ct{1056};
t602 = ct{1057};
t603 = ct{1058};
t604 = ct{1059};
t605 = ct{1060};
t606 = ct{1061};
t607 = ct{1062};
t608 = ct{1063};
t609 = ct{1064};
t61 = ct{1065};
t612 = ct{1066};
t613 = ct{1067};
t614 = ct{1068};
t615 = ct{1069};
t616 = ct{1070};
t617 = ct{1071};
t618 = ct{1072};
t619 = ct{1073};
t620 = ct{1074};
t621 = ct{1075};
t622 = ct{1076};
t623 = ct{1077};
t624 = ct{1078};
t626 = ct{1079};
t627 = ct{1080};
t628 = ct{1081};
t629 = ct{1082};
t63 = ct{1083};
t631 = ct{1084};
t632 = ct{1085};
t633 = ct{1086};
t634 = ct{1087};
t635 = ct{1088};
t637 = ct{1089};
t638 = ct{1090};
t639 = ct{1091};
t64 = ct{1092};
t640 = ct{1093};
t642 = ct{1094};
t643 = ct{1095};
t644 = ct{1096};
t646 = ct{1097};
t647 = ct{1098};
t648 = ct{1099};
t649 = ct{1100};
t650 = ct{1101};
t651 = ct{1102};
t652 = ct{1103};
t653 = ct{1104};
t654 = ct{1105};
t656 = ct{1106};
t657 = ct{1107};
t658 = ct{1108};
t660 = ct{1109};
t661 = ct{1110};
t662 = ct{1111};
t663 = ct{1112};
t664 = ct{1113};
t665 = ct{1114};
t666 = ct{1115};
t667 = ct{1116};
t669 = ct{1117};
t67 = ct{1118};
t670 = ct{1119};
t671 = ct{1120};
t673 = ct{1121};
t674 = ct{1122};
t675 = ct{1123};
t676 = ct{1124};
t677 = ct{1125};
t678 = ct{1126};
t679 = ct{1127};
t680 = ct{1128};
t681 = ct{1129};
t683 = ct{1130};
t684 = ct{1131};
t685 = ct{1132};
t686 = ct{1133};
t687 = ct{1134};
t688 = ct{1135};
t689 = ct{1136};
t69 = ct{1137};
t691 = ct{1138};
t692 = ct{1139};
t693 = ct{1140};
t694 = ct{1141};
t695 = ct{1142};
t696 = ct{1143};
t697 = ct{1144};
t698 = ct{1145};
t699 = ct{1146};
t7 = ct{1147};
t70 = ct{1148};
t700 = ct{1149};
t701 = ct{1150};
t702 = ct{1151};
t703 = ct{1152};
t704 = ct{1153};
t705 = ct{1154};
t706 = ct{1155};
t707 = ct{1156};
t708 = ct{1157};
t71 = ct{1158};
t712 = ct{1159};
t713 = ct{1160};
t714 = ct{1161};
t719 = ct{1162};
t72 = ct{1163};
t720 = ct{1164};
t721 = ct{1165};
t722 = ct{1166};
t723 = ct{1167};
t724 = ct{1168};
t725 = ct{1169};
t726 = ct{1170};
t728 = ct{1171};
t729 = ct{1172};
t73 = ct{1173};
t730 = ct{1174};
t731 = ct{1175};
t734 = ct{1176};
t735 = ct{1177};
t737 = ct{1178};
t74 = ct{1179};
t740 = ct{1180};
t743 = ct{1181};
t744 = ct{1182};
t745 = ct{1183};
t748 = ct{1184};
t749 = ct{1185};
t75 = ct{1186};
t750 = ct{1187};
t751 = ct{1188};
t753 = ct{1189};
t754 = ct{1190};
t755 = ct{1191};
t756 = ct{1192};
t757 = ct{1193};
t758 = ct{1194};
t759 = ct{1195};
t76 = ct{1196};
t760 = ct{1197};
t761 = ct{1198};
t762 = ct{1199};
t763 = ct{1200};
t764 = ct{1201};
t765 = ct{1202};
t766 = ct{1203};
t769 = ct{1204};
t77 = ct{1205};
t770 = ct{1206};
t771 = ct{1207};
t772 = ct{1208};
t773 = ct{1209};
t774 = ct{1210};
t775 = ct{1211};
t776 = ct{1212};
t777 = ct{1213};
t778 = ct{1214};
t779 = ct{1215};
t78 = ct{1216};
t780 = ct{1217};
t782 = ct{1218};
t783 = ct{1219};
t784 = ct{1220};
t785 = ct{1221};
t786 = ct{1222};
t787 = ct{1223};
t788 = ct{1224};
t79 = ct{1225};
t790 = ct{1226};
t791 = ct{1227};
t792 = ct{1228};
t794 = ct{1229};
t795 = ct{1230};
t796 = ct{1231};
t798 = ct{1232};
t799 = ct{1233};
t8 = ct{1234};
t80 = ct{1235};
t800 = ct{1236};
t801 = ct{1237};
t802 = ct{1238};
t803 = ct{1239};
t805 = ct{1240};
t806 = ct{1241};
t809 = ct{1242};
t81 = ct{1243};
t810 = ct{1244};
t811 = ct{1245};
t812 = ct{1246};
t813 = ct{1247};
t815 = ct{1248};
t816 = ct{1249};
t817 = ct{1250};
t818 = ct{1251};
t819 = ct{1252};
t82 = ct{1253};
t820 = ct{1254};
t821 = ct{1255};
t822 = ct{1256};
t827 = ct{1257};
t83 = ct{1258};
t831 = ct{1259};
t834 = ct{1260};
t835 = ct{1261};
t836 = ct{1262};
t837 = ct{1263};
t838 = ct{1264};
t839 = ct{1265};
t84 = ct{1266};
t840 = ct{1267};
t841 = ct{1268};
t842 = ct{1269};
t843 = ct{1270};
t845 = ct{1271};
t846 = ct{1272};
t847 = ct{1273};
t848 = ct{1274};
t849 = ct{1275};
t85 = ct{1276};
t850 = ct{1277};
t851 = ct{1278};
t852 = ct{1279};
t853 = ct{1280};
t854 = ct{1281};
t855 = ct{1282};
t856 = ct{1283};
t857 = ct{1284};
t859 = ct{1285};
t86 = ct{1286};
t860 = ct{1287};
t862 = ct{1288};
t863 = ct{1289};
t864 = ct{1290};
t866 = ct{1291};
t867 = ct{1292};
t868 = ct{1293};
t869 = ct{1294};
t87 = ct{1295};
t870 = ct{1296};
t871 = ct{1297};
t872 = ct{1298};
t873 = ct{1299};
t876 = ct{1300};
t877 = ct{1301};
t88 = ct{1302};
t880 = ct{1303};
t881 = ct{1304};
t882 = ct{1305};
t883 = ct{1306};
t886 = ct{1307};
t888 = ct{1308};
t889 = ct{1309};
t89 = ct{1310};
t890 = ct{1311};
t891 = ct{1312};
t892 = ct{1313};
t894 = ct{1314};
t898 = ct{1315};
t899 = ct{1316};
t9 = ct{1317};
t90 = ct{1318};
t900 = ct{1319};
t901 = ct{1320};
t902 = ct{1321};
t903 = ct{1322};
t904 = ct{1323};
t905 = ct{1324};
t908 = ct{1325};
t91 = ct{1326};
t911 = ct{1327};
t913 = ct{1328};
t915 = ct{1329};
t916 = ct{1330};
t918 = ct{1331};
t919 = ct{1332};
t92 = ct{1333};
t920 = ct{1334};
t922 = ct{1335};
t924 = ct{1336};
t925 = ct{1337};
t931 = ct{1338};
t934 = ct{1339};
t936 = ct{1340};
t937 = ct{1341};
t938 = ct{1342};
t94 = ct{1343};
t940 = ct{1344};
t941 = ct{1345};
t942 = ct{1346};
t944 = ct{1347};
t945 = ct{1348};
t946 = ct{1349};
t947 = ct{1350};
t948 = ct{1351};
t950 = ct{1352};
t952 = ct{1353};
t953 = ct{1354};
t954 = ct{1355};
t955 = ct{1356};
t958 = ct{1357};
t959 = ct{1358};
t965 = ct{1359};
t966 = ct{1360};
t968 = ct{1361};
t969 = ct{1362};
t97 = ct{1363};
t972 = ct{1364};
t973 = ct{1365};
t974 = ct{1366};
t975 = ct{1367};
t977 = ct{1368};
t978 = ct{1369};
t979 = ct{1370};
t982 = ct{1371};
t983 = ct{1372};
t987 = ct{1373};
t992 = ct{1374};
t994 = ct{1375};
t995 = ct{1376};
t997 = ct{1377};
t999 = ct{1378};
t2495 = t1629.*1.11e-3;
t2496 = t1630.*1.11e-3;
t2512 = t1628.*2.19e-3;
t2533 = t734+t1593+t1665;
t2535 = t1665.*7.299999999999999e-4;
t2536 = t1630.*1.12e-3;
t2542 = t1629.*8.8e-4;
t2547 = t2274.*1.8866e-1;
t2595 = t2274.*5.267999999999999e-2;
t2608 = t1629.*1.144e-2;
t2612 = t1791.*1.11e-3;
t2624 = t1630.*4.988e-2;
t2626 = t2271.*2.0e-4;
t2635 = t1840.*(-1.11e-3);
t2638 = t1819.*1.11e-3;
t2652 = t1840.*1.11e-3;
t2653 = t1791.*8.8e-4;
t2671 = t309+t315+t501+t502+t802+t1945;
t2677 = t1840.*(-8.8e-4);
t2679 = t1819.*8.8e-4;
t2684 = t1840.*8.8e-4;
t2688 = t329+t504+t505+t506+t805+t1951;
t2693 = t1791.*1.144e-2;
t2701 = t1840.*(-1.144e-2);
t2703 = t1819.*1.144e-2;
t2705 = -t8.*(t284+t287+t290-t329-t805-t1951);
t2706 = -t15.*(t284+t287+t290-t329-t805-t1951);
t2708 = t1840.*1.144e-2;
t2712 = t1999.*7.000000000000001e-5;
t2713 = t1999.*7.000000000000022e-5;
t2718 = t8.*(t284+t287+t290-t329-t805-t1951);
t2719 = t2024.*7.000000000000022e-5;
t2724 = t2024.*7.000000000000001e-5;
t2745 = t1999.*7.299999999999999e-4;
t2746 = t2024.*7.299999999999999e-4;
t2748 = t2056.*1.11e-3;
t2756 = t248+t701+t761+t769+t770+t924+t965;
t2757 = t2056.*1.12e-3;
t2766 = t2056.*4.988e-2;
t2769 = t913+t1791+t1879;
t2772 = t2149.*(t92-t663).*(-4.466636216449161e-20);
t2776 = t2149.*(t92-t663).*4.466636216449161e-20;
t2784 = t2373.*7.000000000000001e-5;
t2785 = t2373.*7.000000000000022e-5;
t2802 = t2373.*7.299999999999999e-4;
t2827 = t2149.*(t92-t663).*(-9.999999999999998e-6);
t2897 = t2149.*(t92-t663).*(-1.2e-4);
t2943 = t233+t544+t1057+t1098+t1592+t1628;
t3440 = t1739+t1788+t1789+t1926+t1973+t2135+t2169;
t3443 = t1708+t1904+t1916+t1965+t1966+t2027+t2031;
t3476 = t1747+t1768+t1895+t1947+t2004+t2194+t2252;
t797 = -t784;
t807 = -t763;
t814 = -t796;
t878 = dq6.*t860;
t884 = dq6.*t863;
t885 = dq6.*t864;
t887 = dq7.*t866;
t893 = -t852;
t895 = -t853;
t896 = dq6.*t870;
t897 = dq7.*t871;
t907 = t6.*t863;
t921 = t6.*t860;
t923 = t21.*t870;
t926 = t8.*t877;
t928 = dq5.*t13.*t860;
t930 = t15.*t877;
t933 = dq7.*t908;
t935 = dq5.*t13.*t863;
t939 = dq7.*t911;
t949 = -t882;
t961 = t21.*t860;
t963 = t21.*t863;
t964 = t21.*t864;
t967 = -t908;
t986 = t7.*t953;
t990 = t7.*t958;
t1011 = dq6.*t1003;
t1012 = dq6.*t1004;
t1013 = dq6.*t1007;
t1014 = dq6.*t1008;
t1015 = -t979;
t1027 = -t1003;
t1030 = -t1007;
t1041 = t618+t790;
t1051 = t8.*t1022;
t1054 = t15.*t1022;
t1060 = dq7.*t1052;
t1061 = dq7.*t1053;
t1063 = dq7.*t1055;
t1064 = dq7.*t1056;
t1207 = t616+t870;
t1242 = -t1185;
t1243 = -t1186;
t1244 = -t1188;
t1246 = -t1191;
t1290 = -t1237;
t1298 = t666+t864;
t1309 = -t1212;
t1318 = -t1215;
t1325 = -t1226;
t1330 = -t1273;
t1374 = t7.*t1206;
t1375 = t8.*t1206;
t1386 = t14.*t1206;
t1387 = t15.*t1206;
t1424 = -t1345;
t1515 = t7.*t1295;
t1516 = t8.*t1295;
t1526 = t14.*t1295;
t1528 = t15.*t1295;
t1529 = -t8.*(t621-t864);
t1532 = -t15.*(t621-t864);
t1583 = dq7.*t1527;
t1588 = dq7.*t1531;
t1594 = t7.*t1527;
t1595 = t7.*t1531;
t1601 = t8.*(t621-t864);
t1608 = t22.*t1527;
t1610 = t22.*t1531;
t1614 = dq6.*t14.*t1527;
t1621 = dq6.*t14.*t1531;
t1626 = dq7.*t1604;
t1633 = t7.*t1604;
t1647 = t22.*t1604;
t1649 = t722+t1004;
t1650 = t7.*t1618;
t1652 = t7.*t1623;
t1654 = t724+t1008;
t1657 = t8.*t1625;
t1660 = dq6.*t14.*t1604;
t1682 = -t1669;
t1686 = t788+t1009;
t1693 = -t1677;
t1695 = t763.*2.37e-3;
t1697 = t649+t1056;
t1705 = -t1689;
t1719 = t763.*2.75e-2;
t1720 = -t1703;
t1722 = -t1709;
t1726 = -t1712;
t1730 = t737+t1053;
t1731 = -t1714;
t1752 = -t1724;
t1761 = -t1728;
t1763 = -t1733;
t1766 = -t1742;
t1769 = t775.*5.000000000000001e-5;
t1779 = t871+t968;
t1780 = -t1764;
t1782 = -t1767;
t1792 = t8.*t1738;
t1793 = -t1781;
t1795 = t15.*t1738;
t1799 = t6.*t1770;
t1801 = t13.*t1770;
t1802 = t7.*t1749;
t1805 = t14.*t1749;
t1811 = t866+t1001;
t1813 = -t1794;
t1815 = t849.*2.37e-3;
t1817 = -t1808;
t1835 = t849.*2.75e-2;
t1839 = t850.*4.9e-4;
t1841 = t872.*2.37e-3;
t1851 = -t1838;
t1856 = t872.*2.75e-2;
t1862 = t853.*2.019e-2;
t1864 = t109+t126+t314+t341+t954;
t1867 = t877.*2.75e-2;
t1869 = t852.*5.000000000000001e-5;
t1871 = t7.*t1823;
t1873 = t14.*t1823;
t1874 = t8.*t1830;
t1876 = t15.*t1830;
t1880 = -t1842;
t1884 = t904.*5.000000000000001e-5;
t1903 = t6.*t1855;
t1907 = t13.*t1855;
t1909 = t7.*t1860;
t1913 = t14.*t1860;
t1914 = t7.*t1865;
t1919 = t14.*t1865;
t1957 = t853.*1.9738e-1;
t1969 = t979.*3.466000000000001e-2;
t1972 = t1017.*(-3.466000000000001e-2);
t1985 = t978.*2.324e-2;
t2019 = t1045.*(-3.466000000000001e-2);
t2022 = -t2012;
t2033 = t1045.*3.466000000000001e-2;
t2047 = -t2025;
t2057 = -t2040;
t2083 = -t2062;
t2086 = -t2063;
t2093 = -t2068;
t2105 = -t2079;
t2109 = (t8.*(t92-t663)+t15.*(t621-t864)).^2;
t2111 = -t2084;
t2114 = -t2087;
t2120 = -t2092;
t2125 = -t2106;
t2126 = -t2107;
t2130 = -t2118;
t2133 = -t2122;
t2134 = -t2124;
t2141 = -t2131;
t2146 = -t2137;
t2164 = t140+t147+t156+t669+t1221;
t2165 = t157+t162+t168+t744+t1120;
t2179 = t6.*t2147;
t2180 = t7.*t2147;
t2181 = t6.*t2148;
t2182 = t13.*t2147;
t2183 = t7.*t2148;
t2184 = t14.*t2147;
t2186 = t13.*t2148;
t2187 = t14.*t2148;
t2192 = -t2159;
t2193 = -t2173;
t2197 = -t2178;
t2202 = t2159.*(2.0./5.0);
t2204 = -t2172;
t2209 = t8.*t2177;
t2211 = t15.*t2177;
t2212 = t6.*t2163;
t2214 = t7.*t2163;
t2217 = t13.*t2163;
t2219 = t14.*t2163;
t2226 = -t2190;
t2251 = dq7.*t15.*(t621-t864).*(-3.466000000000001e-2);
t2262 = t7.*t2196;
t2263 = t8.*t2196;
t2266 = t14.*t2196;
t2267 = t15.*t2196;
t2277 = -t2235;
t2292 = -t2244;
t2304 = t1662.*(-2.324e-2);
t2306 = -t2275;
t2310 = t15.*t22.*(t621-t864).*(-2.324e-2);
t2313 = t1662.*2.324e-2;
t2314 = t7.*t1662.*(-3.466000000000001e-2);
t2321 = t1680.*(-3.466000000000001e-2);
t2327 = t1680.*3.466000000000001e-2;
t2350 = t572.*t2147;
t2351 = t572.*t2148;
t2356 = t573.*t2177;
t2369 = t604.*t2163;
t2370 = t573.*t2196;
t2376 = t1055+t1820;
t2382 = t1052+t1849;
t2385 = t1859.*(-3.466000000000001e-2);
t2412 = t831.*t2148;
t2418 = -t2411;
t2424 = -t2407;
t2426 = -t2419;
t2441 = -t2437;
t2442 = -t2438;
t2443 = t1842.*4.466636216449161e-20;
t2444 = t1843.*4.466636216449161e-20;
t2447 = t1846.*4.466636216449161e-20;
t2451 = -t2448;
t2464 = -t2454;
t2471 = -t2461;
t2473 = -t2465;
t2481 = t2159.*1.8866e-1;
t2492 = t2157.*2.37e-3;
t2502 = -t2489;
t2506 = -t2495;
t2508 = -t2496;
t2509 = t2157.*2.75e-2;
t2518 = t2159.*5.267999999999999e-2;
t2525 = t2172.*4.9e-4;
t2526 = t2160.*5.000000000000001e-5;
t2527 = t1066.*t2147;
t2528 = t1066.*t2148;
t2529 = t1040.*t2163;
t2532 = t2156.*2.0e-4;
t2538 = t2170.*2.019e-2;
t2539 = t2230.*2.37e-3;
t2548 = -t2535;
t2549 = -t2536;
t2550 = t2247.*2.37e-3;
t2551 = -t2542;
t2558 = t2230.*2.75e-2;
t2572 = t2247.*2.75e-2;
t2582 = t2235.*5.000000000000001e-5;
t2586 = t1070.*t2196;
t2594 = t2244.*5.000000000000001e-5;
t2606 = t2170.*1.9738e-1;
t2607 = -t2595;
t2618 = t1295.*t2147;
t2619 = t1295.*t2148;
t2620 = t1206.*t2163;
t2623 = -t2608;
t2634 = t317+t318+t320+t322+t810+t1950;
t2636 = -t2624;
t2639 = -t2626;
t2649 = -t2177.*(t621-t864);
t2659 = t308+t310+t313+t316+t822+t1949;
t2668 = -t2196.*(t621-t864);
t2672 = t286+t289+t294+t519+t820+t1944;
t2673 = t1842.*1.0e-5;
t2674 = t1843.*1.0e-5;
t2675 = t1846.*1.0e-5;
t2676 = t331+t507+t508+t509+t760+t1953;
t2687 = t693+t695+t713+t1050+t1209;
t2690 = t8.*t2671;
t2691 = t15.*t2671;
t2707 = t671+t703+t764+t1074+t1211;
t2709 = t1842.*2.840000000000012e-3;
t2710 = t1843.*2.840000000000012e-3;
t2711 = t1846.*2.840000000000012e-3;
t2720 = t638+t775+t1227+t1800;
t2722 = t638+t773+t775+t1110+t1227;
t2725 = -t2719;
t2731 = -t2724;
t2734 = t697+t699+t783+t1213+t1229;
t2735 = t705+t745+t766+t1123+t1219;
t2755 = -t2746;
t2758 = t2190.*7.000000000000001e-5;
t2760 = t2190.*4.999999999999997e-5;
t2761 = t2190.*2.23e-3;
t2762 = t2275.*7.000000000000001e-5;
t2765 = t2407.*4.466636216449161e-20;
t2768 = t2275.*4.999999999999997e-5;
t2770 = t2275.*2.23e-3;
t2771 = t2201.*3.844e-2;
t2774 = t2201.*1.12e-3;
t2775 = t2201.*8.8e-4;
t2778 = t2345.*7.000000000000001e-5;
t2779 = t2345.*7.000000000000022e-5;
t2786 = t2345.*7.299999999999999e-4;
t2787 = t2360.*1.11e-3;
t2788 = t2147.*t2148;
t2805 = t2360.*1.12e-3;
t2822 = t719+t886+t1133+t2185;
t2830 = t2360.*4.988e-2;
t2833 = t2431.*(-1.11e-3);
t2834 = t2414.*1.11e-3;
t2844 = t2407.*1.0e-5;
t2854 = t674+t944+t1222+t2188;
t2869 = t2431.*(-8.8e-4);
t2870 = t2414.*8.8e-4;
t2891 = t2407.*2.840000000000012e-3;
t2898 = t2431.*(-1.144e-2);
t2899 = t2414.*1.144e-2;
t2924 = t2177.*(t621-t864).*(-4.000000000000028e-5);
t2927 = t2177.*(t621-t864).*4.000000000000028e-5;
t2929 = t2196.*(t621-t864).*(-4.000000000000028e-5);
t2932 = t2177.*(t621-t864).*(-5.0e-5);
t2944 = t2177.*(t621-t864).*(-2.81e-3);
t2946 = t2196.*(t621-t864).*(-5.0e-5);
t2952 = t2196.*(t621-t864).*(-2.81e-3);
t2963 = t361+t364+t368+t373+t378+t489+t749+t1099+t2274;
t2971 = t386+t389+t393+t402+t407+t472+t798+t1100+t2305;
t2972 = t395+t397+t399+t411+t412+t473+t801+t1239+t2247;
t3372 = t771+t772+t925+t1999+t2055+t2345+t2373;
t3669 = t2050+t2143+t2153+t2347+t2364+t2417+t2434+t2457+t2491;
t927 = t6.*t878;
t932 = t6.*t884;
t943 = -t878;
t951 = -t884;
t957 = -t896;
t976 = -t921;
t980 = -t926;
t985 = -t933;
t988 = -t939;
t1033 = -t1011;
t1035 = -t1012;
t1059 = dq7.*t1051;
t1062 = dq7.*t1054;
t1077 = t7.*t1041;
t1081 = t14.*t1041;
t1091 = -t1060;
t1092 = -t1061;
t1329 = t1207.^2;
t1471 = dq6.*t1374;
t1472 = dq7.*t1375;
t1473 = dq7.*t8.*t1207;
t1487 = dq6.*t1386;
t1488 = dq7.*t1387;
t1489 = dq7.*t15.*t1207;
t1530 = -t1386;
t1557 = t21.*t1374;
t1564 = t21.*t1386;
t1578 = dq6.*t1515;
t1579 = dq7.*t1516;
t1582 = dq6.*t1526;
t1584 = dq7.*t1528;
t1585 = dq7.*t1529;
t1589 = dq7.*t1532;
t1598 = -t1526;
t1606 = t21.*t1515;
t1607 = t21.*t1526;
t1609 = t22.*t1529;
t1611 = t22.*t1532;
t1613 = t7.*t1583;
t1615 = t7.*t1588;
t1658 = t7.*t1626;
t1681 = t723+t1027;
t1685 = t728+t1030;
t1711 = -t1695;
t1746 = -t1719;
t1776 = t907+t915;
t1803 = dq7.*t1792;
t1806 = dq7.*t1795;
t1844 = -t8.*(t921+t14.*(t86-t652));
t1847 = -t15.*(t921+t14.*(t86-t652));
t1872 = -t1862;
t1875 = t878.*4.9e-4;
t1878 = t896.*4.9e-4;
t1882 = -t1869;
t1886 = dq7.*t8.*(t921+t14.*(t86-t652));
t1888 = dq7.*t15.*(t921+t14.*(t86-t652));
t1890 = t884.*2.019e-2;
t1891 = t885.*2.019e-2;
t1902 = t887.*3.466000000000001e-2;
t1912 = t6.*t1864;
t1915 = -t1876;
t1918 = t13.*t1864;
t1921 = t963.*4.9e-4;
t1922 = t964.*4.9e-4;
t1927 = t897.*2.324e-2;
t1933 = t961.*2.019e-2;
t1936 = t923.*2.019e-2;
t1942 = t933.*3.466000000000001e-2;
t1959 = t939.*2.324e-2;
t1970 = t1012.*4.9e-4;
t1974 = t1014.*4.9e-4;
t1975 = t884.*1.9738e-1;
t1976 = t885.*1.9738e-1;
t1984 = t1011.*2.019e-2;
t1986 = t1013.*2.019e-2;
t1988 = t923.*1.9738e-1;
